simulink model "simulator_prototype_v2"  (R2021b)
(part 6 of 12)

t2408 = ct{941};
t2409 = ct{942};
t241 = ct{943};
t2410 = ct{944};
t2411 = ct{945};
t2412 = ct{946};
t2413 = ct{947};
t2414 = ct{948};
t2416 = ct{949};
t2417 = ct{950};
t2418 = ct{951};
t2419 = ct{952};
t2421 = ct{953};
t2422 = ct{954};
t2423 = ct{955};
t2425 = ct{956};
t2426 = ct{957};
t2427 = ct{958};
t2431 = ct{959};
t2432 = ct{960};
t2433 = ct{961};
t2434 = ct{962};
t2438 = ct{963};
t244 = ct{964};
t2440 = ct{965};
t2441 = ct{966};
t2444 = ct{967};
t2446 = ct{968};
t2447 = ct{969};
t2448 = ct{970};
t2449 = ct{971};
t2450 = ct{972};
t2451 = ct{973};
t2455 = ct{974};
t2457 = ct{975};
t2458 = ct{976};
t2459 = ct{977};
t2460 = ct{978};
t2461 = ct{979};
t2463 = ct{980};
t2465 = ct{981};
t2466 = ct{982};
t2467 = ct{983};
t2468 = ct{984};
t2470 = ct{985};
t2471 = ct{986};
t2472 = ct{987};
t2473 = ct{988};
t2474 = ct{989};
t2476 = ct{990};
t2477 = ct{991};
t2478 = ct{992};
t2479 = ct{993};
t2480 = ct{994};
t2481 = ct{995};
t2484 = ct{996};
t2485 = ct{997};
t2487 = ct{998};
t2488 = ct{999};
t2489 = ct{1000};
t2490 = ct{1001};
t2491 = ct{1002};
t2492 = ct{1003};
t2493 = ct{1004};
t2494 = ct{1005};
t2496 = ct{1006};
t2497 = ct{1007};
t2498 = ct{1008};
t2499 = ct{1009};
t25 = ct{1010};
t2500 = ct{1011};
t2502 = ct{1012};
t2503 = ct{1013};
t2504 = ct{1014};
t2505 = ct{1015};
t2507 = ct{1016};
t2508 = ct{1017};
t2509 = ct{1018};
t2510 = ct{1019};
t2511 = ct{1020};
t2512 = ct{1021};
t2514 = ct{1022};
t2515 = ct{1023};
t2516 = ct{1024};
t2517 = ct{1025};
t2520 = ct{1026};
t2521 = ct{1027};
t2522 = ct{1028};
t2524 = ct{1029};
t2525 = ct{1030};
t2526 = ct{1031};
t2527 = ct{1032};
t2528 = ct{1033};
t2529 = ct{1034};
t2530 = ct{1035};
t2531 = ct{1036};
t2532 = ct{1037};
t2534 = ct{1038};
t2535 = ct{1039};
t2539 = ct{1040};
t2541 = ct{1041};
t2542 = ct{1042};
t2548 = ct{1043};
t2549 = ct{1044};
t2550 = ct{1045};
t2552 = ct{1046};
t2554 = ct{1047};
t2555 = ct{1048};
t2556 = ct{1049};
t2557 = ct{1050};
t2558 = ct{1051};
t2559 = ct{1052};
t2560 = ct{1053};
t2564 = ct{1054};
t2565 = ct{1055};
t2566 = ct{1056};
t2569 = ct{1057};
t257 = ct{1058};
t2570 = ct{1059};
t2571 = ct{1060};
t2572 = ct{1061};
t2575 = ct{1062};
t2577 = ct{1063};
t2578 = ct{1064};
t2579 = ct{1065};
t2580 = ct{1066};
t2581 = ct{1067};
t2582 = ct{1068};
t2583 = ct{1069};
t2584 = ct{1070};
t2585 = ct{1071};
t2586 = ct{1072};
t2587 = ct{1073};
t2589 = ct{1074};
t259 = ct{1075};
t2595 = ct{1076};
t2597 = ct{1077};
t2599 = ct{1078};
t26 = ct{1079};
t2600 = ct{1080};
t2601 = ct{1081};
t2603 = ct{1082};
t2604 = ct{1083};
t2605 = ct{1084};
t2606 = ct{1085};
t261 = ct{1086};
t2610 = ct{1087};
t2611 = ct{1088};
t2612 = ct{1089};
t2613 = ct{1090};
t2614 = ct{1091};
t2616 = ct{1092};
t2618 = ct{1093};
t2619 = ct{1094};
t262 = ct{1095};
t2620 = ct{1096};
t2621 = ct{1097};
t2622 = ct{1098};
t2623 = ct{1099};
t2624 = ct{1100};
t2626 = ct{1101};
t2627 = ct{1102};
t2628 = ct{1103};
t2629 = ct{1104};
t2630 = ct{1105};
t2632 = ct{1106};
t2633 = ct{1107};
t2634 = ct{1108};
t2635 = ct{1109};
t2638 = ct{1110};
t264 = ct{1111};
t2640 = ct{1112};
t2641 = ct{1113};
t2642 = ct{1114};
t2643 = ct{1115};
t2644 = ct{1116};
t2645 = ct{1117};
t2646 = ct{1118};
t2647 = ct{1119};
t2648 = ct{1120};
t2649 = ct{1121};
t2650 = ct{1122};
t2651 = ct{1123};
t2652 = ct{1124};
t2653 = ct{1125};
t2654 = ct{1126};
t2655 = ct{1127};
t2657 = ct{1128};
t2658 = ct{1129};
t2659 = ct{1130};
t2660 = ct{1131};
t2661 = ct{1132};
t2662 = ct{1133};
t2664 = ct{1134};
t2665 = ct{1135};
t2666 = ct{1136};
t2667 = ct{1137};
t2668 = ct{1138};
t2670 = ct{1139};
t2671 = ct{1140};
t2672 = ct{1141};
t2673 = ct{1142};
t2674 = ct{1143};
t2675 = ct{1144};
t2676 = ct{1145};
t2678 = ct{1146};
t2679 = ct{1147};
t2680 = ct{1148};
t2681 = ct{1149};
t2682 = ct{1150};
t2683 = ct{1151};
t2684 = ct{1152};
t2685 = ct{1153};
t2686 = ct{1154};
t2687 = ct{1155};
t2688 = ct{1156};
t2691 = ct{1157};
t2692 = ct{1158};
t2694 = ct{1159};
t2695 = ct{1160};
t2697 = ct{1161};
t2698 = ct{1162};
t2699 = ct{1163};
t27 = ct{1164};
t2701 = ct{1165};
t2703 = ct{1166};
t2707 = ct{1167};
t2708 = ct{1168};
t2709 = ct{1169};
t271 = ct{1170};
t2710 = ct{1171};
t2711 = ct{1172};
t2712 = ct{1173};
t2714 = ct{1174};
t2716 = ct{1175};
t2732 = ct{1176};
t2733 = ct{1177};
t2735 = ct{1178};
t2736 = ct{1179};
t2737 = ct{1180};
t2738 = ct{1181};
t2739 = ct{1182};
t2740 = ct{1183};
t2742 = ct{1184};
t2743 = ct{1185};
t2744 = ct{1186};
t2745 = ct{1187};
t2748 = ct{1188};
t2749 = ct{1189};
t2750 = ct{1190};
t2753 = ct{1191};
t2754 = ct{1192};
t2757 = ct{1193};
t2759 = ct{1194};
t276 = ct{1195};
t2762 = ct{1196};
t2765 = ct{1197};
t2769 = ct{1198};
t2771 = ct{1199};
t2773 = ct{1200};
t2774 = ct{1201};
t2775 = ct{1202};
t2777 = ct{1203};
t2778 = ct{1204};
t2779 = ct{1205};
t2781 = ct{1206};
t2785 = ct{1207};
t2786 = ct{1208};
t2787 = ct{1209};
t2788 = ct{1210};
t279 = ct{1211};
t2790 = ct{1212};
t2791 = ct{1213};
t2792 = ct{1214};
t2793 = ct{1215};
t2795 = ct{1216};
t2796 = ct{1217};
t2797 = ct{1218};
t2798 = ct{1219};
t2799 = ct{1220};
t28 = ct{1221};
t280 = ct{1222};
t2801 = ct{1223};
t2802 = ct{1224};
t2803 = ct{1225};
t2804 = ct{1226};
t2805 = ct{1227};
t2806 = ct{1228};
t2807 = ct{1229};
t2808 = ct{1230};
t2810 = ct{1231};
t2811 = ct{1232};
t2812 = ct{1233};
t2813 = ct{1234};
t2814 = ct{1235};
t2817 = ct{1236};
t2818 = ct{1237};
t2819 = ct{1238};
t2820 = ct{1239};
t2823 = ct{1240};
t2825 = ct{1241};
t2831 = ct{1242};
t2832 = ct{1243};
t2835 = ct{1244};
t2838 = ct{1245};
t2850 = ct{1246};
t2851 = ct{1247};
t2857 = ct{1248};
t2858 = ct{1249};
t2859 = ct{1250};
t286 = ct{1251};
t2865 = ct{1252};
t2867 = ct{1253};
t2868 = ct{1254};
t2870 = ct{1255};
t2875 = ct{1256};
t2883 = ct{1257};
t2884 = ct{1258};
t2886 = ct{1259};
t2890 = ct{1260};
t2893 = ct{1261};
t2894 = ct{1262};
t2895 = ct{1263};
t2898 = ct{1264};
t2900 = ct{1265};
t2901 = ct{1266};
t2903 = ct{1267};
t2905 = ct{1268};
t2909 = ct{1269};
t2911 = ct{1270};
t2914 = ct{1271};
t2917 = ct{1272};
t2918 = ct{1273};
t2919 = ct{1274};
t2920 = ct{1275};
t2922 = ct{1276};
t2923 = ct{1277};
t2925 = ct{1278};
t2926 = ct{1279};
t2927 = ct{1280};
t293 = ct{1281};
t2930 = ct{1282};
t2931 = ct{1283};
t2933 = ct{1284};
t2935 = ct{1285};
t2937 = ct{1286};
t2941 = ct{1287};
t2942 = ct{1288};
t2943 = ct{1289};
t2944 = ct{1290};
t2947 = ct{1291};
t2948 = ct{1292};
t2949 = ct{1293};
t2950 = ct{1294};
t2951 = ct{1295};
t2952 = ct{1296};
t2955 = ct{1297};
t2956 = ct{1298};
t2961 = ct{1299};
t2962 = ct{1300};
t2963 = ct{1301};
t2964 = ct{1302};
t2965 = ct{1303};
t2966 = ct{1304};
t2969 = ct{1305};
t2970 = ct{1306};
t2971 = ct{1307};
t2972 = ct{1308};
t2973 = ct{1309};
t2975 = ct{1310};
t2976 = ct{1311};
t2977 = ct{1312};
t2978 = ct{1313};
t2979 = ct{1314};
t2981 = ct{1315};
t2982 = ct{1316};
t2983 = ct{1317};
t2984 = ct{1318};
t2986 = ct{1319};
t2987 = ct{1320};
t2990 = ct{1321};
t2991 = ct{1322};
t2993 = ct{1323};
t2999 = ct{1324};
t3 = ct{1325};
t30 = ct{1326};
t3000 = ct{1327};
t3004 = ct{1328};
t3005 = ct{1329};
t3008 = ct{1330};
t3010 = ct{1331};
t3011 = ct{1332};
t3012 = ct{1333};
t3015 = ct{1334};
t3017 = ct{1335};
t3018 = ct{1336};
t3019 = ct{1337};
t3022 = ct{1338};
t3023 = ct{1339};
t3026 = ct{1340};
t3027 = ct{1341};
t3029 = ct{1342};
t3030 = ct{1343};
t3036 = ct{1344};
t3037 = ct{1345};
t3042 = ct{1346};
t3043 = ct{1347};
t3044 = ct{1348};
t3045 = ct{1349};
t3049 = ct{1350};
t305 = ct{1351};
t3050 = ct{1352};
t3051 = ct{1353};
t3054 = ct{1354};
t3055 = ct{1355};
t3056 = ct{1356};
t306 = ct{1357};
t3064 = ct{1358};
t3065 = ct{1359};
t3066 = ct{1360};
t3067 = ct{1361};
t3068 = ct{1362};
t3069 = ct{1363};
t3072 = ct{1364};
t3074 = ct{1365};
t3075 = ct{1366};
t3076 = ct{1367};
t3077 = ct{1368};
t3079 = ct{1369};
t308 = ct{1370};
t3080 = ct{1371};
t3081 = ct{1372};
t3082 = ct{1373};
t3083 = ct{1374};
t3085 = ct{1375};
t3086 = ct{1376};
t3087 = ct{1377};
t3088 = ct{1378};
t31 = ct{1379};
t310 = ct{1380};
t3119 = ct{1381};
t312 = ct{1382};
t3120 = ct{1383};
t3129 = ct{1384};
t313 = ct{1385};
t314 = ct{1386};
t3153 = ct{1387};
t3154 = ct{1388};
t3159 = ct{1389};
t316 = ct{1390};
t3165 = ct{1391};
t3171 = ct{1392};
t3172 = ct{1393};
t319 = ct{1394};
t32 = ct{1395};
t321 = ct{1396};
t322 = ct{1397};
t326 = ct{1398};
t328 = ct{1399};
t329 = ct{1400};
t33 = ct{1401};
t330 = ct{1402};
t3306 = ct{1403};
t3308 = ct{1404};
t331 = ct{1405};
t3312 = ct{1406};
t3317 = ct{1407};
t332 = ct{1408};
t333 = ct{1409};
t335 = ct{1410};
t336 = ct{1411};
t3371 = ct{1412};
t3372 = ct{1413};
t3374 = ct{1414};
t3375 = ct{1415};
t338 = ct{1416};
t3380 = ct{1417};
t3381 = ct{1418};
t339 = ct{1419};
t34 = ct{1420};
t341 = ct{1421};
t343 = ct{1422};
t3457 = ct{1423};
t3458 = ct{1424};
t346 = ct{1425};
t347 = ct{1426};
t35 = ct{1427};
t350 = ct{1428};
t3504 = ct{1429};
t351 = ct{1430};
t3514 = ct{1431};
t352 = ct{1432};
t354 = ct{1433};
t356 = ct{1434};
t358 = ct{1435};
t359 = ct{1436};
t36 = ct{1437};
t360 = ct{1438};
t3617 = ct{1439};
t362 = ct{1440};
t3628 = ct{1441};
t363 = ct{1442};
t364 = ct{1443};
t365 = ct{1444};
t366 = ct{1445};
t369 = ct{1446};
t370 = ct{1447};
t371 = ct{1448};
t372 = ct{1449};
t3742 = ct{1450};
t378 = ct{1451};
t3780 = ct{1452};
t3781 = ct{1453};
t38 = ct{1454};
t380 = ct{1455};
t3808 = ct{1456};
t3809 = ct{1457};
t382 = ct{1458};
t3846 = ct{1459};
t3847 = ct{1460};
t3848 = ct{1461};
t3849 = ct{1462};
t3850 = ct{1463};
t387 = ct{1464};
t39 = ct{1465};
t393 = ct{1466};
t3940 = ct{1467};
t3961 = ct{1468};
t3999 = ct{1469};
t4 = ct{1470};
t410 = ct{1471};
t4109 = ct{1472};
t4115 = ct{1473};
t4116 = ct{1474};
t42 = ct{1475};
t4220 = ct{1476};
t4270 = ct{1477};
t428 = ct{1478};
t4280 = ct{1479};
t4282 = ct{1480};
t4289 = ct{1481};
t429 = ct{1482};
t4293 = ct{1483};
t4295 = ct{1484};
t43 = ct{1485};
t4421 = ct{1486};
t4500 = ct{1487};
t46 = ct{1488};
t461 = ct{1489};
t4620 = ct{1490};
t4644 = ct{1491};
t4655 = ct{1492};
t47 = ct{1493};
t4704 = ct{1494};
t4705 = ct{1495};
t473 = ct{1496};
t474 = ct{1497};
t4789 = ct{1498};
t4792 = ct{1499};
t480 = ct{1500};
t4974 = ct{1501};
t4976 = ct{1502};
t498 = ct{1503};
t4985 = ct{1504};
t5 = ct{1505};
t50 = ct{1506};
t503 = ct{1507};
t504 = ct{1508};
t506 = ct{1509};
t510 = ct{1510};
t514 = ct{1511};
t516 = ct{1512};
t521 = ct{1513};
t522 = ct{1514};
t523 = ct{1515};
t524 = ct{1516};
t5240 = ct{1517};
t5243 = ct{1518};
t528 = ct{1519};
t530 = ct{1520};
t5317 = ct{1521};
t535 = ct{1522};
t538 = ct{1523};
t5381 = ct{1524};
t539 = ct{1525};
t542 = ct{1526};
t543 = ct{1527};
t549 = ct{1528};
t56 = ct{1529};
t562 = ct{1530};
t563 = ct{1531};
t564 = ct{1532};
t573 = ct{1533};
t575 = ct{1534};
t577 = ct{1535};
t579 = ct{1536};
t58 = ct{1537};
t580 = ct{1538};
t581 = ct{1539};
t587 = ct{1540};
t59 = ct{1541};
t593 = ct{1542};
t594 = ct{1543};
t598 = ct{1544};
t6 = ct{1545};
t60 = ct{1546};
t610 = ct{1547};
t611 = ct{1548};
t612 = ct{1549};
t614 = ct{1550};
t615 = ct{1551};
t616 = ct{1552};
t623 = ct{1553};
t624 = ct{1554};
t628 = ct{1555};
t635 = ct{1556};
t636 = ct{1557};
t638 = ct{1558};
t640 = ct{1559};
t641 = ct{1560};
t642 = ct{1561};
t643 = ct{1562};
t644 = ct{1563};
t645 = ct{1564};
t646 = ct{1565};
t648 = ct{1566};
t649 = ct{1567};
t654 = ct{1568};
t655 = ct{1569};
t656 = ct{1570};
t657 = ct{1571};
t658 = ct{1572};
t659 = ct{1573};
t660 = ct{1574};
t662 = ct{1575};
t663 = ct{1576};
t664 = ct{1577};
t665 = ct{1578};
t666 = ct{1579};
t667 = ct{1580};
t668 = ct{1581};
t669 = ct{1582};
t67 = ct{1583};
t670 = ct{1584};
t672 = ct{1585};
t673 = ct{1586};
t674 = ct{1587};
t675 = ct{1588};
t676 = ct{1589};
t677 = ct{1590};
t678 = ct{1591};
t679 = ct{1592};
t68 = ct{1593};
t680 = ct{1594};
t681 = ct{1595};
t682 = ct{1596};
t683 = ct{1597};
t684 = ct{1598};
t685 = ct{1599};
t686 = ct{1600};
t687 = ct{1601};
t689 = ct{1602};
t691 = ct{1603};
t692 = ct{1604};
t693 = ct{1605};
t694 = ct{1606};
t696 = ct{1607};
t698 = ct{1608};
t7 = ct{1609};
t70 = ct{1610};
t702 = ct{1611};
t704 = ct{1612};
t705 = ct{1613};
t707 = ct{1614};
t708 = ct{1615};
t71 = ct{1616};
t710 = ct{1617};
t711 = ct{1618};
t712 = ct{1619};
t713 = ct{1620};
t714 = ct{1621};
t715 = ct{1622};
t716 = ct{1623};
t717 = ct{1624};
t718 = ct{1625};
t719 = ct{1626};
t720 = ct{1627};
t721 = ct{1628};
t722 = ct{1629};
t723 = ct{1630};
t724 = ct{1631};
t725 = ct{1632};
t726 = ct{1633};
t728 = ct{1634};
t73 = ct{1635};
t733 = ct{1636};
t736 = ct{1637};
t738 = ct{1638};
t740 = ct{1639};
t741 = ct{1640};
t742 = ct{1641};
t743 = ct{1642};
t744 = ct{1643};
t745 = ct{1644};
t746 = ct{1645};
t747 = ct{1646};
t749 = ct{1647};
t750 = ct{1648};
t751 = ct{1649};
t755 = ct{1650};
t756 = ct{1651};
t757 = ct{1652};
t758 = ct{1653};
t759 = ct{1654};
t76 = ct{1655};
t762 = ct{1656};
t763 = ct{1657};
t764 = ct{1658};
t766 = ct{1659};
t767 = ct{1660};
t768 = ct{1661};
t770 = ct{1662};
t771 = ct{1663};
t772 = ct{1664};
t773 = ct{1665};
t774 = ct{1666};
t775 = ct{1667};
t776 = ct{1668};
t777 = ct{1669};
t778 = ct{1670};
t781 = ct{1671};
t782 = ct{1672};
t783 = ct{1673};
t784 = ct{1674};
t785 = ct{1675};
t786 = ct{1676};
t787 = ct{1677};
t789 = ct{1678};
t790 = ct{1679};
t791 = ct{1680};
t792 = ct{1681};
t793 = ct{1682};
t794 = ct{1683};
t796 = ct{1684};
t797 = ct{1685};
t798 = ct{1686};
t799 = ct{1687};
t800 = ct{1688};
t801 = ct{1689};
t802 = ct{1690};
t806 = ct{1691};
t807 = ct{1692};
t808 = ct{1693};
t809 = ct{1694};
t812 = ct{1695};
t813 = ct{1696};
t816 = ct{1697};
t817 = ct{1698};
t818 = ct{1699};
t819 = ct{1700};
t820 = ct{1701};
t821 = ct{1702};
t822 = ct{1703};
t823 = ct{1704};
t824 = ct{1705};
t825 = ct{1706};
t826 = ct{1707};
t827 = ct{1708};
t828 = ct{1709};
t829 = ct{1710};
t830 = ct{1711};
t831 = ct{1712};
t832 = ct{1713};
t833 = ct{1714};
t850 = ct{1715};
t855 = ct{1716};
t856 = ct{1717};
t874 = ct{1718};
t878 = ct{1719};
t89 = ct{1720};
t893 = ct{1721};
t90 = ct{1722};
t91 = ct{1723};
t911 = ct{1724};
t92 = ct{1725};
t925 = ct{1726};
t926 = ct{1727};
t936 = ct{1728};
t937 = ct{1729};
t940 = ct{1730};
t941 = ct{1731};
t942 = ct{1732};
t944 = ct{1733};
t945 = ct{1734};
t948 = ct{1735};
t949 = ct{1736};
t950 = ct{1737};
t951 = ct{1738};
t959 = ct{1739};
t961 = ct{1740};
t965 = ct{1741};
t966 = ct{1742};
t97 = ct{1743};
t974 = ct{1744};
t978 = ct{1745};
t983 = ct{1746};
t987 = ct{1747};
t989 = ct{1748};
t99 = ct{1749};
t990 = ct{1750};
t991 = ct{1751};
t992 = ct{1752};
t993 = ct{1753};
t995 = ct{1754};
t996 = ct{1755};
t998 = ct{1756};
t3121 = t35.*t991.*t2699.*2.196325630278387e-1;
t3122 = t36.*t991.*t2699.*2.196325630278387e-1;
t3126 = t50.*t202.*t2981.*9.543032792050485e-17;
t3130 = (t2307.*t2363)./1.0e+8;
t3131 = (t2297.*t2388)./1.0e+8;
t3133 = t2363.*t2554;
t3136 = t38.*t1022.*(t855-t878).*(-2.196325630278387e-1);
t3137 = t39.*t1022.*(t855-t878).*(-2.196325630278387e-1);
t3139 = (t2297.*t2419)./1.0e+8;
t3140 = (t2338.*t2363)./1.0e+8;
t3143 = t35.*t991.*t2699.*1.122398993609262e-1;
t3144 = t36.*t991.*t2699.*1.122398993609262e-1;
t3147 = t35.*t991.*t2699.*1.887873611596568e-1;
t3148 = t36.*t991.*t2699.*1.887873611596568e-1;
t3149 = t35.*t991.*t2699.*5.076068728976717e-3;
t3150 = t36.*t991.*t2699.*5.076068728976717e-3;
t3156 = t2307.*t2363.*6.2e-7;
t3157 = t2297.*t2388.*6.2e-7;
t3158 = t2363.*t2801;
t3162 = t2297.*t2419.*6.2e-7;
t3163 = t2338.*t2363.*6.2e-7;
t3164 = t2363.*t2831;
t3167 = t38.*t1022.*(t855-t878).*(-1.122398993609262e-1);
t3168 = t39.*t1022.*(t855-t878).*(-1.122398993609262e-1);
t3169 = t2363.*t2850;
t3170 = t2363.*t2851;
t3173 = t38.*t1022.*(t855-t878).*(-1.887873611596568e-1);
t3174 = t39.*t1022.*(t855-t878).*(-1.887873611596568e-1);
t3175 = t39.*t1022.*(t855-t878).*1.887873611596568e-1;
t3176 = t38.*t1022.*(t855-t878).*(-5.076068728976717e-3);
t3177 = t39.*t1022.*(t855-t878).*(-5.076068728976717e-3);
t3178 = t38.*t1022.*(t855-t878).*5.076068728976717e-3;
t3179 = t39.*t1022.*(t855-t878).*5.076068728976717e-3;
t3181 = t2363.*t2973;
t3182 = t2388.*t2971;
t3183 = t2388.*t2972;
t3185 = t2388.*t2973;
t3192 = t2399.*t2973;
t3200 = t2363.*t2976;
t3203 = t38.*t1022.*(t855-t878).*(-1.46680315462752e-4);
t3204 = t39.*t1022.*(t855-t878).*(-1.46680315462752e-4);
t3205 = t39.*t1022.*(t855-t878).*1.46680315462752e-4;
t3206 = t598+t1904+t2554;
t3267 = t35.*t941.*t948.*(t850-t874).*(-4.392651260556773e-1);
t3268 = t36.*t941.*t948.*(t850-t874).*(-4.392651260556773e-1);
t3269 = t35.*t941.*t948.*(t850-t874).*4.392651260556773e-1;
t3270 = t36.*t941.*t948.*(t850-t874).*4.392651260556773e-1;
t3311 = t201.*t3165.*8.595599785252598e-1;
t3313 = t535+t577+t1887+t1940;
t3359 = t564+t611+t1929+t1967;
t3361 = t35.*t941.*t948.*(t850-t874).*(-2.244797987218524e-1);
t3362 = t36.*t941.*t948.*(t850-t874).*(-2.244797987218524e-1);
t3363 = t36.*t941.*t948.*(t850-t874).*(-3.775747223193135e-1);
t3364 = t35.*t941.*t948.*(t850-t874).*(-3.775747223193135e-1);
t3365 = t36.*t941.*t948.*(t850-t874).*3.775747223193135e-1;
t3367 = t35.*t941.*t948.*(t850-t874).*(-1.015213745795343e-2);
t3368 = t36.*t941.*t948.*(t850-t874).*(-1.015213745795343e-2);
t3369 = t35.*t941.*t948.*(t850-t874).*1.015213745795343e-2;
t3370 = t36.*t941.*t948.*(t850-t874).*1.015213745795343e-2;
t3378 = -t3375;
t3383 = -t3380;
t3384 = -t3381;
t3416 = t50.*t202.*t3165.*9.543032792050485e-17;
t3459 = -t3458;
t3469 = t2363.*t3154;
t3470 = t2388.*t3154;
t3472 = t2419.*t3154;
t3480 = t998+t1036+t1059+t1481+t1519;
t3498 = t1019+t1060+t1072+t1503+t1537;
t3779 = t1021+t1024+t1053+t1490+t1498+t1512;
t3783 = t1582+t1647+t1769+t1961+t2034;
t3851 = t1619+t1739+t1774+t1991+t2057+t2079;
t3865 = t58+t59+t3849;
t3866 = t56+t73+t3850;
t3869 = t539+t577+t581+t593+t1909+t1937+t1939+t1940;
t3870 = t538+t573+t575+t579+t1924+t1935+t1936+t1957;
t3871 = t1038+t1043+t1056+t1057+t1501+t1507+t1517+t1531;
t3911 = -t26.*(t1941-t3308+t39.*t1022.*(t855-t878).*2.196325630278387e-1);
t3912 = -t32.*(t1941-t3308+t39.*t1022.*(t855-t878).*2.196325630278387e-1);
t3914 = -t27.*(t1959-t3306+t38.*t1022.*(t855-t878).*2.196325630278387e-1);
t3915 = -t33.*(t1959-t3306+t38.*t1022.*(t855-t878).*2.196325630278387e-1);
t3917 = t27.*(t1959-t3306+t38.*t1022.*(t855-t878).*2.196325630278387e-1).*(-3.0./5.0e+2);
t3948 = t33.*(t1959-t3306+t38.*t1022.*(t855-t878).*2.196325630278387e-1).*(-1.247162e-2);
t3955 = t26.*(t1941-t3308+t39.*t1022.*(t855-t878).*2.196325630278387e-1).*(-5.84482e-3);
t3956 = t33.*(t1959-t3306+t38.*t1022.*(t855-t878).*2.196325630278387e-1).*1.247162e-2;
t3960 = t26.*(t1941-t3308+t39.*t1022.*(t855-t878).*2.196325630278387e-1).*(-6.48e-5);
t3966 = t27.*(t1959-t3306+t38.*t1022.*(t855-t878).*2.196325630278387e-1).*(-3.131399999999998e-4);
t3969 = t32.*(t1941-t3308+t39.*t1022.*(t855-t878).*2.196325630278387e-1).*(-6.47e-6);
t3970 = t27.*(t1959-t3306+t38.*t1022.*(t855-t878).*2.196325630278387e-1).*(-4.36041e-5);
t3971 = t32.*(t1941-t3308+t39.*t1022.*(t855-t878).*2.196325630278387e-1).*6.47e-6;
t3974 = t1000+t1002+t1006+t1028+t1040+t1054+t1493+t1500+t1506;
t4002 = t26.*(t1941-t3308+t39.*t1022.*(t855-t878).*2.196325630278387e-1).*(-1.688944904408e-4);
t4003 = t27.*(t1959-t3306+t38.*t1022.*(t855-t878).*2.196325630278387e-1).*(-6.1855407534e-5);
t4005 = t33.*(t1959-t3306+t38.*t1022.*(t855-t878).*2.196325630278387e-1).*(-1.35652563578e-4);
t4006 = t26.*(t1941-t3308+t39.*t1022.*(t855-t878).*2.196325630278387e-1).*1.688944904408e-4;
t4012 = t26.*(t1941-t3308+t39.*t1022.*(t855-t878).*2.196325630278387e-1).*(-7.0482312e-7);
t4017 = t32.*(t1941-t3308+t39.*t1022.*(t855-t878).*2.196325630278387e-1).*(-1.869599668e-7);
t4019 = t26.*(t1941-t3308+t39.*t1022.*(t855-t878).*2.196325630278387e-1).*7.0482312e-7;
t4129 = -t34.*(t1005+t26.*(t1941-t3308+t39.*t1022.*(t855-t878).*2.196325630278387e-1));
t4132 = -t28.*(t1005+t26.*(t1941-t3308+t39.*t1022.*(t855-t878).*2.196325630278387e-1));
t4139 = t28.*(t1005+t26.*(t1941-t3308+t39.*t1022.*(t855-t878).*2.196325630278387e-1));
t4182 = t34.*(t1005+t26.*(t1941-t3308+t39.*t1022.*(t855-t878).*2.196325630278387e-1)).*(-1.838876e-2);
t4192 = t50.*t189.*(t1941-t3308+t39.*t1022.*(t855-t878).*2.196325630278387e-1).*(-4.306286555174926e-24);
t4194 = t50.*t189.*(t1959-t3306+t38.*t1022.*(t855-t878).*2.196325630278387e-1).*(-7.660522649005482e-24);
t4214 = t34.*(t1005+t26.*(t1941-t3308+t39.*t1022.*(t855-t878).*2.196325630278387e-1)).*(-1.33637554986e-4);
t4230 = t1098+t1129+t1142+t1156+t2455+t2484+t2490+t2524;
t4231 = t1099+t1135+t1160+t1169+t2451+t2457+t2511+t2512;
t4232 = t1699+t1745+t1767+t1768+t2039+t2093+t2095+t2107;
t4269 = t312+t316+t4115;
t4271 = t314+t319+t4116;
t4279 = t1593+t1621+t1625+t1632+t1743+t1778+t1997+t2035+t2094;
t4281 = t1592+t1603+t1610+t1875+t1883+t1891+t1910+t1925+t1934;
t4300 = -t3165.*(t1959-t3306+t38.*t1022.*(t855-t878).*2.196325630278387e-1);
t4301 = t99+t107+t108+t124+t130+t139+t280+t286+t305+t310+t614+t623+t624+t658+t698+t767+t993+t995+t1011+t1033;
t4303 = t216+t230+t261+t276+t474+t480+t503+t510+t926+t936+t961+t987+t1432+t1439+t1464+t1465;
t4325 = t100+t101+t126+t128+t134+t257+t279+t293+t306+t308+t615+t616+t662+t696+t733+t978+t990+t992+t1034+t1037;
t4368 = -t3154.*(t1005+t26.*(t1941-t3308+t39.*t1022.*(t855-t878).*2.196325630278387e-1));
t4371 = t3154.*(t1005+t26.*(t1941-t3308+t39.*t1022.*(t855-t878).*2.196325630278387e-1));
t4444 = t2143+t2161+t2163+t2340+t2409+t2411+t2425+t2485+t2489;
t4445 = t1444+t1462+t1476+t1487+t1489+t1495+t1534+t1540+t1850+t1857+t1867+t1869;
t4589 = t680+t942+t965+t1103+t1133+t1200+t1211+t1510+t1551+t1555+t1556+t1557+t1574+t1575;
t4599 = t3808.*t3847;
t4601 = t3809.*t3848;
t4641 = t3780.*t4109;
t4643 = -t3781.*(t1089-t1104-t1105-t1121-t2117+t2120+t2122+t2123);
t4645 = t3781.*(t1089-t1104-t1105-t1121-t2117+t2120+t2122+t2123);
t4646 = t925+t1331+t1372+t1453+t1457+t1472+t1502+t1508+t1786+t1801+t1803+t1818+t1856+t1858;
t4668 = -t3781.*(t313-t314-t1108+t1115-t1158-t1159-t2117+t2120+t2122+t2123);
t4669 = t3781.*(t313-t314-t1108+t1115-t1158-t1159-t2117+t2120+t2122+t2123);
t4679 = t3847.*t4116;
t4680 = t3848.*t4115;
t4823 = -t3847.*(t313-t314-t1108+t1115-t1158-t1159-t2117+t2120+t2122+t2123);
t4834 = -t3849.*(t313-t314-t1108+t1115-t1158-t1159-t2117+t2120+t2122+t2123);
t4842 = t3849.*(t313-t314-t1108+t1115-t1158-t1159-t2117+t2120+t2122+t2123);
t4986 = t151+t182+t203+t231+t239+t259+t271+t393+t428+t461+t473+t498+t504+t506+t856+t893+t911+t937+t940+t959+t966+t1195+t1266+t1377+t1388+t1431+t1466+t1467;
t5223 = t704+t705+t726+t728+t755+t778+t781+t797+t1670+t1675+t1713+t1714+t1718+t1719+t1733+t1734+t1988+t1990+t2009+t2010+t2017+t2027+t2036+t2074;
t5224 = t719+t742+t747+t750+t751+t763+t773+t775+t1642+t1655+t1657+t1662+t1663+t1684+t1709+t1724+t1984+t2005+t2031+t2033+t2052+t2059+t2067+t2068;
t5227 = t236.*t241.*t3999.*t4644.*2.33806891548878e-94;
t5252 = t236.*t241.*t3940.*t4655.*2.33806891548878e-94;
t5253 = t236.*t241.*t3961.*t4655.*4.788365138921021e-91;
t5306 = t236.*t241.*t4270.*t4644.*4.312975891071717e-75;
t5308 = t236.*t241.*t4220.*t4655.*4.312975891071717e-75;
t5315 = t236.*t241.*t3999.*t4705.*2.595777943136013e-110;
t5319 = t236.*t241.*t3961.*t4792.*5.316153227542554e-107;
t5328 = t236.*t241.*t4289.*t4644.*4.788365138921021e-91;
t5337 = t236.*t241.*t4280.*t4655.*4.788365138921021e-91;
t5340 = t236.*t241.*t4282.*t4655.*4.312975891071717e-75;
t5347 = t236.*t241.*t4270.*t4705.*4.788365138921021e-91;
t5348 = t236.*t241.*t4295.*t4655.*4.312975891071717e-75;
t5350 = t236.*t241.*t4293.*t4655.*2.33806891548878e-94;
t5377 = t236.*t241.*t4289.*t4705.*5.316153227542554e-107;
t5378 = t236.*t241.*t3999.*t4974.*1.267469698796881e-113;
t5379 = t236.*t241.*t4280.*t4792.*5.316153227542554e-107;
t5384 = t236.*t241.*t4282.*t4792.*4.788365138921021e-91;
t5398 = t236.*t241.*t3940.*t4985.*1.267469698796881e-113;
t5403 = t236.*t241.*t3961.*t4985.*2.595777943136013e-110;
t5406 = t236.*t241.*t4295.*t4792.*4.788365138921021e-91;
t5410 = t236.*t241.*t4293.*t4792.*2.595777943136013e-110;
t5427 = t236.*t241.*t4270.*t4974.*2.33806891548878e-94;
t5443 = t236.*t241.*t4220.*t4985.*2.33806891548878e-94;
t5485 = t1305+t1307+t1316+t1317+t1342+t1399+t1404+t1436+t2184+t2202+t2207+t2258+t2274+t2275+t2277+t2278+t2541+t2560+t2589+t2595+t2597+t2623+t2624+t2634;
t5486 = t1300+t1311+t1337+t1338+t1379+t1392+t1394+t1398+t2179+t2181+t2200+t2201+t2232+t2241+t2271+t2276+t2580+t2582+t2587+t2611+t2629+t2630+t2655+t2662;
t5487 = t236.*t241.*t4421.*t4792.*5.316153227542554e-107;
t5490 = t236.*t241.*t4289.*t4974.*2.595777943136013e-110;
t5491 = t236.*t241.*t4500.*t4792.*4.788365138921021e-91;
t5494 = t236.*t241.*t4282.*t4985.*2.33806891548878e-94;
t5500 = t236.*t241.*t4293.*t4985.*1.267469698796881e-113;
t5518 = t236.*t241.*t4620.*t4792.*2.595777943136013e-110;
t5524 = t236.*t241.*t4655.*t4704.*4.788365138921021e-91;
t5549 = t236.*t241.*t4421.*t4985.*2.595777943136013e-110;
t5578 = t236.*t241.*t4500.*t4985.*2.33806891548878e-94;
t5626 = t236.*t241.*t4620.*t4985.*1.267469698796881e-113;
t5630 = t236.*t241.*t4655.*t4976.*2.33806891548878e-94;
t5692 = t236.*t241.*t4792.*t4976.*2.595777943136013e-110;
t5695 = t236.*t241.*t4704.*t4985.*2.595777943136013e-110;
t5722 = t1076+t1078+t1079+t1097+t1119+t1120+t1125+t1127+t1128+t1136+t1140+t1144+t1152+t1153+t1164+t1175+t2417+t2418+t2426+t2431+t2432+t2444+t2466+t2467+t2476+t2477+t2480+t2481+t2491+t2505+t2514+t2516;
t5723 = t1074+t1075+t1077+t1088+t1109+t1111+t1116+t1130+t1131+t1138+t1139+t1151+t1163+t1165+t1172+t1173+t2416+t2427+t2440+t2441+t2446+t2458+t2463+t2473+t2474+t2478+t2479+t2487+t2488+t2498+t2499+t2504;
t5839 = t1811+t1812+t1821+t1822+t1823+t1824+t1825+t1830+t1837+t1838+t1839+t1846+t1851+t1852+t1855+t1859+t2858+t2859+t2867+t2868+t2886+t2894+t2895+t2903+t2905+t2914+t2919+t2922+t2923+t2925+t2933+t2935;
t5840 = t1808+t1809+t1816+t1819+t1820+t1831+t1832+t1833+t1841+t1844+t1845+t1847+t1848+t1849+t1853+t1854+t2857+t2865+t2883+t2884+t2890+t2893+t2898+t2900+t2901+t2911+t2917+t2918+t2920+t2926+t2930+t2931;
t5951 = t711+t714+t743+t759+t771+t772+t783+t784+t789+t798+t816+t817+t820+t823+t824+t827+t1634+t1645+t1646+t1680+t1696+t1697+t1707+t1708+t1720+t1723+t1731+t1732+t1762+t1779+t1781+t1787+t1979+t1980+t1999+t2001+t2043+t2058+t2061+t2062+t2065+t2066+t2081+t2082+t2084+t2102+t2108+t2109;
t5953 = t720+t723+t744+t764+t774+t776+t785+t786+t794+t800+t806+t807+t809+t812+t831+t832+t1639+t1656+t1658+t1685+t1710+t1711+t1725+t1728+t1735+t1736+t1747+t1748+t1764+t1770+t1783+t1792+t1983+t2008+t2015+t2016+t2030+t2032+t2041+t2042+t2051+t2054+t2070+t2071+t2091+t2103+t2106+t2110;
t5954 = t712+t713+t757+t758+t766+t770+t782+t790+t791+t799+t818+t822+t825+t826+t828+t829+t1644+t1677+t1679+t1687+t1698+t1706+t1721+t1722+t1729+t1730+t1744+t1760+t1761+t1763+t1788+t1789+t1981+t2002+t2003+t2013+t2037+t2044+t2045+t2063+t2064+t2075+t2083+t2085+t2086+t2100+t2101+t2105;
t5955 = t721+t722+t745+t746+t749+t777+t787+t792+t793+t796+t801+t802+t808+t819+t830+t833+t1629+t1640+t1641+t1659+t1661+t1712+t1715+t1726+t1727+t1737+t1746+t1755+t1784+t1785+t1790+t1791+t1985+t2006+t2007+t2014+t2029+t2040+t2049+t2050+t2069+t2072+t2087+t2089+t2090+t2104+t2111+t2112;
t6183 = t1285+t1299+t1324+t1343+t1352+t1366+t1367+t1376+t1386+t1387+t1389+t1407+t1408+t1417+t1428+t1429+t2177+t2178+t2190+t2191+t2198+t2210+t2211+t2230+t2234+t2261+t2265+t2266+t2267+t2283+t2285+t2288+t2548+t2549+t2565+t2566+t2599+t2616+t2620+t2621+t2628+t2641+t2645+t2646+t2648+t2657+t2661+t2668;
t6184 = t1290+t1301+t1328+t1335+t1349+t1380+t1393+t1395+t1397+t1409+t1410+t1419+t1420+t1421+t1433+t1434+t2180+t2182+t2217+t2218+t2233+t2238+t2242+t2243+t2249+t2254+t2263+t2268+t2269+t2272+t2284+t2289+t2557+t2558+t2570+t2571+t2579+t2581+t2584+t2585+t2586+t2614+t2633+t2644+t2653+t2654+t2660+t2665;
t6185 = t1286+t1287+t1322+t1323+t1354+t1368+t1374+t1375+t1385+t1406+t1414+t1415+t1416+t1427+t1441+t1448+t2176+t2192+t2209+t2216+t2224+t2227+t2229+t2237+t2259+t2260+t2264+t2273+t2281+t2282+t2286+t2287+t2550+t2552+t2564+t2577+t2578+t2600+t2601+t2622+t2626+t2627+t2635+t2642+t2643+t2647+t2649+t2650;
t6187 = t1319+t1320+t1344+t1345+t1348+t1360+t1370+t1371+t1378+t1405+t1411+t1412+t1424+t1425+t1440+t1447+t2174+t2187+t2194+t2195+t2203+t2208+t2215+t2222+t2223+t2248+t2256+t2257+t2262+t2270+t2279+t2280+t2542+t2559+t2569+t2603+t2604+t2605+t2606+t2610+t2618+t2619+t2632+t2640+t2658+t2659+t2666+t2667;
t2424 = -t2376;
t2445 = -t2387;
t2501 = t2350.*(3.0./5.0e+2);
t2506 = t2355.*(3.0./5.0e+2);
t2523 = t2390.*(3.0./5.0e+2);
t2533 = -t2521;
t2536 = -t2527;
t2537 = -t2528;
t2547 = t2496.*(3.0./5.0e+2);
t2553 = t2502.*(3.0./5.0e+2);
t2602 = t2350./1.0e+8;
t2615 = t2355./1.0e+8;
t2636 = t2522.*(3.0./5.0e+2);
t2663 = t2387./1.0e+8;
t2677 = -t2674;
t2689 = -t2681;
t2690 = -t2684;
t2693 = -t2687;
t2696 = -t2688;
t2700 = -t2692;
t2702 = -t2694;
t2704 = -t2697;
t2705 = -t2698;
t2713 = -t2707;
t2715 = -t2709;
t2717 = -t2710;
t2719 = -t2711;
t2720 = -t2712;
t2721 = -t2714;
t2746 = t2351.*9.99471e-3;
t2747 = -t2737;
t2751 = t2356.*1.838876e-2;
t2752 = -t2740;
t2755 = t2350.*1.247162e-2;
t2756 = t2355.*1.247162e-2;
t2760 = t2387.*1.247162e-2;
t2761 = t2376.*9.99471e-3;
t2764 = t2373.*1.838876e-2;
t2768 = t2350.*5.68686e-3;
t2770 = t2355.*5.68686e-3;
t2776 = t2390.*5.68686e-3;
t2784 = t2410.*9.99471e-3;
t2789 = t2412.*1.838876e-2;
t2815 = t2350.*3.131399999999998e-4;
t2816 = t2355.*3.131399999999998e-4;
t2821 = t2350.*5.7e-7;
t2822 = t2390.*3.131399999999998e-4;
t2824 = t2355.*5.7e-7;
t2826 = t2351.*9.3e-7;
t2827 = t2350.*1.02e-6;
t2828 = t2355.*1.02e-6;
t2829 = t2356.*1.02e-6;
t2830 = -t2813;
t2833 = t2497.*9.99471e-3;
t2834 = -t2817;
t2836 = t2503.*1.838876e-2;
t2837 = -t2820;
t2839 = t2373.*1.02e-6;
t2840 = t2376.*9.3e-7;
t2843 = t2350.*2.4e-7;
t2844 = t2496.*1.247162e-2;
t2845 = t2390.*5.7e-7;
t2846 = t2355.*2.4e-7;
t2847 = t2502.*1.247162e-2;
t2848 = t2387.*1.02e-6;
t2852 = t2521.*1.247162e-2;
t2854 = t2351.*9.0e-8;
t2855 = t2356.*9.0e-8;
t2856 = -t2838;
t2861 = t2410.*9.3e-7;
t2864 = t2412.*1.02e-6;
t2866 = t2496.*5.68686e-3;
t2869 = t2502.*5.68686e-3;
t2871 = t2350.*4.0e-8;
t2873 = t2387.*2.4e-7;
t2874 = t2355.*4.0e-8;
t2877 = t2373.*9.0e-8;
t2878 = t2376.*9.0e-8;
t2881 = t2522.*5.68686e-3;
t2882 = t2387.*4.0e-8;
t2885 = t2390.*4.0e-8;
t2888 = t2527.*9.99471e-3;
t2889 = t2528.*9.99471e-3;
t2897 = t2526.*1.838876e-2;
t2902 = t2531.*1.838876e-2;
t2928 = t2410.*9.0e-8;
t2929 = t2412.*9.0e-8;
t2932 = t2496.*3.131399999999998e-4;
t2934 = t2502.*3.131399999999998e-4;
t2936 = t2522.*3.131399999999998e-4;
t2945 = -t2943;
t2946 = -t2944;
t2953 = -t2947;
t2954 = -t2949;
t2957 = -t2952;
t2985 = -t2983;
t2992 = t514+t2390;
t2998 = t521+t2522;
t3001 = -t2999;
t3002 = -t3000;
t3006 = -t3005;
t3013 = -t3011;
t3014 = -t3012;
t3016 = -t3015;
t3024 = -t3022;
t3025 = -t3023;
t3028 = -t3026;
t3031 = -t3030;
t3038 = -t3036;
t3039 = -t3037;
t3046 = -t3042;
t3047 = t1458+t2350;
t3048 = t1471+t2355;
t3052 = -t18.*(t1456-t2355);
t3053 = -t23.*(t1456-t2355);
t3057 = t1478+t2496;
t3058 = t1485+t2502;
t3059 = -t28.*(t1477-t2502);
t3060 = -t34.*(t1477-t2502);
t3061 = t28.*(t1477-t2502);
t3073 = -t3067;
t3078 = -t3072;
t3091 = t18.*(t1456-t2355).*(-9.99471e-3);
t3092 = t23.*(t1456-t2355).*(-9.99471e-3);
t3093 = t18.*(t1456-t2355).*(-1.838876e-2);
t3094 = t23.*(t1456-t2355).*(-1.838876e-2);
t3095 = t18.*(t1456-t2355).*9.99471e-3;
t3096 = t23.*(t1456-t2355).*9.99471e-3;
t3097 = t18.*(t1456-t2355).*1.838876e-2;
t3100 = t18.*(t1456-t2355).*(-9.3e-7);
t3101 = t18.*(t1456-t2355).*(-1.02e-6);
t3102 = t23.*(t1456-t2355).*(-9.3e-7);
t3103 = t23.*(t1456-t2355).*(-1.02e-6);
t3106 = t18.*(t1456-t2355).*9.3e-7;
t3107 = t18.*(t1456-t2355).*(-9.0e-8);
t3108 = t23.*(t1456-t2355).*(-9.0e-8);
t3109 = t18.*(t1456-t2355).*9.0e-8;
t3113 = t34.*(t1477-t2502).*(-9.99471e-3);
t3115 = t34.*(t1477-t2502).*(-1.838876e-2);
t3117 = t34.*(t1477-t2502).*9.99471e-3;
t3123 = t2356+t2373;
t3124 = -t3121;
t3125 = -t3122;
t3128 = -t3126;
t3134 = -t3130;
t3135 = -t3131;
t3141 = t2503+t2526;
t3145 = -t3143;
t3146 = -t3144;
t3151 = -t3147;
t3152 = -t3149;
t3160 = -t3156;
t3161 = -t3157;
t3187 = t201.*(t1456-t2355).*(-4.899491877593981e-7);
t3189 = -t3181;
t3190 = -t3182;
t3195 = t201.*(t1456-t2355).*(-3.438239914101039e-8);
t3198 = t201.*(t1456-t2355).*3.438239914101039e-8;
t3202 = -t3200;
t3207 = t2825+t2850;
t3208 = t2133+t3000;
t3209 = t2134+t2999;
t3213 = t50.*t202.*(t1456-t2355).*(-9.543032792050485e-25);
t3218 = t50.*t202.*(t1456-t2355).*9.543032792050485e-25;
t3228 = t2171+t3011;
t3229 = t2172+t3012;
t3255 = t50.*t202.*(t1456-t2355).*(-9.733893447891495e-23);
t3257 = t50.*t202.*(t1456-t2355).*(-5.439528691468777e-23);
t3259 = t50.*t202.*(t1456-t2355).*9.733893447891495e-23;
t3261 = t50.*t202.*(t1456-t2355).*(-2.290327870092116e-23);
t3262 = t50.*t202.*(t1456-t2355).*5.439528691468777e-23;
t3263 = t50.*t202.*(t1456-t2355).*(-3.817213116820194e-24);
t3266 = t50.*t202.*(t1456-t2355).*3.817213116820194e-24;
t3314 = t50.*t202.*t3120.*9.543032792050485e-17;
t3377 = t2363.*(t1456-t2355).*(-1.0e-8);
t3418 = -t3416;
t3424 = t2363.*(t1456-t2355).*(-5.7e-7);
t3427 = t2363.*(t1456-t2355).*(-1.02e-6);
t3431 = t2388.*(t1456-t2355).*(-5.7e-7);
t3432 = t2363.*(t1456-t2355).*5.7e-7;
t3436 = t2363.*(t1456-t2355).*(-2.4e-7);
t3438 = t2388.*(t1456-t2355).*5.7e-7;
t3443 = t2363.*(t1456-t2355).*(-4.0e-8);
t3448 = t2419.*(t1456-t2355).*(-5.7e-7);
t3449 = t2388.*(t1456-t2355).*(-4.0e-8);
t3450 = t2363.*(t1456-t2355).*4.0e-8;
t3453 = t2419.*(t1456-t2355).*5.7e-7;
t3454 = t2419.*(t1456-t2355).*(-4.0e-8);
t3456 = t2419.*(t1456-t2355).*4.0e-8;
t3460 = t2363.*t3119;
t3471 = -t3470;
t3474 = -t3472;
t3526 = t201.*(t2337+t18.*(t1456-t2355)).*(-8.76751178095765e-7);
t3533 = t201.*(t2337+t18.*(t1456-t2355)).*(-7.736039806727338e-8);
t3560 = t2363.*t3206;
t3599 = t347+t1539+t2831+t2875;
t3668 = t50.*t202.*(t2337+t18.*(t1456-t2355)).*(-8.875020496606951e-23);
t3670 = t50.*t202.*(t2337+t18.*(t1456-t2355)).*8.875020496606951e-23;
t3671 = t50.*t202.*(t2337+t18.*(t1456-t2355)).*(-9.733893447891495e-23);
t3673 = t50.*t202.*(t2337+t18.*(t1456-t2355)).*9.733893447891495e-23;
t3675 = t50.*t202.*(t2337+t18.*(t1456-t2355)).*(-8.588729512845436e-24);
t3676 = t50.*t202.*(t2337+t18.*(t1456-t2355)).*8.588729512845436e-24;
t3689 = t530+t1918+t2743+t2771;
t3732 = t563+t1964+t2832+t2870;
t3750 = t2363.*(t2337+t18.*(t1456-t2355)).*(-9.3e-7);
t3751 = t2363.*(t2337+t18.*(t1456-t2355)).*(-1.02e-6);
t3753 = t2363.*(t2337+t18.*(t1456-t2355)).*9.3e-7;
t3754 = t2388.*(t2337+t18.*(t1456-t2355)).*(-1.02e-6);
t3758 = t2363.*(t2337+t18.*(t1456-t2355)).*(-9.0e-8);
t3759 = t2388.*(t2337+t18.*(t1456-t2355)).*1.02e-6;
t3761 = t2388.*(t2337+t18.*(t1456-t2355)).*(-9.0e-8);
t3762 = t2363.*(t2337+t18.*(t1456-t2355)).*9.0e-8;
t3767 = t2419.*(t2337+t18.*(t1456-t2355)).*(-1.02e-6);
t3768 = t2388.*(t2337+t18.*(t1456-t2355)).*9.0e-8;
t3770 = t2419.*(t2337+t18.*(t1456-t2355)).*1.02e-6;
t3774 = t2419.*(t2337+t18.*(t1456-t2355)).*(-9.0e-8);
t3776 = t2419.*(t2337+t18.*(t1456-t2355)).*9.0e-8;
t3786 = (t1477-t2502).*(t2801-t2850);
t3827 = (t2337+t18.*(t1456-t2355)).*(t1477-t2502).*1.02e-6;
t3834 = (t2337+t18.*(t1456-t2355)).*(t1477-t2502).*9.0e-8;
t3880 = t1880+t3122+t3270;
t3882 = t1902+t3121+t3269;
t3883 = -t16.*(-t1881+t3121+t3269);
t3885 = -t21.*(-t1881+t3121+t3269);
t3888 = -t17.*(-t1901+t3122+t3270);
t3890 = -t22.*(-t1901+t3122+t3270);
t3894 = t17.*(-t1901+t3122+t3270).*(-3.0./5.0e+2);
t3898 = t1943+t3136+t3306;
t3903 = t1955+t3137+t3308;
t3904 = t1958+t3137+t3308;
t3905 = t1972+t3136+t3306;
t3923 = t22.*(-t1901+t3122+t3270).*(-1.247162e-2);
t3924 = t16.*(-t1881+t3121+t3269).*(-5.84482e-3);
t3928 = t22.*(-t1901+t3122+t3270).*1.247162e-2;
t3930 = t17.*(-t1901+t3122+t3270).*(-5.68686e-3);
t3931 = t16.*(-t1881+t3121+t3269).*(-6.48e-5);
t3932 = t16.*(-t1881+t3121+t3269).*5.84482e-3;
t3934 = t16.*(-t1881+t3121+t3269).*6.48e-5;
t3935 = t21.*(-t1881+t3121+t3269).*(-6.47e-6);
t3938 = t17.*(-t1901+t3122+t3270).*(-3.131399999999998e-4);
t4092 = -t17.*((t237.*(t42-t43))./9.007199254740992e+15+t21.*(-t1881+t3121+t3269));
t4094 = -t22.*((t237.*(t42-t43))./9.007199254740992e+15+t21.*(-t1881+t3121+t3269));
t4099 = -t18.*(t951+t16.*(-t1881+t3121+t3269));
t4100 = -t23.*(t951+t16.*(-t1881+t3121+t3269));
t4103 = t22.*((t237.*(t42-t43))./9.007199254740992e+15+t21.*(-t1881+t3121+t3269));
t4104 = t23.*(t951+t16.*(-t1881+t3121+t3269));
t4111 = t1004+t3912;
t4114 = t1026+t3911;
t4156 = t17.*((t237.*(t42-t43))./9.007199254740992e+15+t21.*(-t1881+t3121+t3269)).*(-1.247162e-2);
t4158 = t18.*(t951+t16.*(-t1881+t3121+t3269)).*(-9.99471e-3);
t4160 = t17.*((t237.*(t42-t43))./9.007199254740992e+15+t21.*(-t1881+t3121+t3269)).*1.247162e-2;
t4172 = t123.*t188.*(t2694-t2701+t3036-t3043).*(-2.442490654175345e-23);
t4180 = t4139.*(-9.99471e-3);
t4183 = t4139.*9.99471e-3;
t4209 = t4139.*(-7.26350557185e-5);
t4211 = t50.*t123.*t189.*(t2694-t2701+t3036-t3043).*(-2.711709361697228e-39);
t4215 = t4139.*7.26350557185e-5;
t4219 = t3480.*t3504;
t4242 = t3317.*t3783;
t4413 = t3514.*t3869;
t4496 = t3514.*t3974;
t4579 = t3312.*t4231;
t4602 = -t4601;
t4614 = t3808.*t3865;
t4615 = t3312.*t4279;
t4616 = t3809.*t3866;
t4640 = t3846.*t3869;
t4647 = t3851.*t3869;
t4650 = t3742.*t4231;
t4660 = t3846.*t3974;
t4663 = t3851.*t3974;
t4667 = t3780.*t4269;
t4681 = t3742.*t4279;
t4682 = -t4679;
t4702 = t3779.*t4279;
t4742 = t3865.*t4116;
t4754 = t3866.*t4115;
t4816 = t3848.*t4269;
t4829 = t3850.*t4269;
t4860 = t2346+t2382+t3168+t3173+t3372+t3374;
t4865 = t2345+t2408+t3167+t3175+t3371+t3378;
t4868 = t3869.*t4232;
t4869 = t3871.*t4231;
t4911 = t3974.*t4232;
t4931 = t3870.*t4279;
t5005 = t4231.*t4281;
t5246 = t3359.*t3617.*(t2674-t2676+t3022-t3027).*(t2694-t2701+t3036-t3043).*2.889644e-2;
t5248 = t3313.*t3628.*(t2674-t2676+t3022-t3027).*(t2694-t2701+t3036-t3043).*2.889644e-2;
t5254 = -t5253;
t5316 = -t5315;
t5320 = -t5319;
t5338 = t236.*t241.*t4301.*t4644.*4.312975891071717e-75;
t5342 = -t5340;
t5344 = t236.*t241.*t4303.*t4644.*2.33806891548878e-94;
t5345 = t236.*t241.*t4325.*t4644.*4.312975891071717e-75;
t5349 = -t5348;
t5380 = -t5378;
t5382 = t236.*t241.*t4301.*t4705.*4.788365138921021e-91;
t5388 = t236.*t241.*t4445.*t4644.*4.788365138921021e-91;
t5399 = -t5398;
t5402 = t236.*t241.*t4303.*t4705.*2.595777943136013e-110;
t5404 = t236.*t241.*t4325.*t4705.*4.788365138921021e-91;
t5407 = -t5406;
t5411 = -t5410;
t5428 = -t5427;
t5444 = -t5443;
t5482 = t236.*t241.*t4445.*t4705.*5.316153227542554e-107;
t5488 = t236.*t241.*t4644.*t4646.*2.33806891548878e-94;
t5492 = -t5491;
t5493 = t236.*t241.*t4301.*t4974.*2.33806891548878e-94;
t5496 = t236.*t241.*t4303.*t4974.*1.267469698796881e-113;
t5497 = t236.*t241.*t4325.*t4974.*2.33806891548878e-94;
t5517 = t236.*t241.*t4646.*t4705.*2.595777943136013e-110;
tau_c = ft_7({t1000,t1002,t1003,t1005,t1006,t1015,t1018,t1020,t1022,t1023,t1035,t1040,t1044,t1045,t1046,t1048,t1049,t1050,t1051,t1058,t1063,t1065,t1067,t1068,t1071,t1083,t1084,t1089,t1093,t1104,t1105,t1108,t1115,t1121,t1158,t1159,t1190,t1193,t1194,t1196,t1205,t1207,t1208,t1210,t1212,t1214,t1217,t1218,t1219,t1220,t1221,t1222,t123,t1230,t1235,t1236,t1237,t1238,t1288,t1289,t1302,t1303,t1319,t1320,t1336,t1348,t1350,t1351,t1360,t1369,t1378,t1396,t14,t140,t1425,t1435,t1456,t1477,t1488,t1492,t1493,t1494,t15,t1504,t1505,t1513,t1514,t1515,t1516,t1522,t1526,t1527,t1529,t1538,t1539,t1543,t1544,t1545,t1546,t1547,t1548,t1549,t1550,t1553,t1554,t1558,t1559,t1564,t1565,t1576,t1577,t1578,t1579,t1581,t1584,t1585,t1586,t1587,t1591,t1595,t1596,t1598,t1599,t16,t1600,t1601,t1602,t1604,t1605,t1606,t1607,t1608,t1609,t1612,t1613,t1614,t1615,t1616,t1626,t1627,t1628,t1629,t1631,t1637,t1640,t1641,t1648,t1649,t1659,t1660,t1661,t1666,t1667,t1683,t1686,t1690,t1692,t17,t1700,t1701,t1703,t1704,t1705,t1712,t1717,t1738,t1741,t1742,t1750,t1752,t1753,t1754,t1758,t1759,t1775,t1776,t18,t1860,t1861,t1864,t1865,t1868,t1870,t1874,t1876,t1879,t188,t1881,t1882,t1884,t1886,t1888,t1889,t189,t1890,t1893,t1896,t19,t1900,t1901,t1903,t1905,t1906,t1911,t1912,t1913,t1918,t1923,t1926,t1927,t1930,t1931,t1933,t1941,t1945,t1946,t1948,t1951,t1952,t1953,t1954,t1956,t1957,t1959,t1962,t1963,t1964,t1966,t1969,t1971,t1973,t1978,t1992,t1993,t1994,t1998,t2,t20,t2004,t201,t202,t2023,t2024,t2028,t2053,t2060,t2073,t2089,t2090,t2098,t2099,t21,t2117,t2120,t2122,t2123,t2125,t2130,t2132,t2135,t2137,t2138,t2139,t2140,t2141,t2142,t2145,t2146,t2147,t2149,t2150,t2151,t2152,t2153,t2154,t2155,t2156,t2157,t2159,t2160,t2162,t2164,t2165,t2166,t2167,t2168,t2169,t2170,t2173,t2174,t2183,t2187,t2193,t2194,t2195,t2199,t22,t2203,t2215,t2219,t2222,t2223,t2239,t2240,t2256,t2257,t2290,t2291,t2292,t2293,t2294,t2295,t2296,t2297,t2298,t2299,t23,t2300,t2301,t2302,t2303,t2304,t2305,t2306,t2307,t2308,t2309,t2310,t2311,t2312,t2313,t2317,t2320,t2322,t2323,t2324,t2325,t2326,t2327,t2328,t2329,t2335,t2336,t2337,t2338,t2339,t2341,t2342,t2343,t2344,t2351,t2352,t2353,t2354,t2355,t2357,t2358,t2359,t236,t2360,t2361,t2362,t2363,t2364,t2365,t2366,t2367,t2368,t2369,t237,t2370,t2371,t2374,t2375,t2377,t2378,t2379,t238,t2380,t2381,t2384,t2385,t2386,t2388,t2389,t2391,t2393,t2394,t2395,t2396,t2397,t2398,t2399,t24,t2400,t2401,t2402,t2403,t2404,t2405,t241,t2410,t2412,t2413,t2414,t2419,t2421,t2422,t2423,t2424,t2433,t2434,t2438,t244,t2445,t2447,t2448,t2449,t2450,t2459,t2460,t2461,t2465,t2468,t2470,t2471,t2472,t2492,t2493,t2494,t2497,t25,t2500,t2501,t2502,t2506,t2507,t2508,t2509,t2510,t2515,t2517,t2520,t2523,t2525,t2527,t2529,t2530,t2531,t2532,t2533,t2534,t2535,t2536,t2537,t2539,t2547,t2553,t2555,t2556,t2572,t2575,t2583,t26,t2602,t2605,t2606,t2612,t2613,t2615,t2618,t2619,t262,t2636,t2638,t264,t2651,t2652,t2663,t2664,t2670,t2671,t2672,t2673,t2674,t2675,t2676,t2677,t2678,t2679,t2680,t2681,t2682,t2683,t2684,t2685,t2686,t2687,t2689,t2690,t2691,t2692,t2693,t2694,t2695,t2696,t2697,t2698,t27,t2700,t2701,t2702,t2703,t2704,t2705,t2707,t2708,t2709,t2711,t2712,t2713,t2715,t2716,t2717,t2719,t2720,t2721,t2732,t2733,t2735,t2736,t2737,t2738,t2739,t2740,t2742,t2743,t2744,t2745,t2746,t2747,t2748,t2749,t2750,t2751,t2752,t2753,t2754,t2755,t2756,t2757,t2759,t2760,t2761,t2762,t2764,t2765,t2768,t2769,t2770,t2773,t2774,t2775,t2776,t2777,t2778,t2779,t2781,t2784,t2785,t2786,t2787,t2788,t2789,t2790,t2791,t2792,t2793,t2795,t2796,t2797,t2798,t2799,t28,t2801,t2802,t2803,t2804,t2805,t2806,t2807,t2808,t2810,t2811,t2812,t2813,t2814,t2815,t2816,t2817,t2818,t2819,t2820,t2821,t2822,t2823,t2824,t2826,t2827,t2828,t2829,t2830,t2831,t2832,t2833,t2834,t2835,t2836,t2837,t2838,t2839,t2840,t2843,t2844,t2845,t2846,t2847,t2848,t2850,t2851,t2852,t2854,t2855,t2856,t2861,t2864,t2866,t2869,t2871,t2873,t2874,t2877,t2878,t2881,t2882,t2885,t2888,t2889,t2897,t2902,t2909,t2927,t2928,t2929,t2932,t2934,t2936,t2937,t2941,t2942,t2945,t2946,t2947,t2948,t2950,t2951,t2953,t2954,t2955,t2956,t2957,t2961,t2962,t2963,t2964,t2965,t2966,t2969,t2970,t2971,t2972,t2973,t2975,t2976,t2977,t2978,t2979,t2981,t2982,t2984,t2985,t2986,t2987,t2990,t2991,t2992,t2993,t2998,t3,t30,t3001,t3002,t3004,t3006,t3008,t3010,t3013,t3014,t3015,t3016,t3017,t3018,t3019,t3022,t3024,t3025,t3027,t3028,t3029,t3030,t3031,t3036,t3038,t3039,t3043,t3044,t3045,t3046,t3047,t3049,t3050,t3051,t3052,t3053,t3054,t3055,t3056,t3057,t3060,t3061,t3064,t3065,t3066,t3067,t3068,t3069,t3072,t3073,t3074,t3075,t3076,t3077,t3078,t3079,t3080,t3081,t3082,t3083,t3085,t3086,t3087,t3088,t3092,t3093,t3094,t3095,t3096,t3097,t31,t3101,t3102,t3103,t3106,t3107,t3108,t3109,t3113,t3115,t3117,t3119,t3120,t3121,t3122,t3123,t3124,t3125,t3126,t3128,t3129,t313,t3130,t3131,t3133,t3134,t3135,t3139,t314,t3140,t3141,t3144,t3145,t3146,t3147,t3148,t3149,t3150,t3151,t3152,t3153,t3154,t3156,t3157,t3158,t3159,t3160,t3161,t3162,t3163,t3164,t3165,t3170,t3171,t3172,t3178,t3179,t3181,t3182,t3183,t3185,t3187,t3189,t3190,t3192,t3198,t32,t3200,t3202,t3203,t3204,t3205,t3206,t3208,t3209,t321,t3218,t322,t3228,t3229,t3259,t326,t3261,t3262,t3263,t3266,t3267,t3268,t3269,t3270,t328,t329,t33,t330,t3306,t3308,t331,t3311,t3313,t3314,t332,t333,t335,t3359,t336,t3361,t3362,t3364,t3365,t3367,t3369,t3370,t3377,t338,t3383,t3384,t339,t34,t341,t3418,t3424,t3427,t343,t3432,t3436,t3438,t3443,t3449,t3450,t3453,t3456,t3457,t3458,t3459,t346,t3460,t3469,t3470,t3471,t3474,t3480,t3498,t35,t350,t351,t352,t3526,t3533,t354,t356,t3560,t358,t359,t36,t360,t3617,t362,t3628,t363,t364,t365,t366,t3670,t3673,t3676,t3689,t369,t370,t371,t372,t3732,t3751,t3753,t3758,t3759,t3762,t3767,t3768,t3770,t3774,t3776,t3779,t378,t3783,t3786,t38,t380,t382,t3827,t3834,t3847,t3849,t3850,t3865,t3866,t3869,t387,t3870,t3871,t3880,t3882,t3883,t3885,t3888,t3890,t3894,t3898,t39,t3904,t3914,t3915,t3917,t3923,t3928,t3930,t3931,t3932,t3934,t3935,t3938,t3940,t3955,t3956,t3960,t3966,t3970,t3971,t3974,t4,t4002,t4003,t4005,t4006,t4012,t4017,t4019,t4092,t4099,t410,t4103,t4104,t4109,t4111,t4129,t4139,t4156,t4158,t4160,t4172,t4182,t4183,t4192,t4194,t42,t4211,t4214,t4215,t4219,t4220,t4230,t4231,t4242,t4279,t4280,t4281,t429,t4295,t43,t4300,t4368,t4371,t4413,t4421,t4444,t4445,t4496,t4500,t4579,t4589,t4599,t46,t4602,t4614,t4615,t4616,t4620,t4640,t4641,t4644,t4645,t4646,t4647,t4650,t4655,t4660,t4663,t4667,t4669,t4679,t4680,t4681,t4682,t47,t4702,t4704,t4705,t4742,t4754,t4789,t4792,t4816,t4823,t4829,t4842,t4860,t4865,t4868,t4869,t4911,t4931,t4974,t4976,t4985,t4986,t5,t50,t5005,t516,t522,t5223,t5224,t5227,t523,t524,t5240,t5243,t5246,t5248,t5252,t5254,t528,t530,t5306,t5308,t5316,t5317,t5320,t5328,t5337,t5338,t5340,t5342,t5344,t5345,t5347,t5348,t5349,t5350,t5377,t5379,t5380,t5381,t5382,t5384,t5388,t5399,t5402,t5403,t5404,t5407,t5411,t542,t5427,t5428,t543,t5443,t5444,t5482,t5485,t5486,t5487,t5488,t549,t5490,t5491,t5492,t5493,t5494,t5496,t5497,t5500,t5517,t5518,t5524,t5549,t5578,t56,t562,t5626,t563,t5630,t5692,t5695,t5722,t5723,t575,t58,t580,t5839,t5840,t587,t59,t594,t5951,t5953,t5954,t6,t60,t610,t612,t6183,t6184,t6185,t628,t635,t636,t638,t640,t641,t642,t643,t644,t645,t646,t648,t649,t654,t655,t656,t657,t659,t660,t663,t664,t665,t666,t667,t668,t669,t67,t670,t672,t673,t674,t675,t676,t677,t678,t679,t68,t681,t682,t683,t684,t685,t686,t687,t689,t691,t692,t693,t694,t7,t70,t702,t707,t708,t71,t710,t715,t716,t717,t718,t721,t722,t724,t725,t73,t736,t738,t740,t741,t749,t756,t76,t762,t768,t777,t792,t793,t801,t802,t808,t813,t819,t821,t850,t855,t874,t878,t89,t90,t91,t92,t941,t944,t945,t948,t949,t950,t951,t97,t974,t983,t989,t996});
end
function tau_c = ft_7(ct)
t1000 = ct{1};
t1002 = ct{2};
t1003 = ct{3};
t1005 = ct{4};
t1006 = ct{5};
t1015 = ct{6};
t1018 = ct{7};
t1020 = ct{8};
t1022 = ct{9};
t1023 = ct{10};
t1035 = ct{11};
t1040 = ct{12};
t1044 = ct{13};
t1045 = ct{14};
t1046 = ct{15};
t1048 = ct{16};
t1049 = ct{17};
t1050 = ct{18};
t1051 = ct{19};
t1058 = ct{20};
t1063 = ct{21};
t1065 = ct{22};
t1067 = ct{23};
t1068 = ct{24};
t1071 = ct{25};
t1083 = ct{26};
t1084 = ct{27};
t1089 = ct{28};
t1093 = ct{29};
t1104 = ct{30};
t1105 = ct{31};
t1108 = ct{32};
t1115 = ct{33};
t1121 = ct{34};
t1158 = ct{35};
t1159 = ct{36};
t1190 = ct{37};
t1193 = ct{38};
t1194 = ct{39};
t1196 = ct{40};
t1205 = ct{41};
t1207 = ct{42};
t1208 = ct{43};
t1210 = ct{44};
t1212 = ct{45};
t1214 = ct{46};
t1217 = ct{47};
t1218 = ct{48};
t1219 = ct{49};
t1220 = ct{50};
t1221 = ct{51};
t1222 = ct{52};
t123 = ct{53};
t1230 = ct{54};
t1235 = ct{55};
t1236 = ct{56};
t1237 = ct{57};
t1238 = ct{58};
t1288 = ct{59};
t1289 = ct{60};
t1302 = ct{61};
t1303 = ct{62};
t1319 = ct{63};
t1320 = ct{64};
t1336 = ct{65};
t1348 = ct{66};
t1350 = ct{67};
t1351 = ct{68};
t1360 = ct{69};
t1369 = ct{70};
t1378 = ct{71};
t1396 = ct{72};
t14 = ct{73};
t140 = ct{74};
t1425 = ct{75};
t1435 = ct{76};
t1456 = ct{77};
t1477 = ct{78};
t1488 = ct{79};
t1492 = ct{80};
t1493 = ct{81};
t1494 = ct{82};
t15 = ct{83};
t1504 = ct{84};
t1505 = ct{85};
t1513 = ct{86};
t1514 = ct{87};
t1515 = ct{88};
t1516 = ct{89};
t1522 = ct{90};
t1526 = ct{91};
t1527 = ct{92};
t1529 = ct{93};
t1538 = ct{94};
t1539 = ct{95};
t1543 = ct{96};
t1544 = ct{97};
t1545 = ct{98};
t1546 = ct{99};
t1547 = ct{100};
t1548 = ct{101};
t1549 = ct{102};
t1550 = ct{103};
t1553 = ct{104};
t1554 = ct{105};
t1558 = ct{106};
t1559 = ct{107};
t1564 = ct{108};
t1565 = ct{109};
t1576 = ct{110};
t1577 = ct{111};
t1578 = ct{112};
t1579 = ct{113};
t1581 = ct{114};
t1584 = ct{115};
t1585 = ct{116};
t1586 = ct{117};
t1587 = ct{118};
t1591 = ct{119};
t1595 = ct{120};
t1596 = ct{121};
t1598 = ct{122};
t1599 = ct{123};
t16 = ct{124};
t1600 = ct{125};
t1601 = ct{126};
t1602 = ct{127};
t1604 = ct{128};
t1605 = ct{129};
t1606 = ct{130};
t1607 = ct{131};
t1608 = ct{132};
t1609 = ct{133};
t1612 = ct{134};
t1613 = ct{135};
t1614 = ct{136};
t1615 = ct{137};
t1616 = ct{138};
t1626 = ct{139};
t1627 = ct{140};
t1628 = ct{141};
t1629 = ct{142};
t1631 = ct{143};
t1637 = ct{144};
t1640 = ct{145};
t1641 = ct{146};
t1648 = ct{147};
t1649 = ct{148};
t1659 = ct{149};
t1660 = ct{150};
t1661 = ct{151};
t1666 = ct{152};
t1667 = ct{153};
t1683 = ct{154};
t1686 = ct{155};
t1690 = ct{156};
t1692 = ct{157};
t17 = ct{158};
t1700 = ct{159};
t1701 = ct{160};
t1703 = ct{161};
t1704 = ct{162};
t1705 = ct{163};
t1712 = ct{164};
t1717 = ct{165};
t1738 = ct{166};
t1741 = ct{167};
t1742 = ct{168};
t1750 = ct{169};
t1752 = ct{170};
t1753 = ct{171};
t1754 = ct{172};
t1758 = ct{173};
t1759 = ct{174};
t1775 = ct{175};
t1776 = ct{176};
t18 = ct{177};
t1860 = ct{178};
t1861 = ct{179};
t1864 = ct{180};
t1865 = ct{181};
t1868 = ct{182};
t1870 = ct{183};
t1874 = ct{184};
t1876 = ct{185};
t1879 = ct{186};
t188 = ct{187};
t1881 = ct{188};
t1882 = ct{189};
t1884 = ct{190};
t1886 = ct{191};
t1888 = ct{192};
t1889 = ct{193};
t189 = ct{194};
t1890 = ct{195};
t1893 = ct{196};
t1896 = ct{197};
t19 = ct{198};
t1900 = ct{199};
t1901 = ct{200};
t1903 = ct{201};
t1905 = ct{202};
t1906 = ct{203};
t1911 = ct{204};
t1912 = ct{205};
t1913 = ct{206};
t1918 = ct{207};
t1923 = ct{208};
t1926 = ct{209};
t1927 = ct{210};
t1930 = ct{211};
t1931 = ct{212};
t1933 = ct{213};
t1941 = ct{214};
t1945 = ct{215};
t1946 = ct{216};
t1948 = ct{217};
t1951 = ct{218};
t1952 = ct{219};
t1953 = ct{220};
t1954 = ct{221};
t1956 = ct{222};
t1957 = ct{223};
t1959 = ct{224};
t1962 = ct{225};
t1963 = ct{226};
t1964 = ct{227};
t1966 = ct{228};
t1969 = ct{229};
t1971 = ct{230};
t1973 = ct{231};
t1978 = ct{232};
t1992 = ct{233};
t1993 = ct{234};
t1994 = ct{235};
t1998 = ct{236};
t2 = ct{237};
t20 = ct{238};
t2004 = ct{239};
t201 = ct{240};
t202 = ct{241};
t2023 = ct{242};
t2024 = ct{243};
t2028 = ct{244};
t2053 = ct{245};
t2060 = ct{246};
t2073 = ct{247};
t2089 = ct{248};
t2090 = ct{249};
t2098 = ct{250};
t2099 = ct{251};
t21 = ct{252};
t2117 = ct{253};
t2120 = ct{254};
t2122 = ct{255};
t2123 = ct{256};
t2125 = ct{257};
t2130 = ct{258};
t2132 = ct{259};
t2135 = ct{260};
t2137 = ct{261};
t2138 = ct{262};
t2139 = ct{263};
t2140 = ct{264};
t2141 = ct{265};
t2142 = ct{266};
t2145 = ct{267};
t2146 = ct{268};
t2147 = ct{269};
t2149 = ct{270};
t2150 = ct{271};
t2151 = ct{272};
t2152 = ct{273};
t2153 = ct{274};
t2154 = ct{275};
t2155 = ct{276};
t2156 = ct{277};
t2157 = ct{278};
t2159 = ct{279};
t2160 = ct{280};
t2162 = ct{281};
t2164 = ct{282};
t2165 = ct{283};
t2166 = ct{284};
t2167 = ct{285};
t2168 = ct{286};
t2169 = ct{287};
t2170 = ct{288};
t2173 = ct{289};
t2174 = ct{290};
t2183 = ct{291};
t2187 = ct{292};
t2193 = ct{293};
t2194 = ct{294};
t2195 = ct{295};
t2199 = ct{296};
t22 = ct{297};
t2203 = ct{298};
t2215 = ct{299};
t2219 = ct{300};
t2222 = ct{301};
t2223 = ct{302};
t2239 = ct{303};
t2240 = ct{304};
t2256 = ct{305};
t2257 = ct{306};
t2290 = ct{307};
t2291 = ct{308};
t2292 = ct{309};
t2293 = ct{310};
t2294 = ct{311};
t2295 = ct{312};
t2296 = ct{313};
t2297 = ct{314};
t2298 = ct{315};
t2299 = ct{316};
t23 = ct{317};
t2300 = ct{318};
t2301 = ct{319};
t2302 = ct{320};
t2303 = ct{321};
t2304 = ct{322};
t2305 = ct{323};
t2306 = ct{324};
t2307 = ct{325};
t2308 = ct{326};
t2309 = ct{327};
t2310 = ct{328};
t2311 = ct{329};
t2312 = ct{330};
t2313 = ct{331};
t2317 = ct{332};
t2320 = ct{333};
t2322 = ct{334};
t2323 = ct{335};
t2324 = ct{336};
t2325 = ct{337};
t2326 = ct{338};
t2327 = ct{339};
t2328 = ct{340};
t2329 = ct{341};
t2335 = ct{342};
t2336 = ct{343};
t2337 = ct{344};
t2338 = ct{345};
t2339 = ct{346};
t2341 = ct{347};
t2342 = ct{348};
t2343 = ct{349};
t2344 = ct{350};
t2351 = ct{351};
t2352 = ct{352};
t2353 = ct{353};
t2354 = ct{354};
t2355 = ct{355};
t2357 = ct{356};
t2358 = ct{357};
t2359 = ct{358};
t236 = ct{359};
t2360 = ct{360};
t2361 = ct{361};
t2362 = ct{362};
t2363 = ct{363};
t2364 = ct{364};
t2365 = ct{365};
t2366 = ct{366};
t2367 = ct{367};
t2368 = ct{368};
t2369 = ct{369};
t237 = ct{370};
t2370 = ct{371};
t2371 = ct{372};
t2374 = ct{373};
t2375 = ct{374};
t2377 = ct{375};
t2378 = ct{376};
t2379 = ct{377};
t238 = ct{378};
t2380 = ct{379};
t2381 = ct{380};
t2384 = ct{381};
t2385 = ct{382};
t2386 = ct{383};
t2388 = ct{384};
t2389 = ct{385};
t2391 = ct{386};
t2393 = ct{387};
t2394 = ct{388};
t2395 = ct{389};
t2396 = ct{390};
t2397 = ct{391};
t2398 = ct{392};
t2399 = ct{393};
t24 = ct{394};
t2400 = ct{395};
t2401 = ct{396};
t2402 = ct{397};
t2403 = ct{398};
t2404 = ct{399};
t2405 = ct{400};
t241 = ct{401};
t2410 = ct{402};
t2412 = ct{403};
t2413 = ct{404};
t2414 = ct{405};
t2419 = ct{406};
t2421 = ct{407};
t2422 = ct{408};
t2423 = ct{409};
t2424 = ct{410};
t2433 = ct{411};
t2434 = ct{412};
t2438 = ct{413};
t244 = ct{414};
t2445 = ct{415};
t2447 = ct{416};
t2448 = ct{417};
t2449 = ct{418};
t2450 = ct{419};
t2459 = ct{420};
t2460 = ct{421};
t2461 = ct{422};
t2465 = ct{423};
t2468 = ct{424};
t2470 = ct{425};
t2471 = ct{426};
t2472 = ct{427};
t2492 = ct{428};
t2493 = ct{429};
t2494 = ct{430};
t2497 = ct{431};
t25 = ct{432};
t2500 = ct{433};
t2501 = ct{434};
t2502 = ct{435};
t2506 = ct{436};
t2507 = ct{437};
t2508 = ct{438};
t2509 = ct{439};
t2510 = ct{440};
t2515 = ct{441};
t2517 = ct{442};
t2520 = ct{443};
t2523 = ct{444};
t2525 = ct{445};
t2527 = ct{446};
t2529 = ct{447};
t2530 = ct{448};
t2531 = ct{449};
t2532 = ct{450};
t2533 = ct{451};
t2534 = ct{452};
t2535 = ct{453};
t2536 = ct{454};
t2537 = ct{455};
t2539 = ct{456};
t2547 = ct{457};
t2553 = ct{458};
t2555 = ct{459};
t2556 = ct{460};
t2572 = ct{461};
t2575 = ct{462};
t2583 = ct{463};
t26 = ct{464};
t2602 = ct{465};
t2605 = ct{466};
t2606 = ct{467};
t2612 = ct{468};
t2613 = ct{469};
t2615 = ct{470};
t2618 = ct{471};
t2619 = ct{472};
t262 = ct{473};
t2636 = ct{474};
t2638 = ct{475};
t264 = ct{476};
t2651 = ct{477};
t2652 = ct{478};
t2663 = ct{479};
t2664 = ct{480};
t2670 = ct{481};
t2671 = ct{482};
t2672 = ct{483};
t2673 = ct{484};
t2674 = ct{485};
t2675 = ct{486};
t2676 = ct{487};
t2677 = ct{488};
t2678 = ct{489};
t2679 = ct{490};
t2680 = ct{491};
t2681 = ct{492};
t2682 = ct{493};
t2683 = ct{494};
t2684 = ct{495};
t2685 = ct{496};
t2686 = ct{497};
t2687 = ct{498};
t2689 = ct{499};
t2690 = ct{500};
t2691 = ct{501};
t2692 = ct{502};
t2693 = ct{503};
t2694 = ct{504};
t2695 = ct{505};
t2696 = ct{506};
t2697 = ct{507};
t2698 = ct{508};
t27 = ct{509};
t2700 = ct{510};
t2701 = ct{511};
t2702 = ct{512};
t2703 = ct{513};
t2704 = ct{514};
t2705 = ct{515};
t2707 = ct{516};
t2708 = ct{517};
t2709 = ct{518};
t2711 = ct{519};
t2712 = ct{520};
t2713 = ct{521};
t2715 = ct{522};
t2716 = ct{523};
t2717 = ct{524};
t2719 = ct{525};
t2720 = ct{526};
t2721 = ct{527};
t2732 = ct{528};
t2733 = ct{529};
t2735 = ct{530};
t2736 = ct{531};
t2737 = ct{532};
t2738 = ct{533};
t2739 = ct{534};
t2740 = ct{535};
t2742 = ct{536};
t2743 = ct{537};
t2744 = ct{538};
t2745 = ct{539};
t2746 = ct{540};
t2747 = ct{541};
t2748 = ct{542};
t2749 = ct{543};
t2750 = ct{544};
t2751 = ct{545};
t2752 = ct{546};
t2753 = ct{547};
t2754 = ct{548};
t2755 = ct{549};
t2756 = ct{550};
t2757 = ct{551};
t2759 = ct{552};
t2760 = ct{553};
t2761 = ct{554};
t2762 = ct{555};
t2764 = ct{556};
t2765 = ct{557};
t2768 = ct{558};
t2769 = ct{559};
t2770 = ct{560};
t2773 = ct{561};
t2774 = ct{562};
t2775 = ct{563};
t2776 = ct{564};
t2777 = ct{565};
t2778 = ct{566};
t2779 = ct{567};
t2781 = ct{568};
t2784 = ct{569};
t2785 = ct{570};
t2786 = ct{571};
t2787 = ct{572};
t2788 = ct{573};
t2789 = ct{574};
t2790 = ct{575};
t2791 = ct{576};
t2792 = ct{577};
t2793 = ct{578};
t2795 = ct{579};
t2796 = ct{580};
t2797 = ct{581};
t2798 = ct{582};
t2799 = ct{583};
t28 = ct{584};
t2801 = ct{585};
t2802 = ct{586};
t2803 = ct{587};
t2804 = ct{588};
t2805 = ct{589};
t2806 = ct{590};
t2807 = ct{591};
t2808 = ct{592};
t2810 = ct{593};
t2811 = ct{594};
t2812 = ct{595};
t2813 = ct{596};
t2814 = ct{597};
t2815 = ct{598};
t2816 = ct{599};
t2817 = ct{600};
t2818 = ct{601};
t2819 = ct{602};
t2820 = ct{603};
t2821 = ct{604};
t2822 = ct{605};
t2823 = ct{606};
t2824 = ct{607};
t2826 = ct{608};
t2827 = ct{609};
t2828 = ct{610};
t2829 = ct{611};
t2830 = ct{612};
t2831 = ct{613};
t2832 = ct{614};
t2833 = ct{615};
t2834 = ct{616};
t2835 = ct{617};
t2836 = ct{618};
t2837 = ct{619};
t2838 = ct{620};
t2839 = ct{621};
t2840 = ct{622};
t2843 = ct{623};
t2844 = ct{624};
t2845 = ct{625};
t2846 = ct{626};
t2847 = ct{627};
t2848 = ct{628};
t2850 = ct{629};
t2851 = ct{630};
t2852 = ct{631};
t2854 = ct{632};
t2855 = ct{633};
t2856 = ct{634};
t2861 = ct{635};
t2864 = ct{636};
t2866 = ct{637};
t2869 = ct{638};
t2871 = ct{639};
t2873 = ct{640};
t2874 = ct{641};
t2877 = ct{642};
t2878 = ct{643};
t2881 = ct{644};
t2882 = ct{645};
t2885 = ct{646};
t2888 = ct{647};
t2889 = ct{648};
t2897 = ct{649};
t2902 = ct{650};
t2909 = ct{651};
t2927 = ct{652};
t2928 = ct{653};
t2929 = ct{654};
t2932 = ct{655};
t2934 = ct{656};
t2936 = ct{657};
t2937 = ct{658};
t2941 = ct{659};
t2942 = ct{660};
t2945 = ct{661};
t2946 = ct{662};
t2947 = ct{663};
t2948 = ct{664};
t2950 = ct{665};
t2951 = ct{666};
t2953 = ct{667};
t2954 = ct{668};
t2955 = ct{669};
t2956 = ct{670};
t2957 = ct{671};
t2961 = ct{672};
t2962 = ct{673};
t2963 = ct{674};
t2964 = ct{675};
t2965 = ct{676};
t2966 = ct{677};
t2969 = ct{678};
t2970 = ct{679};
t2971 = ct{680};
t2972 = ct{681};
t2973 = ct{682};
t2975 = ct{683};
t2976 = ct{684};
t2977 = ct{685};
t2978 = ct{686};
t2979 = ct{687};
t2981 = ct{688};
t2982 = ct{689};
t2984 = ct{690};
t2985 = ct{691};
t2986 = ct{692};
t2987 = ct{693};
t2990 = ct{694};
t2991 = ct{695};
t2992 = ct{696};
t2993 = ct{697};
t2998 = ct{698};
t3 = ct{699};
t30 = ct{700};
t3001 = ct{701};
t3002 = ct{702};
t3004 = ct{703};
t3006 = ct{704};
t3008 = ct{705};
t3010 = ct{706};
t3013 = ct{707};
t3014 = ct{708};
t3015 = ct{709};
t3016 = ct{710};
t3017 = ct{711};
t3018 = ct{712};
t3019 = ct{713};
t3022 = ct{714};
t3024 = ct{715};
t3025 = ct{716};
t3027 = ct{717};
t3028 = ct{718};
t3029 = ct{719};
t3030 = ct{720};
t3031 = ct{721};
t3036 = ct{722};
t3038 = ct{723};
t3039 = ct{724};
t3043 = ct{725};
t3044 = ct{726};
t3045 = ct{727};
t3046 = ct{728};
t3047 = ct{729};
t3049 = ct{730};
t3050 = ct{731};
t3051 = ct{732};
t3052 = ct{733};
t3053 = ct{734};
t3054 = ct{735};
t3055 = ct{736};
t3056 = ct{737};
t3057 = ct{738};
t3060 = ct{739};
t3061 = ct{740};
t3064 = ct{741};
t3065 = ct{742};
t3066 = ct{743};
t3067 = ct{744};
t3068 = ct{745};
t3069 = ct{746};
t3072 = ct{747};
t3073 = ct{748};
t3074 = ct{749};
t3075 = ct{750};
t3076 = ct{751};
t3077 = ct{752};
t3078 = ct{753};
t3079 = ct{754};
t3080 = ct{755};
t3081 = ct{756};
t3082 = ct{757};
t3083 = ct{758};
t3085 = ct{759};
t3086 = ct{760};
t3087 = ct{761};
t3088 = ct{762};
t3092 = ct{763};
t3093 = ct{764};
t3094 = ct{765};
t3095 = ct{766};
t3096 = ct{767};
t3097 = ct{768};
t31 = ct{769};
t3101 = ct{770};
t3102 = ct{771};
t3103 = ct{772};
t3106 = ct{773};
t3107 = ct{774};
t3108 = ct{775};
t3109 = ct{776};
t3113 = ct{777};
t3115 = ct{778};
t3117 = ct{779};
t3119 = ct{780};
t3120 = ct{781};
t3121 = ct{782};
t3122 = ct{783};
t3123 = ct{784};
t3124 = ct{785};
t3125 = ct{786};
t3126 = ct{787};
t3128 = ct{788};
t3129 = ct{789};
t313 = ct{790};
t3130 = ct{791};
t3131 = ct{792};
t3133 = ct{793};
t3134 = ct{794};
t3135 = ct{795};
t3139 = ct{796};
t314 = ct{797};
t3140 = ct{798};
t3141 = ct{799};
t3144 = ct{800};
t3145 = ct{801};
t3146 = ct{802};
t3147 = ct{803};
t3148 = ct{804};
t3149 = ct{805};
t3150 = ct{806};
t3151 = ct{807};
t3152 = ct{808};
t3153 = ct{809};
t3154 = ct{810};
t3156 = ct{811};
t3157 = ct{812};
t3158 = ct{813};
t3159 = ct{814};
t3160 = ct{815};
t3161 = ct{816};
t3162 = ct{817};
t3163 = ct{818};
t3164 = ct{819};
t3165 = ct{820};
t3170 = ct{821};
t3171 = ct{822};
t3172 = ct{823};
t3178 = ct{824};
t3179 = ct{825};
t3181 = ct{826};
t3182 = ct{827};
t3183 = ct{828};
t3185 = ct{829};
t3187 = ct{830};
t3189 = ct{831};
t3190 = ct{832};
t3192 = ct{833};
t3198 = ct{834};
t32 = ct{835};
t3200 = ct{836};
t3202 = ct{837};
t3203 = ct{838};
t3204 = ct{839};
t3205 = ct{840};
t3206 = ct{841};
t3208 = ct{842};
t3209 = ct{843};
t321 = ct{844};
t3218 = ct{845};
t322 = ct{846};
t3228 = ct{847};
t3229 = ct{848};
t3259 = ct{849};
t326 = ct{850};
t3261 = ct{851};
t3262 = ct{852};
t3263 = ct{853};
t3266 = ct{854};
t3267 = ct{855};
t3268 = ct{856};
t3269 = ct{857};
t3270 = ct{858};
t328 = ct{859};
t329 = ct{860};
t33 = ct{861};
t330 = ct{862};
t3306 = ct{863};
t3308 = ct{864};
t331 = ct{865};
t3311 = ct{866};
t3313 = ct{867};
t3314 = ct{868};
t332 = ct{869};
t333 = ct{870};
t335 = ct{871};
t3359 = ct{872};
t336 = ct{873};
t3361 = ct{874};
t3362 = ct{875};
t3364 = ct{876};
t3365 = ct{877};
t3367 = ct{878};
t3369 = ct{879};
t3370 = ct{880};
t3377 = ct{881};
t338 = ct{882};
t3383 = ct{883};
t3384 = ct{884};
t339 = ct{885};
t34 = ct{886};
t341 = ct{887};
t3418 = ct{888};
t3424 = ct{889};
t3427 = ct{890};
t343 = ct{891};
t3432 = ct{892};
t3436 = ct{893};
t3438 = ct{894};
t3443 = ct{895};
t3449 = ct{896};
t3450 = ct{897};
t3453 = ct{898};
t3456 = ct{899};
t3457 = ct{900};
t3458 = ct{901};
t3459 = ct{902};
t346 = ct{903};
t3460 = ct{904};
t3469 = ct{905};
t3470 = ct{906};
t3471 = ct{907};
t3474 = ct{908};
t3480 = ct{909};
t3498 = ct{910};
t35 = ct{911};
t350 = ct{912};
t351 = ct{913};
t352 = ct{914};
t3526 = ct{915};
t3533 = ct{916};
t354 = ct{917};
t356 = ct{918};
t3560 = ct{919};
t358 = ct{920};
t359 = ct{921};
t36 = ct{922};
t360 = ct{923};
t3617 = ct{924};
t362 = ct{925};
t3628 = ct{926};
t363 = ct{927};
t364 = ct{928};
t365 = ct{929};
t366 = ct{930};
t3670 = ct{931};
t3673 = ct{932};
t3676 = ct{933};
t3689 = ct{934};
t369 = ct{935};
t370 = ct{936};
t371 = ct{937};
t372 = ct{938};
t3732 = ct{939};
t3751 = ct{940};
t3753 = ct{941};
t3758 = ct{942};
t3759 = ct{943};
t3762 = ct{944};
t3767 = ct{945};
t3768 = ct{946};
t3770 = ct{947};
t3774 = ct{948};
t3776 = ct{949};
t3779 = ct{950};
t378 = ct{951};
t3783 = ct{952};
t3786 = ct{953};
t38 = ct{954};
t380 = ct{955};
t382 = ct{956};
t3827 = ct{957};
t3834 = ct{958};
t3847 = ct{959};
t3849 = ct{960};
t3850 = ct{961};
t3865 = ct{962};
t3866 = ct{963};
t3869 = ct{964};
t387 = ct{965};
t3870 = ct{966};
t3871 = ct{967};
t3880 = ct{968};
t3882 = ct{969};
t3883 = ct{970};
t3885 = ct{971};
t3888 = ct{972};
t3890 = ct{973};
t3894 = ct{974};
t3898 = ct{975};
t39 = ct{976};
t3904 = ct{977};
t3914 = ct{978};
t3915 = ct{979};
t3917 = ct{980};
t3923 = ct{981};
t3928 = ct{982};
t3930 = ct{983};
t3931 = ct{984};
t3932 = ct{985};
t3934 = ct{986};
t3935 = ct{987};
t3938 = ct{988};
t3940 = ct{989};
t3955 = ct{990};
t3956 = ct{991};
t3960 = ct{992};
t3966 = ct{993};
t3970 = ct{994};
t3971 = ct{995};
t3974 = ct{996};
t4 = ct{997};
t4002 = ct{998};
t4003 = ct{999};
t4005 = ct{1000};
t4006 = ct{1001};
t4012 = ct{1002};
t4017 = ct{1003};
t4019 = ct{1004};
t4092 = ct{1005};
t4099 = ct{1006};
t410 = ct{1007};
t4103 = ct{1008};
t4104 = ct{1009};
t4109 = ct{1010};
t4111 = ct{1011};
t4129 = ct{1012};
t4139 = ct{1013};
t4156 = ct{1014};
t4158 = ct{1015};
t4160 = ct{1016};
t4172 = ct{1017};
t4182 = ct{1018};
t4183 = ct{1019};
t4192 = ct{1020};
t4194 = ct{1021};
t42 = ct{1022};
t4211 = ct{1023};
t4214 = ct{1024};
t4215 = ct{1025};
t4219 = ct{1026};
t4220 = ct{1027};
t4230 = ct{1028};
t4231 = ct{1029};
t4242 = ct{1030};
t4279 = ct{1031};
t4280 = ct{1032};
t4281 = ct{1033};
t429 = ct{1034};
t4295 = ct{1035};
t43 = ct{1036};
t4300 = ct{1037};
t4368 = ct{1038};
t4371 = ct{1039};
t4413 = ct{1040};
t4421 = ct{1041};
t4444 = ct{1042};
t4445 = ct{1043};
t4496 = ct{1044};
t4500 = ct{1045};
t4579 = ct{1046};
t4589 = ct{1047};
t4599 = ct{1048};
t46 = ct{1049};
t4602 = ct{1050};
t4614 = ct{1051};
t4615 = ct{1052};
t4616 = ct{1053};
t4620 = ct{1054};
t4640 = ct{1055};
t4641 = ct{1056};
t4644 = ct{1057};
t4645 = ct{1058};
t4646 = ct{1059};
t4647 = ct{1060};
t4650 = ct{1061};
t4655 = ct{1062};
t4660 = ct{1063};
t4663 = ct{1064};
t4667 = ct{1065};
t4669 = ct{1066};
t4679 = ct{1067};
t4680 = ct{1068};
t4681 = ct{1069};
t4682 = ct{1070};
t47 = ct{1071};
t4702 = ct{1072};
t4704 = ct{1073};
t4705 = ct{1074};
t4742 = ct{1075};
t4754 = ct{1076};
t4789 = ct{1077};
t4792 = ct{1078};
t4816 = ct{1079};
t4823 = ct{1080};
t4829 = ct{1081};
t4842 = ct{1082};
t4860 = ct{1083};
t4865 = ct{1084};
t4868 = ct{1085};
t4869 = ct{1086};
t4911 = ct{1087};
t4931 = ct{1088};
t4974 = ct{1089};
t4976 = ct{1090};
t4985 = ct{1091};
t4986 = ct{1092};
t5 = ct{1093};
t50 = ct{1094};
t5005 = ct{1095};
t516 = ct{1096};
t522 = ct{1097};
t5223 = ct{1098};
t5224 = ct{1099};
t5227 = ct{1100};
t523 = ct{1101};
t524 = ct{1102};
t5240 = ct{1103};
t5243 = ct{1104};
t5246 = ct{1105};
t5248 = ct{1106};
t5252 = ct{1107};
t5254 = ct{1108};
t528 = ct{1109};
t530 = ct{1110};
t5306 = ct{1111};
t5308 = ct{1112};
t5316 = ct{1113};
t5317 = ct{1114};
t5320 = ct{1115};
t5328 = ct{1116};
t5337 = ct{1117};
t5338 = ct{1118};
t5340 = ct{1119};
t5342 = ct{1120};
t5344 = ct{1121};
t5345 = ct{1122};
t5347 = ct{1123};
t5348 = ct{1124};
t5349 = ct{1125};
t5350 = ct{1126};
t5377 = ct{1127};
t5379 = ct{1128};
t5380 = ct{1129};
t5381 = ct{1130};
t5382 = ct{1131};
t5384 = ct{1132};
t5388 = ct{1133};
t5399 = ct{1134};
t5402 = ct{1135};
t5403 = ct{1136};
t5404 = ct{1137};
t5407 = ct{1138};
t5411 = ct{1139};
t542 = ct{1140};
t5427 = ct{1141};
t5428 = ct{1142};
t543 = ct{1143};
t5443 = ct{1144};
t5444 = ct{1145};
t5482 = ct{1146};
t5485 = ct{1147};
t5486 = ct{1148};
t5487 = ct{1149};
t5488 = ct{1150};
t549 = ct{1151};
t5490 = ct{1152};
t5491 = ct{1153};
t5492 = ct{1154};
t5493 = ct{1155};
t5494 = ct{1156};
t5496 = ct{1157};
t5497 = ct{1158};
t5500 = ct{1159};
t5517 = ct{1160};
t5518 = ct{1161};
t5524 = ct{1162};
t5549 = ct{1163};
t5578 = ct{1164};
t56 = ct{1165};
t562 = ct{1166};
t5626 = ct{1167};
t563 = ct{1168};
t5630 = ct{1169};
t5692 = ct{1170};
t5695 = ct{1171};
t5722 = ct{1172};
t5723 = ct{1173};
t575 = ct{1174};
t58 = ct{1175};
t580 = ct{1176};
t5839 = ct{1177};
t5840 = ct{1178};
t587 = ct{1179};
t59 = ct{1180};
t594 = ct{1181};
t5951 = ct{1182};
t5953 = ct{1183};
t5954 = ct{1184};
t6 = ct{1185};
t60 = ct{1186};
t610 = ct{1187};
t612 = ct{1188};
t6183 = ct{1189};
t6184 = ct{1190};
t6185 = ct{1191};
t628 = ct{1192};
t635 = ct{1193};
t636 = ct{1194};
t638 = ct{1195};
t640 = ct{1196};
t641 = ct{1197};
t642 = ct{1198};
t643 = ct{1199};
t644 = ct{1200};
t645 = ct{1201};
t646 = ct{1202};
t648 = ct{1203};
t649 = ct{1204};
t654 = ct{1205};
t655 = ct{1206};
t656 = ct{1207};
t657 = ct{1208};
t659 = ct{1209};
t660 = ct{1210};
t663 = ct{1211};
t664 = ct{1212};
t665 = ct{1213};
t666 = ct{1214};
t667 = ct{1215};
t668 = ct{1216};
t669 = ct{1217};
t67 = ct{1218};
t670 = ct{1219};
t672 = ct{1220};
t673 = ct{1221};
t674 = ct{1222};
t675 = ct{1223};
t676 = ct{1224};
t677 = ct{1225};
t678 = ct{1226};
t679 = ct{1227};
t68 = ct{1228};
t681 = ct{1229};
t682 = ct{1230};
t683 = ct{1231};
t684 = ct{1232};
t685 = ct{1233};
t686 = ct{1234};
t687 = ct{1235};
t689 = ct{1236};
t691 = ct{1237};
t692 = ct{1238};
t693 = ct{1239};
t694 = ct{1240};
t7 = ct{1241};
t70 = ct{1242};
t702 = ct{1243};
t707 = ct{1244};
t708 = ct{1245};
t71 = ct{1246};
t710 = ct{1247};
t715 = ct{1248};
t716 = ct{1249};
t717 = ct{1250};
t718 = ct{1251};
t721 = ct{1252};
t722 = ct{1253};
t724 = ct{1254};
t725 = ct{1255};
t73 = ct{1256};
t736 = ct{1257};
t738 = ct{1258};
t740 = ct{1259};
t741 = ct{1260};
t749 = ct{1261};
t756 = ct{1262};
t76 = ct{1263};
t762 = ct{1264};
t768 = ct{1265};
t777 = ct{1266};
t792 = ct{1267};
t793 = ct{1268};
t801 = ct{1269};
t802 = ct{1270};
t808 = ct{1271};
t813 = ct{1272};
t819 = ct{1273};
t821 = ct{1274};
t850 = ct{1275};
t855 = ct{1276};
t874 = ct{1277};
t878 = ct{1278};
t89 = ct{1279};
t90 = ct{1280};
t91 = ct{1281};
t92 = ct{1282};
t941 = ct{1283};
t944 = ct{1284};
t945 = ct{1285};
t948 = ct{1286};
t949 = ct{1287};
t950 = ct{1288};
t951 = ct{1289};
t97 = ct{1290};
t974 = ct{1291};
t983 = ct{1292};
t989 = ct{1293};
t996 = ct{1294};
t5531 = t236.*t241.*t4445.*t4974.*2.595777943136013e-110;
t5552 = -t5549;
t5580 = -t5578;
t5620 = t236.*t241.*t4646.*t4974.*1.267469698796881e-113;
t5627 = -t5626;
t5631 = -t5630;
t5634 = t2125+t2142+t2750+t2762+t2796+t2811+t2812+t3203+t3457+t4006+t4017;
t5694 = -t5692;
et9 = -t2125-t2142+t2745-t2750+t2774+t2785+t2786-t3457+t4002+t32.*(t1941-t3308+t39.*t1022.*(t855-t878).*2.196325630278387e-1).*1.869599668e-7;
et10 = t38.*t1022.*(t855-t878).*1.46680315462752e-4;
t5931 = t3617.*(et9+et10).*(t2674-t2676+t3022-t3027);
t6543 = t5486.*t5951;
et11 = t707+t708-t721-t722-t749+t762+t768-t777-t792-t793-t801-t802-t808+t813-t819+t821-t1629+t1637-t1640-t1641-t1659-t1661+t1666+t1667+t1683+t1692+t1705-t1712+t1758+t1759+t1775+t1776+t1973+t1993+t1994+t2023+t2053+t2060-t2089-t2090+t2098+t2099-t14.*t15.*t21.*t50.*t189.*3.670836568391568e-22;
et12 = t16.*t19.*t20.*t50.*t189.*(-3.279367663374749e-19)-t14.*t15.*t17.*t21.*t50.*t189.*7.075931802640439e-19;
et13 = t14.*t17.*t20.*t21.*t50.*t189.*(-1.190170786299927e-18)-t15.*t17.*t19.*t21.*t50.*t189.*1.190170786299927e-18;
et14 = t19.*t20.*t21.*t22.*t50.*t189.*(-3.226512155691387e-19);
t6544 = -t5485.*(et11+et12+et13+et14);
t6658 = t5224.*t6183;
et15 = t1288+t1289+t1302+t1303-t1319-t1320+t1336-t1348+t1350+t1351-t1360+t1369-t1378+t1396-t1425+t1435-t2174+t2183-t2187+t2193-t2194-t2195+t2199-t2203-t2215+t2219-t2222-t2223+t2239+t2240-t2256-t2257+t2555+t2556+t2572+t2583-t2605-t2606+t2612+t2613-t2618-t2619+t2651+t2652;
et16 = t24.*t25.*t26.*t50.*t202.*(-3.566935413776081e-21);
et17 = t30.*t31.*t32.*t50.*t202.*(-3.992732227073824e-24);
et18 = t24.*t25.*t32.*t33.*t50.*t202.*(-3.509445006623964e-21);
et19 = t27.*t30.*t31.*t32.*t50.*t202.*(-7.696420262413979e-21);
t6661 = -t5223.*(et15+et16+et17+et18+et19);
et20 = t1288+t1289+t1302+t1303-t1319-t1320+t1336-t1348+t1350+t1351-t1360+t1369-t1378+t1396-t1425+t1435-t2174+t2183-t2187+t2193-t2194-t2195+t2199-t2203-t2215+t2219-t2222-t2223+t2239+t2240-t2256-t2257+t2555+t2556+t2572+t2583-t2605-t2606+t2612+t2613-t2618-t2619+t2651+t2652;
et21 = t24.*t25.*t26.*t50.*t202.*(-3.566935413776081e-21);
et22 = t30.*t31.*t32.*t50.*t202.*(-3.992732227073824e-24);
et23 = t24.*t25.*t32.*t33.*t50.*t202.*(-3.509445006623964e-21);
et24 = t27.*t30.*t31.*t32.*t50.*t202.*(-7.696420262413979e-21);
t6663 = t5223.*(et20+et21+et22+et23+et24);
t6811 = t5839.*t5951;
et25 = t707+t708-t721-t722-t749+t762+t768-t777-t792-t793-t801-t802-t808+t813-t819+t821-t1629+t1637-t1640-t1641-t1659-t1661+t1666+t1667+t1683+t1692+t1705-t1712+t1758+t1759+t1775+t1776+t1973+t1993+t1994+t2023+t2053+t2060-t2089-t2090+t2098+t2099-t14.*t15.*t21.*t50.*t189.*3.670836568391568e-22;
et26 = t16.*t19.*t20.*t50.*t189.*(-3.279367663374749e-19)-t14.*t15.*t17.*t21.*t50.*t189.*7.075931802640439e-19;
et27 = t14.*t17.*t20.*t21.*t50.*t189.*(-1.190170786299927e-18)-t15.*t17.*t19.*t21.*t50.*t189.*1.190170786299927e-18;
et28 = t19.*t20.*t21.*t22.*t50.*t189.*(-3.226512155691387e-19);
t6812 = -t5840.*(et25+et26+et27+et28);
et29 = t707+t708-t721-t722-t749+t762+t768-t777-t792-t793-t801-t802-t808+t813-t819+t821-t1629+t1637-t1640-t1641-t1659-t1661+t1666+t1667+t1683+t1692+t1705-t1712+t1758+t1759+t1775+t1776+t1973+t1993+t1994+t2023+t2053+t2060-t2089-t2090+t2098+t2099-t14.*t15.*t21.*t50.*t189.*3.670836568391568e-22;
et30 = t16.*t19.*t20.*t50.*t189.*(-3.279367663374749e-19)-t14.*t15.*t17.*t21.*t50.*t189.*7.075931802640439e-19;
et31 = t14.*t17.*t20.*t21.*t50.*t189.*(-1.190170786299927e-18)-t15.*t17.*t19.*t21.*t50.*t189.*1.190170786299927e-18;
et32 = t19.*t20.*t21.*t22.*t50.*t189.*(-3.226512155691387e-19);
t6813 = t5840.*(et29+et30+et31+et32);
t6892 = t5722.*t6183;
et33 = t1288+t1289+t1302+t1303-t1319-t1320+t1336-t1348+t1350+t1351-t1360+t1369-t1378+t1396-t1425+t1435-t2174+t2183-t2187+t2193-t2194-t2195+t2199-t2203-t2215+t2219-t2222-t2223+t2239+t2240-t2256-t2257+t2555+t2556+t2572+t2583-t2605-t2606+t2612+t2613-t2618-t2619+t2651+t2652;
et34 = t24.*t25.*t26.*t50.*t202.*(-3.566935413776081e-21);
et35 = t30.*t31.*t32.*t50.*t202.*(-3.992732227073824e-24);
et36 = t24.*t25.*t32.*t33.*t50.*t202.*(-3.509445006623964e-21);
et37 = t27.*t30.*t31.*t32.*t50.*t202.*(-7.696420262413979e-21);
t6893 = -t5723.*(et33+et34+et35+et36+et37);
t2519 = -t2506;
t2598 = -t2553;
t2669 = -t2663;
t2763 = -t2746;
t2766 = -t2756;
t2772 = -t2760;
t2794 = -t2770;
t2809 = -t2784;
t2841 = -t2824;
t2842 = -t2826;
t2853 = -t2833;
t2862 = -t2847;
t2863 = -t2848;
t2876 = -t2852;
t2880 = -t2854;
t2904 = -t2861;
t2910 = -t2869;
t2912 = -t2873;
t2913 = -t2874;
t2916 = -t2882;
t2921 = -t2888;
t2938 = -t2928;
t2994 = t516+t2445;
t2995 = t18.*t2992;
t2996 = t23.*t2992;
t3003 = t522+t2533;
t3007 = t28.*t2998;
t3009 = t34.*t2998;
t3062 = t1550+t2615;
t3089 = t23.*t3047.*9.99471e-3;
t3090 = t18.*t3047.*1.838876e-2;
t3098 = t18.*t3047.*1.02e-6;
t3099 = t23.*t3047.*9.3e-7;
t3104 = t18.*t3047.*9.0e-8;
t3105 = t23.*t3047.*9.0e-8;
t3110 = t34.*t3057.*9.99471e-3;
t3111 = t28.*t3057.*1.838876e-2;
t3112 = t3061.*(-9.99471e-3);
t3114 = t3061.*(-1.838876e-2);
t3116 = t3061.*9.99471e-3;
t3118 = t3061.*1.838876e-2;
t3127 = t2351+t2424;
t3132 = t1956+t2827;
t3138 = t1969+t2828;
t3142 = t2497+t2537;
t3155 = t201.*t3047.*8.595599785252598e-9;
t3180 = t201.*t3047.*8.76751178095765e-7;
t3184 = t50.*t202.*t2992.*5.439528691468777e-23;
t3186 = t201.*t3047.*2.062943948460623e-7;
t3191 = t201.*t3047.*3.438239914101039e-8;
t3193 = t50.*t202.*t2992.*3.817213116820194e-24;
t3210 = t2132+t3002;
t3211 = t2135+t3001;
t3212 = t50.*t202.*t3047.*9.543032792050485e-25;
t3214 = t16.*t3208;
t3215 = t17.*t3209;
t3216 = t21.*t3208;
t3217 = t22.*t3209;
t3230 = t2170+t3013;
t3231 = t2173+t3014;
t3232 = t26.*t3228;
t3233 = t27.*t3229;
t3234 = t32.*t3228;
t3235 = t33.*t3229;
t3252 = t50.*t202.*t3047.*9.733893447891495e-23;
t3253 = t23.*t50.*t202.*t3047.*8.875020496606951e-23;
t3254 = t50.*t202.*t3047.*5.439528691468777e-23;
t3256 = t50.*t202.*t3047.*2.290327870092116e-23;
t3260 = t50.*t202.*t3047.*3.817213116820194e-24;
t3264 = t18.*t50.*t202.*t3047.*8.588729512845436e-24;
t3265 = t23.*t50.*t202.*t3047.*8.588729512845436e-24;
t3315 = -t3314;
t3316 = t2363.*t2992.*5.7e-7;
t3326 = t2363.*t2992.*4.0e-8;
t3360 = t2335+t3053;
t3366 = t2381+t3052;
t3373 = (t2363.*t3047)./1.0e+8;
t3376 = (t2388.*t3047)./1.0e+8;
t3382 = (t2419.*t3047)./1.0e+8;
t3385 = t2465+t3060;
t3386 = t2468+t3061;
t3387 = -t2363.*(t1545-t2615);
t3415 = t50.*t202.*t3123.*9.733893447891495e-23;
t3421 = t50.*t202.*t3123.*8.588729512845436e-24;
t3422 = t2363.*t3047.*5.7e-7;
t3423 = t2363.*t3047.*1.02e-6;
t3426 = t2388.*t3047.*1.02e-6;
t3428 = t2363.*t3047.*2.4e-7;
t3435 = t2388.*t3047.*2.4e-7;
t3437 = t2363.*t3047.*4.0e-8;
t3441 = t2419.*t3047.*1.02e-6;
t3442 = t2388.*t3047.*4.0e-8;
t3444 = t2419.*t3047.*2.4e-7;
t3447 = t27.*t2363.*t3047.*(-1.02e-6);
t3451 = t2419.*t3047.*4.0e-8;
t3452 = t17.*t2297.*t3057.*1.02e-6;
t3462 = t188.*t3229.*6.899985389504867e-8;
t3463 = t188.*t3228.*3.878758105047274e-8;
t3468 = t580+t1546+t1903+t2602;
t3473 = t2363.*t3123.*1.02e-6;
t3475 = t2363.*t3123.*9.0e-8;
t3517 = t50.*t189.*t3228.*4.306286555174926e-24;
t3520 = t50.*t189.*t3229.*7.660522649005482e-24;
t3566 = -t3560;
t3677 = t3047.*t3057.*1.02e-6;
t3678 = t3057.*(t1456-t2355).*(-1.02e-6);
t3679 = t3047.*(t1477-t2502).*(-1.02e-6);
t3682 = t18.*t3047.*t3057.*(-1.02e-6);
t3683 = t23.*t3047.*t3057.*(-9.3e-7);
t3686 = t18.*t3047.*t3057.*(-9.0e-8);
t3687 = t23.*t3047.*t3057.*(-9.0e-8);
t3734 = -t3057.*(t1953-t2828);
t3738 = t2981.*t3229;
t3739 = t3057.*(t1953-t2828);
t3764 = t3057.*t3123.*1.02e-6;
t3766 = t27.*t3751;
t3771 = t3057.*t3123.*9.0e-8;
t3772 = t27.*t3758;
t3782 = t1884+t1906+t2756+t2768;
t3784 = t1926+t1946+t2847+t2866;
t3788 = t1952+t2073+t2821+t2874;
t3790 = -t3786;
t3793 = t1978+t2028+t2846+t2871;
t3802 = t3120.*t3229;
t3819 = t3057.*(t2337+t18.*(t1456-t2355)).*(-9.3e-7);
t3820 = t3057.*(t2337+t18.*(t1456-t2355)).*(-1.02e-6);
t3826 = t3057.*(t2337+t18.*(t1456-t2355)).*1.02e-6;
t3828 = t3057.*(t2337+t18.*(t1456-t2355)).*(-9.0e-8);
t3832 = t3165.*t3229;
t3833 = t3057.*(t2337+t18.*(t1456-t2355)).*9.0e-8;
t3852 = t3209.*t3229.*3.24e-6;
t3853 = t3209.*t3229.*3.11e-6;
t3862 = -t3057.*(t335-t1539-t2831+t2851);
t3864 = t3057.*(t335-t1539-t2831+t2851);
t3877 = t2672+t2679+t3025+t3028;
t3878 = t2676+t2677+t3024+t3027;
t3879 = t1881+t3124+t3267;
t3881 = t1901+t3125+t3268;
t3884 = t16.*t3880;
t3886 = t21.*t3880;
t3887 = t17.*t3882;
t3889 = t22.*t3882;
t3901 = t2691+t2703+t3039+t3046;
t3902 = t2701+t2702+t3038+t3043;
t3907 = t26.*t3898;
t3908 = t32.*t3898;
t3909 = t33.*t3904;
t3913 = t27.*t3904;
t4081 = t950+t3885;
t4085 = t974+t3883;
t4105 = t4103.*(-3.0./5.0e+2);
t4107 = t4103.*(3.0./5.0e+2);
t4108 = t2738+t2739+t3094+t3095;
t4117 = t33.*t4111;
t4122 = t2810+t2835+t3106+t3108;
t4123 = t2804+t2856+t3102+t3107;
t4124 = t2830+t2835+t3101+t3108;
t4125 = t2806+t2838+t3103+t3109;
t4127 = t27.*t4111;
t4159 = t4104.*(-1.838876e-2);
t4163 = t4103.*(-5.68686e-3);
t4165 = t4104.*1.838876e-2;
t4167 = t4103.*5.68686e-3;
t4169 = t4103.*(-3.131399999999998e-4);
t4171 = t4103.*3.131399999999998e-4;
t4191 = t50.*t189.*t3898.*4.306286555174926e-24;
t4193 = t50.*t189.*t3904.*7.660522649005482e-24;
t4221 = -t4219;
t4244 = -t4242;
t4283 = t2973.*t4111;
t4299 = t3165.*t3904;
t4317 = -t28.*t3057.*(t2813-t2835+t18.*(t1456-t2355).*1.02e-6+t23.*(t1456-t2355).*9.0e-8);
t4318 = -t34.*t3057.*(-t2804+t2838+t3109+t23.*(t1456-t2355).*9.3e-7);
t4321 = t28.*t3057.*(t2813-t2835+t18.*(t1456-t2355).*1.02e-6+t23.*(t1456-t2355).*9.0e-8);
t4322 = t34.*t3057.*(-t2804+t2838+t3109+t23.*(t1456-t2355).*9.3e-7);
t4327 = t3229.*t3882.*3.24e-6;
t4328 = t3229.*t3882.*3.11e-6;
t4331 = t3209.*(t2694-t2701+t3036-t3043).*(-1.1e-7);
t4332 = t3209.*(t2694-t2701+t3036-t3043).*(-3.24e-6);
t4334 = t3209.*(t2694-t2701+t3036-t3043).*1.1e-7;
t4335 = t3209.*(t2694-t2701+t3036-t3043).*(-3.11e-6);
t4337 = t3209.*(t2694-t2701+t3036-t3043).*3.24e-6;
t4339 = t3209.*(t2694-t2701+t3036-t3043).*3.11e-6;
t4340 = t3208.*(t2694-t2701+t3036-t3043).*(-5.0e-8);
t4341 = t3209.*(t2694-t2701+t3036-t3043).*(-5.0e-8);
t4342 = t3208.*(t2694-t2701+t3036-t3043).*(-1.6e-7);
t4343 = t3209.*(t1959-t3306+t38.*t1022.*(t855-t878).*2.196325630278387e-1).*(-3.11e-6);
t4345 = t3209.*(t1959-t3306+t38.*t1022.*(t855-t878).*2.196325630278387e-1).*(-3.24e-6);
t4348 = t3209.*(t2694-t2701+t3036-t3043).*5.0e-8;
t4351 = t3209.*(t1959-t3306+t38.*t1022.*(t855-t878).*2.196325630278387e-1).*3.11e-6;
t4352 = t3209.*(t1959-t3306+t38.*t1022.*(t855-t878).*2.196325630278387e-1).*3.24e-6;
t4360 = -t3141.*(t2813-t2835+t18.*(t1456-t2355).*1.02e-6+t23.*(t1456-t2355).*9.0e-8);
t4363 = t3141.*(t2813-t2835+t18.*(t1456-t2355).*1.02e-6+t23.*(t1456-t2355).*9.0e-8);
t4384 = t3185+t3418+t3469;
t4414 = t1504+t1888+t2506+t2737+t2752+t3092+t3093;
t4617 = -t4616;
t4642 = -t4640;
t4652 = -t4650;
t4661 = -t4660;
t4664 = -t4663;
t4683 = -t4681;
t4686 = t3882.*(t2694-t2701+t3036-t3043).*(-1.1e-7);
t4688 = t3882.*(t2694-t2701+t3036-t3043).*(-3.24e-6);
t4691 = t3882.*(t2694-t2701+t3036-t3043).*1.1e-7;
t4692 = t3880.*(t2694-t2701+t3036-t3043).*(-5.0e-8);
t4693 = t3882.*(t2694-t2701+t3036-t3043).*(-3.11e-6);
t4696 = t3880.*(t2694-t2701+t3036-t3043).*(-1.6e-7);
t4697 = t3882.*(t2694-t2701+t3036-t3043).*3.24e-6;
t4698 = t3882.*(t2694-t2701+t3036-t3043).*3.11e-6;
t4699 = t3882.*(t2694-t2701+t3036-t3043).*(-5.0e-8);
t4701 = t3882.*(t2694-t2701+t3036-t3043).*5.0e-8;
t4703 = -t4702;
t4758 = t549+t1890+t1911+t1962+t2737+t2752+t2755+t2816+t3092+t3093;
t4772 = -t4754;
t4778 = t3890+t4092;
t4779 = t3888+t4103;
t4815 = t2306+t2317+t3146+t3151+t3362+t3364;
t4822 = t2305+t2336+t3145+t3148+t3361+t3365;
t4826 = -t4816;
t4870 = -t4868;
t4871 = -t4869;
t4898 = t3126+t3181+t3182+t3202+t3471;
t4964 = t50.*t189.*t4860.*(t42-t43).*(-2.711709361697228e-39);
t4965 = t50.*t123.*t189.*t4865.*2.711709361697228e-39;
t5007 = -t5005;
t5038 = t3209.*t4865.*1.1e-7;
t5042 = t3209.*t4865.*3.24e-6;
t5044 = t3209.*t4865.*3.11e-6;
t5047 = t3208.*t4865.*5.0e-8;
t5048 = t3209.*t4865.*5.0e-8;
t5049 = t3208.*t4865.*1.6e-7;
t5339 = -t5338;
t5346 = -t5345;
t5383 = -t5382;
t5389 = -t5388;
t5405 = -t5404;
t5498 = -t5497;
t5510 = t1549+t1565+t2327+t2328+t2357+t2375+t2377+t3150+t3370+t3932+t3935;
t5932 = -t5931;
t6217 = t3732.*t5951.*(t2694-t2701+t3036-t3043).*(-1.08769e-2);
t6219 = t3732.*t5951.*(t2694-t2701+t3036-t3043).*1.08769e-2;
t2997 = -t2996;
t3020 = t2996.*9.99471e-3;
t3021 = t2995.*1.838876e-2;
t3032 = t2995.*1.02e-6;
t3033 = t2996.*9.3e-7;
t3034 = t2995.*9.0e-8;
t3035 = t2996.*9.0e-8;
t3040 = t3009.*9.99471e-3;
t3041 = t3007.*1.838876e-2;
t3063 = t1058+t2863;
t3166 = t50.*t202.*t2994.*9.543032792050485e-25;
t3188 = -t3184;
t3194 = -t3191;
t3196 = t50.*t202.*t2994.*9.733893447891495e-23;
t3197 = t50.*t202.*t2994.*2.290327870092116e-23;
t3199 = t50.*t202.*t2994.*3.817213116820194e-24;
t3219 = t16.*t3211;
t3220 = t17.*t3210;
t3221 = t21.*t3211;
t3222 = t22.*t3210;
t3223 = t3215.*(3.0./5.0e+2);
t3224 = t3217.*(3.0./5.0e+2);
t3236 = t2412+t2995;
t3237 = t26.*t3231;
t3238 = t27.*t3230;
t3239 = t32.*t3231;
t3240 = t33.*t3230;
t3241 = -t3235;
t3243 = t3233.*(3.0./5.0e+2);
t3244 = t3235.*(3.0./5.0e+2);
t3249 = (t2363.*t2994)./1.0e+8;
t3250 = t2531+t3007;
t3251 = t2536+t3009;
t3258 = t18.*t3252;
t3271 = t3215.*1.247162e-2;
t3272 = t3217.*1.247162e-2;
t3273 = t3214.*5.84482e-3;
t3274 = t3216.*5.84482e-3;
t3278 = t3215.*5.68686e-3;
t3279 = t3217.*5.68686e-3;
t3280 = t3214.*6.48e-5;
t3283 = t3216.*6.48e-5;
t3296 = t3215.*3.131399999999998e-4;
t3297 = t3217.*3.131399999999998e-4;
t3299 = t3214.*6.47e-6;
t3300 = t3216.*6.47e-6;
t3318 = t3233.*1.247162e-2;
t3319 = t3235.*1.247162e-2;
t3320 = t3232.*5.84482e-3;
t3321 = t3234.*5.84482e-3;
t3327 = t3232.*6.48e-5;
t3330 = t3234.*6.48e-5;
t3333 = t2363.*t2994.*1.02e-6;
t3334 = t3235.*3.131399999999998e-4;
t3335 = t2363.*t2994.*2.4e-7;
t3341 = t3233.*3.131399999999998e-4;
t3344 = t2363.*t2994.*4.0e-8;
t3346 = t3232.*6.47e-6;
t3347 = t3234.*6.47e-6;
t3348 = t3233.*4.36041e-5;
t3349 = t3235.*4.36041e-5;
t3379 = -t3376;
t3388 = t3233.*1.35652563578e-4;
t3389 = t3235.*1.35652563578e-4;
t3390 = t3232.*1.688944904408e-4;
t3391 = t3234.*1.688944904408e-4;
t3392 = t3233.*6.1855407534e-5;
t3393 = t3235.*6.1855407534e-5;
t3402 = t3232.*7.0482312e-7;
t3403 = t3234.*7.0482312e-7;
t3406 = t3232.*1.869599668e-7;
t3407 = t3234.*1.869599668e-7;
t3417 = t50.*t202.*t3127.*8.875020496606951e-23;
t3420 = t648+t1048+t1522+t2669;
t3425 = t50.*t202.*t3127.*8.588729512845436e-24;
t3429 = t2363.*t3098;
t3430 = t2363.*t3099;
t3434 = -t3426;
t3439 = t27.*t3423;
t3440 = -t3435;
t3445 = t2363.*t3104;
t3446 = t2363.*t3105;
t3455 = -t3452;
t3461 = t27.*t2363.*t3132;
t3464 = t188.*t3230.*6.899985389504867e-8;
t3466 = t188.*t3231.*3.878758105047274e-8;
t3476 = t2363.*t3127.*9.3e-7;
t3478 = t2363.*t3127.*9.0e-8;
t3481 = t1860+t3216;
t3482 = t1864+t3214;
t3489 = -t18.*(t1861-t3214);
t3490 = -t23.*(t1861-t3214);
t3505 = t18.*t22.*(t1861-t3214);
t3511 = t22.*(t1861-t3214).*(-3.0./5.0e+2);
t3519 = t50.*t189.*t3231.*4.306286555174926e-24;
t3521 = t50.*t189.*t3230.*7.660522649005482e-24;
t3522 = t201.*t3360.*7.993907800284916e-7;
t3524 = t1893+t3234;
t3525 = t1912+t3232;
t3527 = t201.*t3360.*7.736039806727338e-8;
t3540 = -t28.*(t1896-t3232);
t3541 = -t34.*(t1896-t3232);
t3547 = t28.*(t1896-t3232);
t3558 = t2994.*t3057.*1.02e-6;
t3559 = t3003.*t3047.*1.02e-6;
t3561 = t33.*(t1896-t3232).*(-3.0./5.0e+2);
t3576 = t18.*(t1861-t3214).*(-9.99471e-3);
t3577 = t23.*(t1861-t3214).*(-9.99471e-3);
t3578 = t18.*(t1861-t3214).*(-1.838876e-2);
t3579 = t23.*(t1861-t3214).*(-1.838876e-2);
t3581 = t17.*(t1861-t3214).*(-1.247162e-2);
t3583 = t22.*(t1861-t3214).*(-5.68686e-3);
t3584 = t18.*(t1861-t3214).*9.99471e-3;
t3588 = t23.*(t1861-t3214).*1.838876e-2;
t3590 = t17.*(t1861-t3214).*1.247162e-2;
t3607 = t22.*(t1861-t3214).*(-3.131399999999998e-4);
t3623 = t34.*(t1896-t3232).*(-9.99471e-3);
t3625 = t34.*(t1896-t3232).*(-1.838876e-2);
t3627 = t27.*(t1896-t3232).*(-1.247162e-2);
t3634 = t34.*(t1896-t3232).*1.838876e-2;
t3645 = t33.*(t1896-t3232).*(-3.131399999999998e-4);
t3655 = t33.*(t1896-t3232).*(-4.36041e-5);
t3662 = t3003.*t3132;
t3666 = t50.*t202.*t3360.*8.875020496606951e-23;
t3669 = t50.*t202.*t3360.*9.733893447891495e-23;
t3672 = t50.*t202.*t3360.*8.588729512845436e-24;
t3680 = t3057.*t3098;
t3681 = t3057.*t3099;
t3684 = t3057.*t3104;
t3685 = t3057.*t3105;
t3688 = t1065+t1084+t2845+t2916;
t3697 = t27.*(t1896-t3232).*(-1.35652563578e-4);
t3700 = t34.*(t1896-t3232).*(-1.33637554986e-4);
t3703 = t34.*(t1896-t3232).*(-7.26350557185e-5);
t3704 = t33.*(t1896-t3232).*(-6.1855407534e-5);
t3707 = t27.*(t1896-t3232).*1.35652563578e-4;
t3733 = t3057.*t3132;
t3735 = -t3132.*(t1477-t2502);
t3736 = t3099+t3104;
t3737 = t3098+t3105;
t3740 = t3132.*(t1477-t2502);
t3741 = t2981.*t3230;
t3745 = t2363.*t3360.*9.3e-7;
t3746 = t2363.*t3360.*1.02e-6;
t3747 = t2388.*t3360.*9.3e-7;
t3748 = t2363.*t3360.*9.0e-8;
t3752 = t2388.*t3360.*9.0e-8;
t3756 = t2419.*t3360.*9.3e-7;
t3765 = t2419.*t3360.*9.0e-8;
t3773 = t3057.*t3127.*9.3e-7;
t3777 = t3057.*t3127.*9.0e-8;
t3785 = t2363.*t3468;
t3787 = t2388.*t3468;
t3789 = t1951+t2028+t2841+t2871;
t3792 = t2419.*t3468;
t3795 = t3003.*t3360.*9.3e-7;
t3798 = t3003.*t3360.*9.0e-8;
t3799 = t3003.*(t2337+t18.*(t1456-t2355)).*(-1.02e-6);
t3804 = t3003.*(t2337+t18.*(t1456-t2355)).*(-9.0e-8);
t3805 = t3120.*t3230;
t3807 = -t3802;
t3810 = t3057.*t3360.*9.3e-7;
t3811 = t3057.*t3360.*1.02e-6;
t3815 = t3360.*(t1477-t2502).*(-9.3e-7);
t3817 = t3057.*t3360.*9.0e-8;
t3822 = t3360.*(t1477-t2502).*(-9.0e-8);
t3823 = -t2973.*(t1896-t3232);
t3836 = t3165.*t3230;
t3840 = -t2976.*(t1896-t3232);
t3842 = t2976.*(t1896-t3232);
t3843 = t612+t989+t1071+t1083+t2885+t2912;
t3844 = t2840+t2842+t2855+t2877;
t3845 = t2829+t2839+t2878+t2880;
t3854 = t3210.*t3230.*3.24e-6;
t3855 = t3210.*t3230.*3.11e-6;
t3856 = (t1545-t2615).*(t1896-t3232);
t3863 = t336+t1538+t1966+t2024+t2843+t2913;
t3867 = -t3119.*(t1896-t3232);
t3874 = -t27.*t3132.*(t1896-t3232);
t3876 = t27.*t3132.*(t1896-t3232);
t3891 = t1000+t1002+t1006+t1040+t1493+t2772+t2776;
t3892 = t1492+t2501+t3089+t3090;
t3893 = t3887.*(3.0./5.0e+2);
t3896 = -t3154.*(t1896-t3232);
t3900 = t3154.*(t1896-t3232);
t3910 = t1003+t1035+t1044+t1063+t1515+t2876+t2881;
t3916 = t3913.*(3.0./5.0e+2);
t3918 = t1514+t2547+t3110+t3111;
t3920 = t3884.*5.84482e-3;
t3921 = t3889.*1.247162e-2;
t3925 = t3884.*6.48e-5;
t3929 = t3887.*5.68686e-3;
t3936 = t3886.*6.47e-6;
t3937 = t3887.*3.131399999999998e-4;
t3941 = t2470+t2751+t2761+t2763+t2764;
t3944 = t3909.*1.247162e-2;
t3947 = t3907.*5.84482e-3;
t3952 = t3907.*6.48e-5;
t3953 = -t3206.*(t1896-t3232);
t3962 = t3913.*3.131399999999998e-4;
t3964 = t3908.*6.47e-6;
t3965 = t3913.*4.36041e-5;
t3976 = t3229.*(t1861-t3214).*(-1.0e-8);
t3984 = t2535+t2836+t2853+t2889+t2897;
t3988 = -t3788.*(t1477-t2502);
t3993 = t3057.*t3793;
t3994 = t3788.*(t1477-t2502);
t3997 = t3907.*1.688944904408e-4;
t3998 = t3913.*6.1855407534e-5;
t4000 = t3909.*1.35652563578e-4;
t4004 = t3907.*7.0482312e-7;
tau_c = ft_8({t1000,t1003,t1005,t1015,t1018,t1020,t1022,t1023,t1045,t1046,t1049,t1050,t1051,t1067,t1068,t1089,t1093,t1104,t1105,t1108,t1115,t1121,t1158,t1159,t1190,t1193,t1194,t1196,t1205,t1207,t1208,t1210,t1212,t1214,t1217,t1218,t1219,t1220,t1221,t1222,t123,t1230,t1235,t1236,t1237,t1238,t1288,t1289,t1302,t1303,t1319,t1320,t1336,t1348,t1350,t1351,t1360,t1369,t1378,t1396,t14,t140,t1425,t1435,t1456,t1477,t1488,t1494,t15,t1505,t1513,t1516,t1526,t1527,t1529,t1539,t1543,t1544,t1545,t1547,t1548,t1549,t1553,t1554,t1558,t1559,t1564,t1565,t1576,t1577,t1578,t1579,t1581,t1584,t1585,t1586,t1587,t1591,t1595,t1596,t1598,t1599,t16,t1600,t1601,t1602,t1604,t1605,t1606,t1607,t1608,t1609,t1612,t1613,t1614,t1615,t1616,t1626,t1627,t1628,t1629,t1631,t1637,t1640,t1641,t1648,t1649,t1659,t1660,t1661,t1666,t1667,t1683,t1686,t1690,t1692,t17,t1700,t1701,t1703,t1704,t1705,t1712,t1717,t1738,t1741,t1742,t1750,t1752,t1753,t1754,t1758,t1759,t1775,t1776,t18,t1861,t1865,t1868,t1870,t1874,t1876,t1879,t188,t1881,t1882,t1886,t1889,t189,t1890,t1896,t19,t1900,t1901,t1905,t1911,t1913,t1918,t1923,t1927,t1930,t1931,t1933,t1941,t1945,t1948,t1953,t1954,t1957,t1959,t1963,t1964,t1971,t1973,t1992,t1993,t1994,t1998,t2,t20,t2004,t201,t202,t2023,t2053,t2060,t2089,t2090,t2098,t2099,t21,t2117,t2120,t2122,t2123,t2125,t2130,t2137,t2138,t2139,t2140,t2141,t2142,t2145,t2146,t2147,t2149,t2150,t2151,t2152,t2153,t2154,t2155,t2156,t2157,t2159,t2160,t2162,t2164,t2165,t2166,t2167,t2168,t2169,t2174,t2183,t2187,t2193,t2194,t2195,t2199,t22,t2203,t2215,t2219,t2222,t2223,t2239,t2240,t2256,t2257,t2290,t2291,t2292,t2293,t2294,t2295,t2296,t2297,t2298,t2299,t23,t2300,t2301,t2302,t2303,t2304,t2306,t2307,t2308,t2309,t2310,t2311,t2312,t2313,t2317,t2320,t2322,t2323,t2324,t2325,t2326,t2327,t2328,t2329,t2337,t2338,t2339,t2341,t2342,t2343,t2344,t2352,t2353,t2354,t2355,t2357,t2358,t2359,t236,t2360,t2361,t2362,t2363,t2364,t2365,t2366,t2367,t2368,t2369,t237,t2370,t2371,t2374,t2375,t2378,t2379,t238,t2380,t2384,t2385,t2386,t2388,t2389,t2391,t2393,t2394,t2395,t2396,t2397,t2398,t2399,t24,t2400,t2401,t2402,t2403,t2404,t2405,t241,t2410,t2413,t2414,t2419,t2421,t2422,t2423,t2433,t2434,t2438,t244,t2447,t2448,t2449,t2450,t2459,t2460,t2461,t2471,t2472,t2492,t2493,t2494,t25,t2500,t2502,t2507,t2508,t2509,t2510,t2515,t2517,t2519,t2520,t2523,t2525,t2527,t2529,t2530,t2532,t2534,t2539,t2553,t2555,t2556,t2572,t2575,t2583,t2598,t26,t2605,t2606,t2612,t2613,t2615,t2618,t2619,t262,t2636,t2638,t264,t2651,t2652,t2664,t2670,t2671,t2673,t2674,t2675,t2676,t2678,t2680,t2681,t2682,t2683,t2684,t2685,t2686,t2687,t2689,t2690,t2692,t2693,t2694,t2695,t2696,t2697,t2698,t27,t2700,t2701,t2704,t2705,t2707,t2708,t2709,t2711,t2712,t2713,t2715,t2716,t2717,t2719,t2720,t2721,t2732,t2733,t2735,t2736,t2740,t2742,t2743,t2744,t2745,t2747,t2748,t2749,t2750,t2751,t2753,t2754,t2755,t2757,t2759,t2760,t2761,t2763,t2764,t2765,t2766,t2769,t2773,t2774,t2775,t2777,t2778,t2779,t2781,t2785,t2786,t2787,t2788,t2789,t2790,t2791,t2792,t2793,t2794,t2795,t2797,t2798,t2799,t28,t2801,t2802,t2803,t2804,t2805,t2807,t2808,t2809,t2813,t2814,t2815,t2817,t2818,t2819,t2820,t2822,t2823,t2828,t2831,t2832,t2834,t2835,t2836,t2837,t2838,t2844,t2850,t2851,t2852,t2853,t2862,t2864,t2889,t2897,t2902,t2904,t2909,t2910,t2921,t2927,t2929,t2932,t2934,t2936,t2937,t2938,t2941,t2942,t2945,t2946,t2947,t2948,t2950,t2951,t2953,t2954,t2955,t2956,t2957,t2961,t2962,t2963,t2964,t2965,t2966,t2969,t2970,t2971,t2972,t2973,t2975,t2976,t2977,t2978,t2979,t2982,t2984,t2985,t2986,t2987,t2990,t2991,t2993,t2994,t2997,t2998,t3,t30,t3003,t3004,t3006,t3008,t3009,t3010,t3015,t3016,t3017,t3018,t3019,t3020,t3021,t3022,t3027,t3029,t3030,t3031,t3032,t3033,t3034,t3035,t3036,t3040,t3041,t3043,t3044,t3045,t3047,t3049,t3050,t3051,t3054,t3055,t3056,t3057,t3063,t3064,t3065,t3066,t3067,t3068,t3069,t3072,t3073,t3074,t3075,t3076,t3077,t3078,t3079,t3080,t3081,t3082,t3083,t3085,t3086,t3087,t3088,t3089,t3090,t3096,t3097,t31,t3109,t3110,t3111,t3113,t3114,t3115,t3116,t3117,t3118,t3119,t3121,t3122,t3128,t3129,t313,t3130,t3131,t3132,t3133,t3134,t3135,t3139,t314,t3140,t3141,t3142,t3144,t3147,t3149,t3150,t3152,t3153,t3154,t3155,t3156,t3157,t3158,t3159,t3160,t3161,t3162,t3163,t3164,t3165,t3166,t3170,t3171,t3172,t3178,t3179,t3180,t3183,t3184,t3186,t3187,t3188,t3189,t3190,t3191,t3192,t3193,t3194,t3196,t3197,t3198,t3199,t32,t3200,t3204,t3205,t3206,t3209,t321,t3210,t3211,t3212,t3214,t3215,t3217,t3218,t3219,t322,t3220,t3221,t3222,t3223,t3224,t3228,t3229,t3230,t3231,t3232,t3233,t3235,t3236,t3237,t3238,t3239,t3240,t3241,t3243,t3244,t3249,t3250,t3252,t3253,t3254,t3256,t3258,t3259,t326,t3260,t3261,t3262,t3263,t3264,t3265,t3266,t3269,t3270,t3271,t3272,t3273,t3274,t3278,t3279,t328,t3280,t3283,t329,t3296,t3297,t3299,t33,t330,t3300,t3306,t3308,t331,t3311,t3313,t3315,t3316,t3318,t3319,t332,t3320,t3321,t3326,t3327,t333,t3330,t3333,t3334,t3335,t3341,t3344,t3346,t3347,t3348,t3349,t335,t3359,t3360,t3367,t3369,t3370,t3373,t3376,t3377,t3379,t338,t3382,t3383,t3384,t3385,t3386,t3387,t3388,t3389,t339,t3390,t3391,t3392,t3393,t34,t3402,t3403,t3406,t3407,t341,t3415,t3417,t3420,t3421,t3422,t3423,t3424,t3425,t3427,t3428,t3429,t343,t3430,t3432,t3434,t3435,t3436,t3437,t3438,t3440,t3441,t3442,t3443,t3444,t3445,t3446,t3447,t3449,t3450,t3451,t3452,t3453,t3455,t3456,t3457,t3458,t3459,t346,t3460,t3461,t3462,t3463,t3464,t3466,t3468,t3470,t3473,t3474,t3475,t3476,t3478,t3480,t3481,t3489,t3490,t3498,t35,t350,t3505,t351,t3511,t3517,t3519,t352,t3520,t3521,t3522,t3524,t3526,t3527,t3533,t354,t3540,t3541,t3547,t3558,t3559,t356,t3560,t3561,t3566,t3576,t3577,t3578,t3579,t358,t3581,t3583,t3584,t3588,t359,t3590,t36,t360,t3607,t3617,t362,t3623,t3625,t3627,t3628,t363,t3634,t364,t3645,t365,t3655,t366,t3662,t3666,t3669,t3670,t3672,t3673,t3676,t3677,t3678,t3679,t3680,t3681,t3682,t3683,t3684,t3685,t3686,t3687,t3688,t3689,t369,t370,t3700,t3703,t3704,t3707,t371,t372,t3732,t3733,t3734,t3735,t3736,t3737,t3738,t3739,t3740,t3741,t3745,t3746,t3747,t3748,t3751,t3752,t3753,t3756,t3758,t3759,t3762,t3764,t3765,t3766,t3767,t3768,t3770,t3771,t3772,t3773,t3774,t3776,t3777,t3779,t378,t3782,t3783,t3784,t3785,t3786,t3787,t3788,t3789,t3790,t3792,t3793,t3795,t3798,t3799,t38,t380,t3802,t3804,t3805,t3807,t3810,t3811,t3815,t3817,t3819,t382,t3822,t3823,t3826,t3827,t3828,t3832,t3833,t3834,t3836,t3842,t3843,t3844,t3845,t3847,t3849,t3850,t3852,t3853,t3854,t3855,t3856,t3862,t3863,t3864,t3865,t3866,t3867,t3869,t387,t3870,t3871,t3876,t3877,t3880,t3882,t3884,t3886,t3887,t3889,t3891,t3892,t3893,t3894,t3898,t39,t3900,t3901,t3904,t3907,t3908,t3909,t3910,t3913,t3914,t3915,t3916,t3917,t3918,t3920,t3921,t3923,t3925,t3928,t3929,t3930,t3931,t3932,t3934,t3935,t3936,t3937,t3938,t3940,t3941,t3944,t3947,t3952,t3953,t3955,t3956,t3960,t3962,t3964,t3965,t3966,t3970,t3971,t3974,t3976,t3984,t3993,t3994,t3997,t3998,t4,t4000,t4002,t4003,t4004,t4005,t4012,t4019,t4099,t410,t4104,t4107,t4108,t4109,t4111,t4117,t4122,t4125,t4127,t4129,t4139,t4156,t4158,t4160,t4163,t4165,t4167,t4171,t4172,t4182,t4183,t4191,t4192,t4193,t4194,t42,t4211,t4214,t4215,t4219,t4220,t4221,t4230,t4231,t4242,t4244,t4279,t4280,t4281,t4283,t429,t4295,t4299,t43,t4300,t4317,t4318,t4321,t4322,t4327,t4328,t4334,t4337,t4339,t4340,t4342,t4348,t4351,t4352,t4360,t4363,t4368,t4371,t4384,t4413,t4421,t4444,t4496,t4500,t4579,t4589,t4599,t46,t4602,t4614,t4615,t4617,t4620,t4640,t4641,t4642,t4644,t4645,t4647,t4650,t4652,t4655,t4661,t4663,t4664,t4667,t4669,t4679,t4680,t4682,t4683,t4686,t4688,t4691,t4692,t4693,t4696,t4697,t4698,t4699,t47,t4701,t4702,t4703,t4704,t4705,t4742,t4758,t4772,t4779,t4789,t4792,t4816,t4822,t4823,t4826,t4829,t4842,t4860,t4865,t4868,t4869,t4870,t4871,t4898,t4911,t4931,t4964,t4965,t4974,t4976,t4985,t4986,t5,t50,t5005,t5007,t5038,t5042,t5044,t5047,t5048,t5049,t5223,t5224,t5227,t523,t524,t5240,t5243,t5246,t5248,t5252,t5254,t528,t530,t5306,t5308,t5316,t5317,t5320,t5328,t5337,t5338,t5339,t5340,t5342,t5344,t5345,t5346,t5347,t5348,t5349,t5350,t5377,t5379,t5380,t5381,t5383,t5384,t5388,t5389,t5399,t5402,t5403,t5405,t5407,t5411,t542,t5427,t5428,t543,t5443,t5444,t5482,t5485,t5486,t5487,t5488,t549,t5490,t5491,t5492,t5493,t5494,t5496,t5498,t5500,t5510,t5517,t5518,t5524,t5531,t5552,t5578,t5580,t56,t562,t5620,t5626,t5627,t563,t5631,t5694,t5695,t5722,t5723,t575,t58,t5839,t5840,t587,t59,t5932,t594,t5951,t5953,t5954,t6,t60,t610,t6183,t6184,t6185,t6219,t628,t635,t636,t638,t640,t641,t642,t643,t644,t645,t646,t649,t654,t6543,t6544,t655,t656,t657,t659,t660,t663,t664,t665,t6658,t666,t6663,t667,t668,t669,t67,t670,t672,t673,t674,t675,t676,t677,t678,t679,t68,t681,t6811,t6812,t6813,t682,t683,t684,t685,t686,t687,t689,t6892,t6893,t691,t692,t693,t694,t7,t70,t702,t707,t708,t71,t710,t715,t716,t717,t718,t721,t722,t724,t725,t73,t736,t738,t740,t741,t749,t756,t76,t762,t768,t777,t792,t793,t801,t802,t808,t813,t819,t821,t850,t855,t874,t878,t89,t90,t91,t92,t941,t944,t945,t948,t949,t951,t97,t983,t996});
end
function tau_c = ft_8(ct)
t1000 = ct{1};
t1003 = ct{2};
t1005 = ct{3};
t1015 = ct{4};
t1018 = ct{5};
t1020 = ct{6};
t1022 = ct{7};
t1023 = ct{8};
t1045 = ct{9};
t1046 = ct{10};
t1049 = ct{11};
t1050 = ct{12};
t1051 = ct{13};
t1067 = ct{14};
t1068 = ct{15};
t1089 = ct{16};
t1093 = ct{17};
t1104 = ct{18};
t1105 = ct{19};
t1108 = ct{20};
t1115 = ct{21};
t1121 = ct{22};
t1158 = ct{23};
t1159 = ct{24};
t1190 = ct{25};
t1193 = ct{26};
t1194 = ct{27};
t1196 = ct{28};
t1205 = ct{29};
t1207 = ct{30};
t1208 = ct{31};
t1210 = ct{32};
t1212 = ct{33};
t1214 = ct{34};
t1217 = ct{35};
t1218 = ct{36};
t1219 = ct{37};
t1220 = ct{38};
t1221 = ct{39};
t1222 = ct{40};
t123 = ct{41};
t1230 = ct{42};
t1235 = ct{43};
t1236 = ct{44};
t1237 = ct{45};
t1238 = ct{46};
t1288 = ct{47};
t1289 = ct{48};
t1302 = ct{49};
t1303 = ct{50};
t1319 = ct{51};
t1320 = ct{52};
t1336 = ct{53};
t1348 = ct{54};
t1350 = ct{55};
t1351 = ct{56};
t1360 = ct{57};
t1369 = ct{58};
t1378 = ct{59};
t1396 = ct{60};
t14 = ct{61};
t140 = ct{62};
t1425 = ct{63};
t1435 = ct{64};
t1456 = ct{65};
t1477 = ct{66};
t1488 = ct{67};
t1494 = ct{68};
t15 = ct{69};
t1505 = ct{70};
t1513 = ct{71};
t1516 = ct{72};
t1526 = ct{73};
t1527 = ct{74};
t1529 = ct{75};
t1539 = ct{76};
t1543 = ct{77};
t1544 = ct{78};
t1545 = ct{79};
t1547 = ct{80};
t1548 = ct{81};
t1549 = ct{82};
t1553 = ct{83};
t1554 = ct{84};
t1558 = ct{85};
t1559 = ct{86};
t1564 = ct{87};
t1565 = ct{88};
t1576 = ct{89};
t1577 = ct{90};
t1578 = ct{91};
t1579 = ct{92};
t1581 = ct{93};
t1584 = ct{94};
t1585 = ct{95};
t1586 = ct{96};
t1587 = ct{97};
t1591 = ct{98};
t1595 = ct{99};
t1596 = ct{100};
t1598 = ct{101};
t1599 = ct{102};
t16 = ct{103};
t1600 = ct{104};
t1601 = ct{105};
t1602 = ct{106};
t1604 = ct{107};
t1605 = ct{108};
t1606 = ct{109};
t1607 = ct{110};
t1608 = ct{111};
t1609 = ct{112};
t1612 = ct{113};
t1613 = ct{114};
t1614 = ct{115};
t1615 = ct{116};
t1616 = ct{117};
t1626 = ct{118};
t1627 = ct{119};
t1628 = ct{120};
t1629 = ct{121};
t1631 = ct{122};
t1637 = ct{123};
t1640 = ct{124};
t1641 = ct{125};
t1648 = ct{126};
t1649 = ct{127};
t1659 = ct{128};
t1660 = ct{129};
t1661 = ct{130};
t1666 = ct{131};
t1667 = ct{132};
t1683 = ct{133};
t1686 = ct{134};
t1690 = ct{135};
t1692 = ct{136};
t17 = ct{137};
t1700 = ct{138};
t1701 = ct{139};
t1703 = ct{140};
t1704 = ct{141};
t1705 = ct{142};
t1712 = ct{143};
t1717 = ct{144};
t1738 = ct{145};
t1741 = ct{146};
t1742 = ct{147};
t1750 = ct{148};
t1752 = ct{149};
t1753 = ct{150};
t1754 = ct{151};
t1758 = ct{152};
t1759 = ct{153};
t1775 = ct{154};
t1776 = ct{155};
t18 = ct{156};
t1861 = ct{157};
t1865 = ct{158};
t1868 = ct{159};
t1870 = ct{160};
t1874 = ct{161};
t1876 = ct{162};
t1879 = ct{163};
t188 = ct{164};
t1881 = ct{165};
t1882 = ct{166};
t1886 = ct{167};
t1889 = ct{168};
t189 = ct{169};
t1890 = ct{170};
t1896 = ct{171};
t19 = ct{172};
t1900 = ct{173};
t1901 = ct{174};
t1905 = ct{175};
t1911 = ct{176};
t1913 = ct{177};
t1918 = ct{178};
t1923 = ct{179};
t1927 = ct{180};
t1930 = ct{181};
t1931 = ct{182};
t1933 = ct{183};
t1941 = ct{184};
t1945 = ct{185};
t1948 = ct{186};
t1953 = ct{187};
t1954 = ct{188};
t1957 = ct{189};
t1959 = ct{190};
t1963 = ct{191};
t1964 = ct{192};
t1971 = ct{193};
t1973 = ct{194};
t1992 = ct{195};
t1993 = ct{196};
t1994 = ct{197};
t1998 = ct{198};
t2 = ct{199};
t20 = ct{200};
t2004 = ct{201};
t201 = ct{202};
t202 = ct{203};
t2023 = ct{204};
t2053 = ct{205};
t2060 = ct{206};
t2089 = ct{207};
t2090 = ct{208};
t2098 = ct{209};
t2099 = ct{210};
t21 = ct{211};
t2117 = ct{212};
t2120 = ct{213};
t2122 = ct{214};
t2123 = ct{215};
t2125 = ct{216};
t2130 = ct{217};
t2137 = ct{218};
t2138 = ct{219};
t2139 = ct{220};
t2140 = ct{221};
t2141 = ct{222};
t2142 = ct{223};
t2145 = ct{224};
t2146 = ct{225};
t2147 = ct{226};
t2149 = ct{227};
t2150 = ct{228};
t2151 = ct{229};
t2152 = ct{230};
t2153 = ct{231};
t2154 = ct{232};
t2155 = ct{233};
t2156 = ct{234};
t2157 = ct{235};
t2159 = ct{236};
t2160 = ct{237};
t2162 = ct{238};
t2164 = ct{239};
t2165 = ct{240};
t2166 = ct{241};
t2167 = ct{242};
t2168 = ct{243};
t2169 = ct{244};
t2174 = ct{245};
t2183 = ct{246};
t2187 = ct{247};
t2193 = ct{248};
t2194 = ct{249};
t2195 = ct{250};
t2199 = ct{251};
t22 = ct{252};
t2203 = ct{253};
t2215 = ct{254};
t2219 = ct{255};
t2222 = ct{256};
t2223 = ct{257};
t2239 = ct{258};
t2240 = ct{259};
t2256 = ct{260};
t2257 = ct{261};
t2290 = ct{262};
t2291 = ct{263};
t2292 = ct{264};
t2293 = ct{265};
t2294 = ct{266};
t2295 = ct{267};
t2296 = ct{268};
t2297 = ct{269};
t2298 = ct{270};
t2299 = ct{271};
t23 = ct{272};
t2300 = ct{273};
t2301 = ct{274};
t2302 = ct{275};
t2303 = ct{276};
t2304 = ct{277};
t2306 = ct{278};
t2307 = ct{279};
t2308 = ct{280};
t2309 = ct{281};
t2310 = ct{282};
t2311 = ct{283};
t2312 = ct{284};
t2313 = ct{285};
t2317 = ct{286};
t2320 = ct{287};
t2322 = ct{288};
t2323 = ct{289};
t2324 = ct{290};
t2325 = ct{291};
t2326 = ct{292};
t2327 = ct{293};
t2328 = ct{294};
t2329 = ct{295};
t2337 = ct{296};
t2338 = ct{297};
t2339 = ct{298};
t2341 = ct{299};
t2342 = ct{300};
t2343 = ct{301};
t2344 = ct{302};
t2352 = ct{303};
t2353 = ct{304};
t2354 = ct{305};
t2355 = ct{306};
t2357 = ct{307};
t2358 = ct{308};
t2359 = ct{309};
t236 = ct{310};
t2360 = ct{311};
t2361 = ct{312};
t2362 = ct{313};
t2363 = ct{314};
t2364 = ct{315};
t2365 = ct{316};
t2366 = ct{317};
t2367 = ct{318};
t2368 = ct{319};
t2369 = ct{320};
t237 = ct{321};
t2370 = ct{322};
t2371 = ct{323};
t2374 = ct{324};
t2375 = ct{325};
t2378 = ct{326};
t2379 = ct{327};
t238 = ct{328};
t2380 = ct{329};
t2384 = ct{330};
t2385 = ct{331};
t2386 = ct{332};
t2388 = ct{333};
t2389 = ct{334};
t2391 = ct{335};
t2393 = ct{336};
t2394 = ct{337};
t2395 = ct{338};
t2396 = ct{339};
t2397 = ct{340};
t2398 = ct{341};
t2399 = ct{342};
t24 = ct{343};
t2400 = ct{344};
t2401 = ct{345};
t2402 = ct{346};
t2403 = ct{347};
t2404 = ct{348};
t2405 = ct{349};
t241 = ct{350};
t2410 = ct{351};
t2413 = ct{352};
t2414 = ct{353};
t2419 = ct{354};
t2421 = ct{355};
t2422 = ct{356};
t2423 = ct{357};
t2433 = ct{358};
t2434 = ct{359};
t2438 = ct{360};
t244 = ct{361};
t2447 = ct{362};
t2448 = ct{363};
t2449 = ct{364};
t2450 = ct{365};
t2459 = ct{366};
t2460 = ct{367};
t2461 = ct{368};
t2471 = ct{369};
t2472 = ct{370};
t2492 = ct{371};
t2493 = ct{372};
t2494 = ct{373};
t25 = ct{374};
t2500 = ct{375};
t2502 = ct{376};
t2507 = ct{377};
t2508 = ct{378};
t2509 = ct{379};
t2510 = ct{380};
t2515 = ct{381};
t2517 = ct{382};
t2519 = ct{383};
t2520 = ct{384};
t2523 = ct{385};
t2525 = ct{386};
t2527 = ct{387};
t2529 = ct{388};
t2530 = ct{389};
t2532 = ct{390};
t2534 = ct{391};
t2539 = ct{392};
t2553 = ct{393};
t2555 = ct{394};
t2556 = ct{395};
t2572 = ct{396};
t2575 = ct{397};
t2583 = ct{398};
t2598 = ct{399};
t26 = ct{400};
t2605 = ct{401};
t2606 = ct{402};
t2612 = ct{403};
t2613 = ct{404};
t2615 = ct{405};
t2618 = ct{406};
t2619 = ct{407};
t262 = ct{408};
t2636 = ct{409};
t2638 = ct{410};
t264 = ct{411};
t2651 = ct{412};
t2652 = ct{413};
t2664 = ct{414};
t2670 = ct{415};
t2671 = ct{416};
t2673 = ct{417};
t2674 = ct{418};
t2675 = ct{419};
t2676 = ct{420};
t2678 = ct{421};
t2680 = ct{422};
t2681 = ct{423};
t2682 = ct{424};
t2683 = ct{425};
t2684 = ct{426};
t2685 = ct{427};
t2686 = ct{428};
t2687 = ct{429};
t2689 = ct{430};
t2690 = ct{431};
t2692 = ct{432};
t2693 = ct{433};
t2694 = ct{434};
t2695 = ct{435};
t2696 = ct{436};
t2697 = ct{437};
t2698 = ct{438};
t27 = ct{439};
t2700 = ct{440};
t2701 = ct{441};
t2704 = ct{442};
t2705 = ct{443};
t2707 = ct{444};
t2708 = ct{445};
t2709 = ct{446};
t2711 = ct{447};
t2712 = ct{448};
t2713 = ct{449};
t2715 = ct{450};
t2716 = ct{451};
t2717 = ct{452};
t2719 = ct{453};
t2720 = ct{454};
t2721 = ct{455};
t2732 = ct{456};
t2733 = ct{457};
t2735 = ct{458};
t2736 = ct{459};
t2740 = ct{460};
t2742 = ct{461};
t2743 = ct{462};
t2744 = ct{463};
t2745 = ct{464};
t2747 = ct{465};
t2748 = ct{466};
t2749 = ct{467};
t2750 = ct{468};
t2751 = ct{469};
t2753 = ct{470};
t2754 = ct{471};
t2755 = ct{472};
t2757 = ct{473};
t2759 = ct{474};
t2760 = ct{475};
t2761 = ct{476};
t2763 = ct{477};
t2764 = ct{478};
t2765 = ct{479};
t2766 = ct{480};
t2769 = ct{481};
t2773 = ct{482};
t2774 = ct{483};
t2775 = ct{484};
t2777 = ct{485};
t2778 = ct{486};
t2779 = ct{487};
t2781 = ct{488};
t2785 = ct{489};
t2786 = ct{490};
t2787 = ct{491};
t2788 = ct{492};
t2789 = ct{493};
t2790 = ct{494};
t2791 = ct{495};
t2792 = ct{496};
t2793 = ct{497};
t2794 = ct{498};
t2795 = ct{499};
t2797 = ct{500};
t2798 = ct{501};
t2799 = ct{502};
t28 = ct{503};
t2801 = ct{504};
t2802 = ct{505};
t2803 = ct{506};
t2804 = ct{507};
t2805 = ct{508};
t2807 = ct{509};
t2808 = ct{510};
t2809 = ct{511};
t2813 = ct{512};
t2814 = ct{513};
t2815 = ct{514};
t2817 = ct{515};
t2818 = ct{516};
t2819 = ct{517};
t2820 = ct{518};
t2822 = ct{519};
t2823 = ct{520};
t2828 = ct{521};
t2831 = ct{522};
t2832 = ct{523};
t2834 = ct{524};
t2835 = ct{525};
t2836 = ct{526};
t2837 = ct{527};
t2838 = ct{528};
t2844 = ct{529};
t2850 = ct{530};
t2851 = ct{531};
t2852 = ct{532};
t2853 = ct{533};
t2862 = ct{534};
t2864 = ct{535};
t2889 = ct{536};
t2897 = ct{537};
t2902 = ct{538};
t2904 = ct{539};
t2909 = ct{540};
t2910 = ct{541};
t2921 = ct{542};
t2927 = ct{543};
t2929 = ct{544};
t2932 = ct{545};
t2934 = ct{546};
t2936 = ct{547};
t2937 = ct{548};
t2938 = ct{549};
t2941 = ct{550};
t2942 = ct{551};
t2945 = ct{552};
t2946 = ct{553};
t2947 = ct{554};
t2948 = ct{555};
t2950 = ct{556};
t2951 = ct{557};
t2953 = ct{558};
t2954 = ct{559};
t2955 = ct{560};
t2956 = ct{561};
t2957 = ct{562};
t2961 = ct{563};
t2962 = ct{564};
t2963 = ct{565};
t2964 = ct{566};
t2965 = ct{567};
t2966 = ct{568};
t2969 = ct{569};
t2970 = ct{570};
t2971 = ct{571};
t2972 = ct{572};
t2973 = ct{573};
t2975 = ct{574};
t2976 = ct{575};
t2977 = ct{576};
t2978 = ct{577};
t2979 = ct{578};
t2982 = ct{579};
t2984 = ct{580};
t2985 = ct{581};
t2986 = ct{582};
t2987 = ct{583};
t2990 = ct{584};
t2991 = ct{585};
t2993 = ct{586};
t2994 = ct{587};
t2997 = ct{588};
t2998 = ct{589};
t3 = ct{590};
t30 = ct{591};
t3003 = ct{592};
t3004 = ct{593};
t3006 = ct{594};
t3008 = ct{595};
t3009 = ct{596};
t3010 = ct{597};
t3015 = ct{598};
t3016 = ct{599};
t3017 = ct{600};
t3018 = ct{601};
t3019 = ct{602};
t3020 = ct{603};
t3021 = ct{604};
t3022 = ct{605};
t3027 = ct{606};
t3029 = ct{607};
t3030 = ct{608};
t3031 = ct{609};
t3032 = ct{610};
t3033 = ct{611};
t3034 = ct{612};
t3035 = ct{613};
t3036 = ct{614};
t3040 = ct{615};
t3041 = ct{616};
t3043 = ct{617};
t3044 = ct{618};
t3045 = ct{619};
t3047 = ct{620};
t3049 = ct{621};
t3050 = ct{622};
t3051 = ct{623};
t3054 = ct{624};
t3055 = ct{625};
t3056 = ct{626};
t3057 = ct{627};
t3063 = ct{628};
t3064 = ct{629};
t3065 = ct{630};
t3066 = ct{631};
t3067 = ct{632};
t3068 = ct{633};
t3069 = ct{634};
t3072 = ct{635};
t3073 = ct{636};
t3074 = ct{637};
t3075 = ct{638};
t3076 = ct{639};
t3077 = ct{640};
t3078 = ct{641};
t3079 = ct{642};
t3080 = ct{643};
t3081 = ct{644};
t3082 = ct{645};
t3083 = ct{646};
t3085 = ct{647};
t3086 = ct{648};
t3087 = ct{649};
t3088 = ct{650};
t3089 = ct{651};
t3090 = ct{652};
t3096 = ct{653};
t3097 = ct{654};
t31 = ct{655};
t3109 = ct{656};
t3110 = ct{657};
t3111 = ct{658};
t3113 = ct{659};
t3114 = ct{660};
t3115 = ct{661};
t3116 = ct{662};
t3117 = ct{663};
t3118 = ct{664};
t3119 = ct{665};
t3121 = ct{666};
t3122 = ct{667};
t3128 = ct{668};
t3129 = ct{669};
t313 = ct{670};
t3130 = ct{671};
t3131 = ct{672};
t3132 = ct{673};
t3133 = ct{674};
t3134 = ct{675};
t3135 = ct{676};
t3139 = ct{677};
t314 = ct{678};
t3140 = ct{679};
t3141 = ct{680};
t3142 = ct{681};
t3144 = ct{682};
t3147 = ct{683};
t3149 = ct{684};
t3150 = ct{685};
t3152 = ct{686};
t3153 = ct{687};
t3154 = ct{688};
t3155 = ct{689};
t3156 = ct{690};
t3157 = ct{691};
t3158 = ct{692};
t3159 = ct{693};
t3160 = ct{694};
t3161 = ct{695};
t3162 = ct{696};
t3163 = ct{697};
t3164 = ct{698};
t3165 = ct{699};
t3166 = ct{700};
t3170 = ct{701};
t3171 = ct{702};
t3172 = ct{703};
t3178 = ct{704};
t3179 = ct{705};
t3180 = ct{706};
t3183 = ct{707};
t3184 = ct{708};
t3186 = ct{709};
t3187 = ct{710};
t3188 = ct{711};
t3189 = ct{712};
t3190 = ct{713};
t3191 = ct{714};
t3192 = ct{715};
t3193 = ct{716};
t3194 = ct{717};
t3196 = ct{718};
t3197 = ct{719};
t3198 = ct{720};
t3199 = ct{721};
t32 = ct{722};
t3200 = ct{723};
t3204 = ct{724};
t3205 = ct{725};
t3206 = ct{726};
t3209 = ct{727};
t321 = ct{728};
t3210 = ct{729};
t3211 = ct{730};
t3212 = ct{731};
t3214 = ct{732};
t3215 = ct{733};
t3217 = ct{734};
t3218 = ct{735};
t3219 = ct{736};
t322 = ct{737};
t3220 = ct{738};
t3221 = ct{739};
t3222 = ct{740};
t3223 = ct{741};
t3224 = ct{742};
t3228 = ct{743};
t3229 = ct{744};
t3230 = ct{745};
t3231 = ct{746};
t3232 = ct{747};
t3233 = ct{748};
t3235 = ct{749};
t3236 = ct{750};
t3237 = ct{751};
t3238 = ct{752};
t3239 = ct{753};
t3240 = ct{754};
t3241 = ct{755};
t3243 = ct{756};
t3244 = ct{757};
t3249 = ct{758};
t3250 = ct{759};
t3252 = ct{760};
t3253 = ct{761};
t3254 = ct{762};
t3256 = ct{763};
t3258 = ct{764};
t3259 = ct{765};
t326 = ct{766};
t3260 = ct{767};
t3261 = ct{768};
t3262 = ct{769};
t3263 = ct{770};
t3264 = ct{771};
t3265 = ct{772};
t3266 = ct{773};
t3269 = ct{774};
t3270 = ct{775};
t3271 = ct{776};
t3272 = ct{777};
t3273 = ct{778};
t3274 = ct{779};
t3278 = ct{780};
t3279 = ct{781};
t328 = ct{782};
t3280 = ct{783};
t3283 = ct{784};
t329 = ct{785};
t3296 = ct{786};
t3297 = ct{787};
t3299 = ct{788};
t33 = ct{789};
t330 = ct{790};
t3300 = ct{791};
t3306 = ct{792};
t3308 = ct{793};
t331 = ct{794};
t3311 = ct{795};
t3313 = ct{796};
t3315 = ct{797};
t3316 = ct{798};
t3318 = ct{799};
t3319 = ct{800};
t332 = ct{801};
t3320 = ct{802};
t3321 = ct{803};
t3326 = ct{804};
t3327 = ct{805};
t333 = ct{806};
t3330 = ct{807};
t3333 = ct{808};
t3334 = ct{809};
t3335 = ct{810};
t3341 = ct{811};
t3344 = ct{812};
t3346 = ct{813};
t3347 = ct{814};
t3348 = ct{815};
t3349 = ct{816};
t335 = ct{817};
t3359 = ct{818};
t3360 = ct{819};
t3367 = ct{820};
t3369 = ct{821};
t3370 = ct{822};
t3373 = ct{823};
t3376 = ct{824};
t3377 = ct{825};
t3379 = ct{826};
t338 = ct{827};
t3382 = ct{828};
t3383 = ct{829};
t3384 = ct{830};
t3385 = ct{831};
t3386 = ct{832};
t3387 = ct{833};
t3388 = ct{834};
t3389 = ct{835};
t339 = ct{836};
t3390 = ct{837};
t3391 = ct{838};
t3392 = ct{839};
t3393 = ct{840};
t34 = ct{841};
t3402 = ct{842};
t3403 = ct{843};
t3406 = ct{844};
t3407 = ct{845};
t341 = ct{846};
t3415 = ct{847};
t3417 = ct{848};
t3420 = ct{849};
t3421 = ct{850};
t3422 = ct{851};
t3423 = ct{852};
t3424 = ct{853};
t3425 = ct{854};
t3427 = ct{855};
t3428 = ct{856};
t3429 = ct{857};
t343 = ct{858};
t3430 = ct{859};
t3432 = ct{860};
t3434 = ct{861};
t3435 = ct{862};
t3436 = ct{863};
t3437 = ct{864};
t3438 = ct{865};
t3440 = ct{866};
t3441 = ct{867};
t3442 = ct{868};
t3443 = ct{869};
t3444 = ct{870};
t3445 = ct{871};
t3446 = ct{872};
t3447 = ct{873};
t3449 = ct{874};
t3450 = ct{875};
t3451 = ct{876};
t3452 = ct{877};
t3453 = ct{878};
t3455 = ct{879};
t3456 = ct{880};
t3457 = ct{881};
t3458 = ct{882};
t3459 = ct{883};
t346 = ct{884};
t3460 = ct{885};
t3461 = ct{886};
t3462 = ct{887};
t3463 = ct{888};
t3464 = ct{889};
t3466 = ct{890};
t3468 = ct{891};
t3470 = ct{892};
t3473 = ct{893};
t3474 = ct{894};
t3475 = ct{895};
t3476 = ct{896};
t3478 = ct{897};
t3480 = ct{898};
t3481 = ct{899};
t3489 = ct{900};
t3490 = ct{901};
t3498 = ct{902};
t35 = ct{903};
t350 = ct{904};
t3505 = ct{905};
t351 = ct{906};
t3511 = ct{907};
t3517 = ct{908};
t3519 = ct{909};
t352 = ct{910};
t3520 = ct{911};
t3521 = ct{912};
t3522 = ct{913};
t3524 = ct{914};
t3526 = ct{915};
t3527 = ct{916};
t3533 = ct{917};
t354 = ct{918};
t3540 = ct{919};
t3541 = ct{920};
t3547 = ct{921};
t3558 = ct{922};
t3559 = ct{923};
t356 = ct{924};
t3560 = ct{925};
t3561 = ct{926};
t3566 = ct{927};
t3576 = ct{928};
t3577 = ct{929};
t3578 = ct{930};
t3579 = ct{931};
t358 = ct{932};
t3581 = ct{933};
t3583 = ct{934};
t3584 = ct{935};
t3588 = ct{936};
t359 = ct{937};
t3590 = ct{938};
t36 = ct{939};
t360 = ct{940};
t3607 = ct{941};
t3617 = ct{942};
t362 = ct{943};
t3623 = ct{944};
t3625 = ct{945};
t3627 = ct{946};
t3628 = ct{947};
t363 = ct{948};
t3634 = ct{949};
t364 = ct{950};
t3645 = ct{951};
t365 = ct{952};
t3655 = ct{953};
t366 = ct{954};
t3662 = ct{955};
t3666 = ct{956};
t3669 = ct{957};
t3670 = ct{958};
t3672 = ct{959};
t3673 = ct{960};
t3676 = ct{961};
t3677 = ct{962};
t3678 = ct{963};
t3679 = ct{964};
t3680 = ct{965};
t3681 = ct{966};
t3682 = ct{967};
t3683 = ct{968};
t3684 = ct{969};
t3685 = ct{970};
t3686 = ct{971};
t3687 = ct{972};
t3688 = ct{973};
t3689 = ct{974};
t369 = ct{975};
t370 = ct{976};
t3700 = ct{977};
t3703 = ct{978};
t3704 = ct{979};
t3707 = ct{980};
t371 = ct{981};
t372 = ct{982};
t3732 = ct{983};
t3733 = ct{984};
t3734 = ct{985};
t3735 = ct{986};
t3736 = ct{987};
t3737 = ct{988};
t3738 = ct{989};
t3739 = ct{990};
t3740 = ct{991};
t3741 = ct{992};
t3745 = ct{993};
t3746 = ct{994};
t3747 = ct{995};
t3748 = ct{996};
t3751 = ct{997};
t3752 = ct{998};
t3753 = ct{999};
t3756 = ct{1000};
t3758 = ct{1001};
t3759 = ct{1002};
t3762 = ct{1003};
t3764 = ct{1004};
t3765 = ct{1005};
t3766 = ct{1006};
t3767 = ct{1007};
t3768 = ct{1008};
t3770 = ct{1009};
t3771 = ct{1010};
t3772 = ct{1011};
t3773 = ct{1012};
t3774 = ct{1013};
t3776 = ct{1014};
t3777 = ct{1015};
t3779 = ct{1016};
t378 = ct{1017};
t3782 = ct{1018};
t3783 = ct{1019};
t3784 = ct{1020};
t3785 = ct{1021};
t3786 = ct{1022};
t3787 = ct{1023};
t3788 = ct{1024};
t3789 = ct{1025};
t3790 = ct{1026};
t3792 = ct{1027};
t3793 = ct{1028};
t3795 = ct{1029};
t3798 = ct{1030};
t3799 = ct{1031};
t38 = ct{1032};
t380 = ct{1033};
t3802 = ct{1034};
t3804 = ct{1035};
t3805 = ct{1036};
t3807 = ct{1037};
t3810 = ct{1038};
t3811 = ct{1039};
t3815 = ct{1040};
t3817 = ct{1041};
t3819 = ct{1042};
t382 = ct{1043};
t3822 = ct{1044};
t3823 = ct{1045};
t3826 = ct{1046};
t3827 = ct{1047};
t3828 = ct{1048};
t3832 = ct{1049};
t3833 = ct{1050};
t3834 = ct{1051};
t3836 = ct{1052};
t3842 = ct{1053};
t3843 = ct{1054};
t3844 = ct{1055};
t3845 = ct{1056};
t3847 = ct{1057};
t3849 = ct{1058};
t3850 = ct{1059};
t3852 = ct{1060};
t3853 = ct{1061};
t3854 = ct{1062};
t3855 = ct{1063};
t3856 = ct{1064};
t3862 = ct{1065};
t3863 = ct{1066};
t3864 = ct{1067};
t3865 = ct{1068};
t3866 = ct{1069};
t3867 = ct{1070};
t3869 = ct{1071};
t387 = ct{1072};
t3870 = ct{1073};
t3871 = ct{1074};
t3876 = ct{1075};
t3877 = ct{1076};
t3880 = ct{1077};
t3882 = ct{1078};
t3884 = ct{1079};
t3886 = ct{1080};
t3887 = ct{1081};
t3889 = ct{1082};
t3891 = ct{1083};
t3892 = ct{1084};
t3893 = ct{1085};
t3894 = ct{1086};
t3898 = ct{1087};
t39 = ct{1088};
t3900 = ct{1089};
t3901 = ct{1090};
t3904 = ct{1091};
t3907 = ct{1092};
t3908 = ct{1093};
t3909 = ct{1094};
t3910 = ct{1095};
t3913 = ct{1096};
t3914 = ct{1097};
t3915 = ct{1098};
t3916 = ct{1099};
t3917 = ct{1100};
t3918 = ct{1101};
t3920 = ct{1102};
t3921 = ct{1103};
t3923 = ct{1104};
t3925 = ct{1105};
t3928 = ct{1106};
t3929 = ct{1107};
t3930 = ct{1108};
t3931 = ct{1109};
t3932 = ct{1110};
t3934 = ct{1111};
t3935 = ct{1112};
t3936 = ct{1113};
t3937 = ct{1114};
t3938 = ct{1115};
t3940 = ct{1116};
t3941 = ct{1117};
t3944 = ct{1118};
t3947 = ct{1119};
t3952 = ct{1120};
t3953 = ct{1121};
t3955 = ct{1122};
t3956 = ct{1123};
t3960 = ct{1124};
t3962 = ct{1125};
t3964 = ct{1126};
t3965 = ct{1127};
t3966 = ct{1128};
t3970 = ct{1129};
t3971 = ct{1130};
t3974 = ct{1131};
t3976 = ct{1132};
t3984 = ct{1133};
t3993 = ct{1134};
t3994 = ct{1135};
t3997 = ct{1136};
t3998 = ct{1137};
t4 = ct{1138};
t4000 = ct{1139};
t4002 = ct{1140};
t4003 = ct{1141};
t4004 = ct{1142};
t4005 = ct{1143};
t4012 = ct{1144};
t4019 = ct{1145};
t4099 = ct{1146};
t410 = ct{1147};
t4104 = ct{1148};
t4107 = ct{1149};
t4108 = ct{1150};
t4109 = ct{1151};
t4111 = ct{1152};
t4117 = ct{1153};
t4122 = ct{1154};
t4125 = ct{1155};
t4127 = ct{1156};
t4129 = ct{1157};
t4139 = ct{1158};
t4156 = ct{1159};
t4158 = ct{1160};
t4160 = ct{1161};
t4163 = ct{1162};
t4165 = ct{1163};
t4167 = ct{1164};
t4171 = ct{1165};
t4172 = ct{1166};
t4182 = ct{1167};
t4183 = ct{1168};
t4191 = ct{1169};
t4192 = ct{1170};
t4193 = ct{1171};
t4194 = ct{1172};
t42 = ct{1173};
t4211 = ct{1174};
t4214 = ct{1175};
t4215 = ct{1176};
t4219 = ct{1177};
t4220 = ct{1178};
t4221 = ct{1179};
t4230 = ct{1180};
t4231 = ct{1181};
t4242 = ct{1182};
t4244 = ct{1183};
t4279 = ct{1184};
t4280 = ct{1185};
t4281 = ct{1186};
t4283 = ct{1187};
t429 = ct{1188};
t4295 = ct{1189};
t4299 = ct{1190};
t43 = ct{1191};
t4300 = ct{1192};
t4317 = ct{1193};
t4318 = ct{1194};
t4321 = ct{1195};
t4322 = ct{1196};
t4327 = ct{1197};
t4328 = ct{1198};
t4334 = ct{1199};
t4337 = ct{1200};
t4339 = ct{1201};
t4340 = ct{1202};
t4342 = ct{1203};
t4348 = ct{1204};
t4351 = ct{1205};
t4352 = ct{1206};
t4360 = ct{1207};
t4363 = ct{1208};
t4368 = ct{1209};
t4371 = ct{1210};
t4384 = ct{1211};
t4413 = ct{1212};
t4421 = ct{1213};
t4444 = ct{1214};
t4496 = ct{1215};
t4500 = ct{1216};
t4579 = ct{1217};
t4589 = ct{1218};
t4599 = ct{1219};
t46 = ct{1220};
t4602 = ct{1221};
t4614 = ct{1222};
t4615 = ct{1223};
t4617 = ct{1224};
t4620 = ct{1225};
t4640 = ct{1226};
t4641 = ct{1227};
t4642 = ct{1228};
t4644 = ct{1229};
t4645 = ct{1230};
t4647 = ct{1231};
t4650 = ct{1232};
t4652 = ct{1233};
t4655 = ct{1234};
t4661 = ct{1235};
t4663 = ct{1236};
t4664 = ct{1237};
t4667 = ct{1238};
t4669 = ct{1239};
t4679 = ct{1240};
t4680 = ct{1241};
t4682 = ct{1242};
t4683 = ct{1243};
t4686 = ct{1244};
t4688 = ct{1245};
t4691 = ct{1246};
t4692 = ct{1247};
t4693 = ct{1248};
t4696 = ct{1249};
t4697 = ct{1250};
t4698 = ct{1251};
t4699 = ct{1252};
t47 = ct{1253};
t4701 = ct{1254};
t4702 = ct{1255};
t4703 = ct{1256};
t4704 = ct{1257};
t4705 = ct{1258};
t4742 = ct{1259};
t4758 = ct{1260};
t4772 = ct{1261};
t4779 = ct{1262};
t4789 = ct{1263};
t4792 = ct{1264};
t4816 = ct{1265};
t4822 = ct{1266};
t4823 = ct{1267};
t4826 = ct{1268};
t4829 = ct{1269};
t4842 = ct{1270};
t4860 = ct{1271};
t4865 = ct{1272};
t4868 = ct{1273};
t4869 = ct{1274};
t4870 = ct{1275};
t4871 = ct{1276};
t4898 = ct{1277};
t4911 = ct{1278};
t4931 = ct{1279};
t4964 = ct{1280};
t4965 = ct{1281};
t4974 = ct{1282};
t4976 = ct{1283};
t4985 = ct{1284};
t4986 = ct{1285};
t5 = ct{1286};
t50 = ct{1287};
t5005 = ct{1288};
t5007 = ct{1289};
t5038 = ct{1290};
t5042 = ct{1291};
t5044 = ct{1292};
t5047 = ct{1293};
t5048 = ct{1294};
t5049 = ct{1295};
t5223 = ct{1296};
t5224 = ct{1297};
t5227 = ct{1298};
t523 = ct{1299};
t524 = ct{1300};
t5240 = ct{1301};
t5243 = ct{1302};
t5246 = ct{1303};
t5248 = ct{1304};
t5252 = ct{1305};
t5254 = ct{1306};
t528 = ct{1307};
t530 = ct{1308};
t5306 = ct{1309};
t5308 = ct{1310};
t5316 = ct{1311};
t5317 = ct{1312};
t5320 = ct{1313};
t5328 = ct{1314};
t5337 = ct{1315};
t5338 = ct{1316};
t5339 = ct{1317};
t5340 = ct{1318};
t5342 = ct{1319};
t5344 = ct{1320};
t5345 = ct{1321};
t5346 = ct{1322};
t5347 = ct{1323};
t5348 = ct{1324};
t5349 = ct{1325};
t5350 = ct{1326};
t5377 = ct{1327};
t5379 = ct{1328};
t5380 = ct{1329};
t5381 = ct{1330};
t5383 = ct{1331};
t5384 = ct{1332};
t5388 = ct{1333};
t5389 = ct{1334};
t5399 = ct{1335};
t5402 = ct{1336};
t5403 = ct{1337};
t5405 = ct{1338};
t5407 = ct{1339};
t5411 = ct{1340};
t542 = ct{1341};
t5427 = ct{1342};
t5428 = ct{1343};
t543 = ct{1344};
t5443 = ct{1345};
t5444 = ct{1346};
t5482 = ct{1347};
t5485 = ct{1348};
t5486 = ct{1349};
t5487 = ct{1350};
t5488 = ct{1351};
t549 = ct{1352};
t5490 = ct{1353};
t5491 = ct{1354};
t5492 = ct{1355};
t5493 = ct{1356};
t5494 = ct{1357};
t5496 = ct{1358};
t5498 = ct{1359};
t5500 = ct{1360};
t5510 = ct{1361};
t5517 = ct{1362};
t5518 = ct{1363};
t5524 = ct{1364};
t5531 = ct{1365};
t5552 = ct{1366};
t5578 = ct{1367};
t5580 = ct{1368};
t56 = ct{1369};
t562 = ct{1370};
t5620 = ct{1371};
t5626 = ct{1372};
t5627 = ct{1373};
t563 = ct{1374};
t5631 = ct{1375};
t5694 = ct{1376};
t5695 = ct{1377};
t5722 = ct{1378};
t5723 = ct{1379};
t575 = ct{1380};
t58 = ct{1381};
t5839 = ct{1382};
t5840 = ct{1383};
t587 = ct{1384};
t59 = ct{1385};
t5932 = ct{1386};
t594 = ct{1387};
t5951 = ct{1388};
t5953 = ct{1389};
t5954 = ct{1390};
t6 = ct{1391};
t60 = ct{1392};
t610 = ct{1393};
t6183 = ct{1394};
t6184 = ct{1395};
t6185 = ct{1396};
t6219 = ct{1397};
t628 = ct{1398};
t635 = ct{1399};
t636 = ct{1400};
t638 = ct{1401};
t640 = ct{1402};
t641 = ct{1403};
t642 = ct{1404};
t643 = ct{1405};
t644 = ct{1406};
t645 = ct{1407};
t646 = ct{1408};
t649 = ct{1409};
t654 = ct{1410};
t6543 = ct{1411};
t6544 = ct{1412};
t655 = ct{1413};
t656 = ct{1414};
t657 = ct{1415};
t659 = ct{1416};
t660 = ct{1417};
t663 = ct{1418};
t664 = ct{1419};
t665 = ct{1420};
t6658 = ct{1421};
t666 = ct{1422};
t6663 = ct{1423};
t667 = ct{1424};
t668 = ct{1425};
t669 = ct{1426};
t67 = ct{1427};
t670 = ct{1428};
t672 = ct{1429};
t673 = ct{1430};
t674 = ct{1431};
t675 = ct{1432};
t676 = ct{1433};
t677 = ct{1434};
t678 = ct{1435};
t679 = ct{1436};
t68 = ct{1437};
t681 = ct{1438};
t6811 = ct{1439};
t6812 = ct{1440};
t6813 = ct{1441};
t682 = ct{1442};
t683 = ct{1443};
t684 = ct{1444};
t685 = ct{1445};
t686 = ct{1446};
t687 = ct{1447};
t689 = ct{1448};
t6892 = ct{1449};
t6893 = ct{1450};
t691 = ct{1451};
t692 = ct{1452};
t693 = ct{1453};
t694 = ct{1454};
t7 = ct{1455};
t70 = ct{1456};
t702 = ct{1457};
t707 = ct{1458};
t708 = ct{1459};
t71 = ct{1460};
t710 = ct{1461};
t715 = ct{1462};
t716 = ct{1463};
t717 = ct{1464};
t718 = ct{1465};
t721 = ct{1466};
t722 = ct{1467};
t724 = ct{1468};
t725 = ct{1469};
t73 = ct{1470};
t736 = ct{1471};
t738 = ct{1472};
t740 = ct{1473};
t741 = ct{1474};
t749 = ct{1475};
t756 = ct{1476};
t76 = ct{1477};
t762 = ct{1478};
t768 = ct{1479};
t777 = ct{1480};
t792 = ct{1481};
t793 = ct{1482};
t801 = ct{1483};
t802 = ct{1484};
t808 = ct{1485};
t813 = ct{1486};
t819 = ct{1487};
t821 = ct{1488};
t850 = ct{1489};
t855 = ct{1490};
t874 = ct{1491};
t878 = ct{1492};
t89 = ct{1493};
t90 = ct{1494};
t91 = ct{1495};
t92 = ct{1496};
t941 = ct{1497};
t944 = ct{1498};
t945 = ct{1499};
t948 = ct{1500};
t949 = ct{1501};
t951 = ct{1502};
t97 = ct{1503};
t983 = ct{1504};
t996 = ct{1505};
t4009 = t3908.*1.869599668e-7;
t4023 = t3229.*(t1861-t3214).*(-9.840000000000001e-6);
t4033 = t3229.*(t1861-t3214).*(-6.2e-7);
t4038 = t3229.*(t1861-t3214).*(-3.24e-6);
t4040 = t3229.*(t1861-t3214).*(-7.83e-6);
t4045 = t3229.*(t1861-t3214).*3.24e-6;
t4046 = t3229.*(t1861-t3214).*7.83e-6;
t4048 = t22.*t3229.*(t1861-t3214).*(-5.7e-7);
t4049 = t17.*t3229.*(t1861-t3214).*(-1.02e-6);
t4054 = t22.*t3229.*(t1861-t3214).*5.7e-7;
t4056 = t17.*t3229.*(t1861-t3214).*(-2.4e-7);
t4058 = t17.*t3229.*(t1861-t3214).*(-4.0e-8);
t4060 = t22.*t3229.*(t1861-t3214).*(-4.0e-8);
t4063 = t17.*t3229.*(t1861-t3214).*2.4e-7;
t4080 = t945+t3884;
t4082 = t949+t3886;
t4093 = -t17.*(t944-t3886);
t4095 = -t22.*(t944-t3886);
t4102 = t17.*(t944-t3886);
t4106 = t22.*(t944-t3886).*(-3.0./5.0e+2);
t4110 = t1023+t3908;
t4113 = t1045+t3907;
t4126 = t27.*(t3908-(t262.*(t46-t47))./9.007199254740992e+15);
t4128 = t33.*(t3908-(t262.*(t46-t47))./9.007199254740992e+15);
t4134 = t549+t1874+t1882+t1890+t1911+t2755+t2794;
t4137 = -t4127;
t4143 = t4117.*(3.0./5.0e+2);
t4149 = t2818+t2819+t3115+t3116;
t4164 = t22.*(t944-t3886).*(-5.68686e-3);
t4170 = t22.*(t944-t3886).*(-3.131399999999998e-4);
t4173 = t188.*t3901.*(t42-t43).*(-2.442490654175345e-23);
t4174 = t188.*t3901.*(t42-t43).*2.442490654175345e-23;
t4175 = t587+t1879+t1923+t1931+t1963+t2844+t2910;
t4177 = t4127.*1.247162e-2;
t4186 = t4117.*3.131399999999998e-4;
t4188 = t4117.*4.36041e-5;
t4195 = -t4193;
t4197 = -t3468.*(t1896-t3232);
t4205 = t4117.*6.1855407534e-5;
t4207 = t4127.*1.35652563578e-4;
t4216 = t50.*t189.*t3901.*(t42-t43).*(-2.711709361697228e-39);
t4218 = t50.*t189.*t3901.*(t42-t43).*2.711709361697228e-39;
t4235 = ((t1861-t3214).*(t1896-t3232))./1.0e+8;
t4251 = (t1861-t3214).*(t1896-t3232).*6.2e-7;
t4253 = t22.*(t1861-t3214).*(t1896-t3232).*5.7e-7;
t4254 = t17.*(t1861-t3214).*(t1896-t3232).*1.02e-6;
t4257 = t17.*(t1861-t3214).*(t1896-t3232).*2.4e-7;
t4258 = t17.*(t1861-t3214).*(t1896-t3232).*4.0e-8;
t4259 = t22.*(t1861-t3214).*(t1896-t3232).*4.0e-8;
t4284 = t2973.*(t3908-(t262.*(t46-t47))./9.007199254740992e+15);
t4302 = t1889+t1948+t2766+t2815+t3089+t3090;
t4312 = t2961+t3517+t3520;
t4323 = t1930+t1971+t2862+t2932+t3110+t3111;
t4329 = t3230.*(-t1901+t3122+t3270).*(-3.24e-6);
t4330 = t3230.*(-t1901+t3122+t3270).*(-3.11e-6);
t4333 = t3210.*t3901.*1.1e-7;
t4336 = t3210.*t3901.*3.24e-6;
t4338 = t3210.*t3901.*3.11e-6;
t4344 = t3210.*t3904.*3.11e-6;
t4346 = t3210.*t3904.*3.24e-6;
t4347 = t3210.*t3901.*5.0e-8;
t4349 = t3211.*t3901.*5.0e-8;
t4350 = t3211.*t3901.*1.6e-7;
t4362 = -t3142.*(-t2804+t2838+t3109+t23.*(t1456-t2355).*9.3e-7);
t4364 = t3142.*(-t2804+t2838+t3109+t23.*(t1456-t2355).*9.3e-7);
t4365 = t530+t1918+t2743+t2751+t2761+t2763+t2764+t2793;
t4399 = t563+t1964+t2832+t2836+t2853+t2889+t2897+t2909;
t4404 = t3209.*t4108;
t4405 = t3210.*t4108;
t4412 = t3230.*(t951+t16.*(-t1881+t3121+t3269)).*(-1.0e-8);
t4415 = t3229.*(t944-t3886).*(-9.840000000000001e-6);
t4416 = t3230.*((t237.*(t42-t43))./9.007199254740992e+15+t21.*(-t1881+t3121+t3269)).*(-9.840000000000001e-6);
t4417 = t3229.*(t944-t3886).*9.840000000000001e-6;
t4425 = t3230.*(t951+t16.*(-t1881+t3121+t3269)).*(-3.24e-6);
t4426 = t3230.*(t951+t16.*(-t1881+t3121+t3269)).*(-7.83e-6);
t4427 = t3230.*(t951+t16.*(-t1881+t3121+t3269)).*(-6.2e-7);
t4429 = (t2527-t3009).*(-t2804+t2838+t3109+t23.*(t1456-t2355).*9.3e-7);
t4432 = t188.*t4384.*8.595599785252598e-1;
t4433 = t1526+t1900+t2553+t2817+t2837+t3113+t3114;
t4437 = ((t1861-t3214).*(t2694-t2701+t3036-t3043))./1.0e+8;
t4439 = ((t1861-t3214).*(t1959-t3306+t38.*t1022.*(t855-t878).*2.196325630278387e-1))./1.0e+8;
t4447 = t3385.*t4122;
t4448 = -t3385.*(-t2804+t2838+t3109+t23.*(t1456-t2355).*9.3e-7);
t4449 = -t3385.*(t2813-t2835+t18.*(t1456-t2355).*1.02e-6+t23.*(t1456-t2355).*9.0e-8);
t4450 = (t1861-t3214).*(t2694-t2701+t3036-t3043).*9.840000000000001e-6;
t4455 = -t3386.*(-t2804+t2838+t3109+t23.*(t1456-t2355).*9.3e-7);
t4457 = -t3386.*(t2813-t2835+t18.*(t1456-t2355).*1.02e-6+t23.*(t1456-t2355).*9.0e-8);
t4458 = t3386.*t4125;
t4460 = (t1861-t3214).*(t2694-t2701+t3036-t3043).*6.2e-7;
t4462 = (t1861-t3214).*(t2694-t2701+t3036-t3043).*3.24e-6;
t4463 = (t1861-t3214).*(t2694-t2701+t3036-t3043).*7.83e-6;
t4467 = t3386.*(t2813-t2835+t18.*(t1456-t2355).*1.02e-6+t23.*(t1456-t2355).*9.0e-8);
t4471 = (t1861-t3214).*(t1959-t3306+t38.*t1022.*(t855-t878).*2.196325630278387e-1).*7.83e-6;
t4473 = (t1861-t3214).*(t1959-t3306+t38.*t1022.*(t855-t878).*2.196325630278387e-1).*6.2e-7;
t4474 = t22.*(t1861-t3214).*(t2694-t2701+t3036-t3043).*5.7e-7;
t4476 = t17.*(t1861-t3214).*(t2694-t2701+t3036-t3043).*1.02e-6;
t4479 = (t1861-t3214).*(t1959-t3306+t38.*t1022.*(t855-t878).*2.196325630278387e-1).*3.24e-6;
t4483 = t17.*(t1861-t3214).*(t2694-t2701+t3036-t3043).*2.4e-7;
t4484 = t17.*(t1861-t3214).*(t2694-t2701+t3036-t3043).*4.0e-8;
t4485 = t22.*(t1861-t3214).*(t2694-t2701+t3036-t3043).*4.0e-8;
t4574 = -t3468.*(t1005+t26.*(t1941-t3308+t39.*t1022.*(t855-t878).*2.196325630278387e-1));
t4587 = -t4108.*(t1861-t3214);
t4594 = ((t1005+t26.*(t1941-t3308+t39.*t1022.*(t855-t878).*2.196325630278387e-1)).*(t1861-t3214))./1.0e+8;
t4607 = (t1005+t26.*(t1941-t3308+t39.*t1022.*(t855-t878).*2.196325630278387e-1)).*(t1861-t3214).*6.2e-7;
t4687 = t3901.*(-t1901+t3122+t3270).*(-1.1e-7);
t4689 = t3901.*(-t1901+t3122+t3270).*(-3.24e-6);
t4690 = t3901.*(-t1881+t3121+t3269).*(-5.0e-8);
t4694 = t3901.*(-t1881+t3121+t3269).*(-1.6e-7);
t4695 = t3901.*(-t1901+t3122+t3270).*(-3.11e-6);
t4700 = t3901.*(-t1901+t3122+t3270).*(-5.0e-8);
t4707 = t524+t575+t1488+t1870+t1886+t1957+t2519+t2740+t2747+t3096+t3097;
t4776 = t543+t610+t1513+t1876+t1927+t1998+t2598+t2820+t2834+t3117+t3118;
t4783 = t18.*t4779;
t4784 = t23.*t4779;
t4791 = t3901.*(t951+t16.*(-t1881+t3121+t3269)).*(-1.0e-8);
t4795 = t587+t1931+t1963+t2004+t2817+t2837+t2844+t2934+t3113+t3114;
t4817 = t3914+t4117;
t4820 = t3901.*((t237.*(t42-t43))./9.007199254740992e+15+t21.*(-t1881+t3121+t3269)).*(-9.840000000000001e-6);
t4821 = (t944-t3886).*(t2694-t2701+t3036-t3043).*9.840000000000001e-6;
t4837 = t3901.*(t951+t16.*(-t1881+t3121+t3269)).*(-3.24e-6);
t4838 = t3901.*(t951+t16.*(-t1881+t3121+t3269)).*(-7.83e-6);
t4839 = t3901.*(t951+t16.*(-t1881+t3121+t3269)).*(-6.2e-7);
t4963 = t50.*t189.*t4898.*9.543032792050485e-17;
t4966 = -t4965;
t5001 = -t3132.*(t4127+t33.*(t1959-t3306+t38.*t1022.*(t855-t878).*2.196325630278387e-1));
t5002 = t3132.*(t4127+t33.*(t1959-t3306+t38.*t1022.*(t855-t878).*2.196325630278387e-1));
t5009 = t3230.*(t17.*((t237.*(t42-t43))./9.007199254740992e+15+t21.*(-t1881+t3121+t3269))+t22.*(-t1901+t3122+t3270)).*(-1.0e-8);
t5010 = (t3230.*(t17.*((t237.*(t42-t43))./9.007199254740992e+15+t21.*(-t1881+t3121+t3269))+t22.*(-t1901+t3122+t3270)))./1.0e+8;
t5016 = t3230.*(t17.*((t237.*(t42-t43))./9.007199254740992e+15+t21.*(-t1881+t3121+t3269))+t22.*(-t1901+t3122+t3270)).*(-1.02e-6);
t5017 = t3230.*(t17.*((t237.*(t42-t43))./9.007199254740992e+15+t21.*(-t1881+t3121+t3269))+t22.*(-t1901+t3122+t3270)).*1.02e-6;
t5019 = t3230.*(t17.*((t237.*(t42-t43))./9.007199254740992e+15+t21.*(-t1881+t3121+t3269))+t22.*(-t1901+t3122+t3270)).*(-2.4e-7);
t5021 = t3230.*t4779.*5.7e-7;
t5023 = t3230.*(t17.*((t237.*(t42-t43))./9.007199254740992e+15+t21.*(-t1881+t3121+t3269))+t22.*(-t1901+t3122+t3270)).*2.4e-7;
t5026 = t3230.*(t17.*((t237.*(t42-t43))./9.007199254740992e+15+t21.*(-t1881+t3121+t3269))+t22.*(-t1901+t3122+t3270)).*(-4.0e-8);
t5029 = t3230.*t4779.*4.0e-8;
t5035 = t3210.*t4860.*1.1e-7;
t5036 = t3210.*t4860.*3.24e-6;
t5037 = t3210.*t4860.*3.11e-6;
t5039 = t3210.*t4860.*5.0e-8;
t5040 = t3211.*t4860.*5.0e-8;
t5041 = t3211.*t4860.*1.6e-7;
t5043 = -t5038;
t5045 = -t5042;
t5046 = -t5044;
t5050 = -t5048;
t5061 = -t4758.*(t1861-t3214);
t5153 = t4865.*(t1861-t3214).*(-1.0e-8);
t5167 = t4865.*(t1861-t3214).*(-3.24e-6);
t5168 = t4865.*(t1861-t3214).*(-7.83e-6);
t5169 = t4865.*(t1861-t3214).*(-6.2e-7);
t5191 = t3183+t3192+t3311+t3315+t3460+t3474;
t5219 = t3901.*(t17.*((t237.*(t42-t43))./9.007199254740992e+15+t21.*(-t1881+t3121+t3269))+t22.*(-t1901+t3122+t3270)).*(-1.0e-8);
t5221 = (t3901.*(t17.*((t237.*(t42-t43))./9.007199254740992e+15+t21.*(-t1881+t3121+t3269))+t22.*(-t1901+t3122+t3270)))./1.0e+8;
t5229 = t3901.*(t17.*((t237.*(t42-t43))./9.007199254740992e+15+t21.*(-t1881+t3121+t3269))+t22.*(-t1901+t3122+t3270)).*(-1.02e-6);
t5230 = t3901.*(t17.*((t237.*(t42-t43))./9.007199254740992e+15+t21.*(-t1881+t3121+t3269))+t22.*(-t1901+t3122+t3270)).*(-2.4e-7);
t5231 = t3901.*t4779.*5.7e-7;
t5233 = t3901.*(t17.*((t237.*(t42-t43))./9.007199254740992e+15+t21.*(-t1881+t3121+t3269))+t22.*(-t1901+t3122+t3270)).*2.4e-7;
t5235 = t3901.*(t17.*((t237.*(t42-t43))./9.007199254740992e+15+t21.*(-t1881+t3121+t3269))+t22.*(-t1901+t3122+t3270)).*(-4.0e-8);
t5239 = t3901.*(t17.*((t237.*(t42-t43))./9.007199254740992e+15+t21.*(-t1881+t3121+t3269))+t22.*(-t1901+t3122+t3270)).*4.0e-8;
t5241 = t3901.*t4779.*4.0e-8;
t5245 = t3359.*t3617.*t3877.*t3901.*2.889644e-2;
t5247 = t3313.*t3628.*t3877.*t3901.*2.889644e-2;
t5256 = -t4758.*(t951+t16.*(-t1881+t3121+t3269));
t5257 = t4758.*(t951+t16.*(-t1881+t3121+t3269));
t5425 = t2507+t2517+t3462+t3463+t4192+t4194;
t5702 = t3877.*t3901.*t4108.*(t1513+t1879+t2598+t2820+t2834+t3117+t3118).*(-7.26735e-3);
t5703 = t4108.*(t2674-t2676+t3022-t3027).*(t2694-t2701+t3036-t3043).*(t1513+t1879+t2598+t2820+t2834+t3117+t3118).*(-7.26735e-3);
et38 = t2500-t2507-t3462-t3463+t50.*t189.*(t1941-t3308+t39.*t1022.*(t855-t878).*2.196325630278387e-1).*4.306286555174926e-24;
et39 = t50.*t189.*(t1959-t3306+t38.*t1022.*(t855-t878).*2.196325630278387e-1).*7.660522649005482e-24;
t5719 = (et38+et39).*(t2674-t2676+t3022-t3027);
t5835 = t3628.*t3901.*t5510.*2.889644e-2;
t5942 = t1558+t2385+t2386+t2393+t2396+t3923+t3930+t3931+t4156+t4167;
et40 = t707+t708-t721-t722-t749+t762+t768-t777-t792-t793-t801-t802-t808+t813-t819+t821-t1629+t1637-t1640-t1641-t1659-t1661+t1666+t1667+t1683+t1692+t1705-t1712+t1758+t1759+t1775+t1776+t1973+t1993+t1994+t2023+t2053+t2060-t2089-t2090+t2098+t2099-t14.*t15.*t21.*t50.*t189.*3.670836568391568e-22;
et41 = t16.*t19.*t20.*t50.*t189.*(-3.279367663374749e-19)-t14.*t15.*t17.*t21.*t50.*t189.*7.075931802640439e-19;
et42 = t14.*t17.*t20.*t21.*t50.*t189.*(-1.190170786299927e-18)-t15.*t17.*t19.*t21.*t50.*t189.*1.190170786299927e-18;
et43 = t19.*t20.*t21.*t22.*t50.*t189.*(-3.226512155691387e-19);
t6220 = t3732.*t3901.*(et40+et41+et42+et43).*(-1.08769e-2);
et44 = t707+t708-t721-t722-t749+t762+t768-t777-t792-t793-t801-t802-t808+t813-t819+t821-t1629+t1637-t1640-t1641-t1659-t1661+t1666+t1667+t1683+t1692+t1705-t1712+t1758+t1759+t1775+t1776+t1973+t1993+t1994+t2023+t2053+t2060-t2089-t2090+t2098+t2099-t14.*t15.*t21.*t50.*t189.*3.670836568391568e-22;
et45 = t16.*t19.*t20.*t50.*t189.*(-3.279367663374749e-19)-t14.*t15.*t17.*t21.*t50.*t189.*7.075931802640439e-19;
et46 = t14.*t17.*t20.*t21.*t50.*t189.*(-1.190170786299927e-18)-t15.*t17.*t19.*t21.*t50.*t189.*1.190170786299927e-18;
et47 = t19.*t20.*t21.*t22.*t50.*t189.*(-3.226512155691387e-19);
t6221 = t3732.*t3901.*(et44+et45+et46+et47).*1.08769e-2;
t6247 = t3784.*t5951.*(t2694-t2701+t3036-t3043).*(-1.08769e-2);
et48 = t707+t708-t721-t722-t749+t762+t768-t777-t792-t793-t801-t802-t808+t813-t819+t821-t1629+t1637-t1640-t1641-t1659-t1661+t1666+t1667+t1683+t1692+t1705-t1712+t1758+t1759+t1775+t1776+t1973+t1993+t1994+t2023+t2053+t2060-t2089-t2090+t2098+t2099-t14.*t15.*t21.*t50.*t189.*3.670836568391568e-22;
et49 = t16.*t19.*t20.*t50.*t189.*(-3.279367663374749e-19)-t14.*t15.*t17.*t21.*t50.*t189.*7.075931802640439e-19;
et50 = t14.*t17.*t20.*t21.*t50.*t189.*(-1.190170786299927e-18)-t15.*t17.*t19.*t21.*t50.*t189.*1.190170786299927e-18;
et51 = t19.*t20.*t21.*t22.*t50.*t189.*(-3.226512155691387e-19);
t6253 = t3784.*t3901.*(et48+et49+et50+et51).*(-1.08769e-2);
t6484 = -t3782.*t6183.*(t2674-t2676+t3022-t3027);
et52 = t1288+t1289+t1302+t1303-t1319-t1320+t1336-t1348+t1350+t1351-t1360+t1369-t1378+t1396-t1425+t1435-t2174+t2183-t2187+t2193-t2194-t2195+t2199-t2203-t2215+t2219-t2222-t2223+t2239+t2240-t2256-t2257+t2555+t2556+t2572+t2583-t2605-t2606+t2612+t2613-t2618-t2619+t2651+t2652;
et53 = t24.*t25.*t26.*t50.*t202.*(-3.566935413776081e-21);
et54 = t30.*t31.*t32.*t50.*t202.*(-3.992732227073824e-24);
et55 = t24.*t25.*t32.*t33.*t50.*t202.*(-3.509445006623964e-21);
et56 = t27.*t30.*t31.*t32.*t50.*t202.*(-7.696420262413979e-21);
t6485 = -t3782.*t3877.*(et52+et53+et54+et55+et56);
et57 = t1288+t1289+t1302+t1303-t1319-t1320+t1336-t1348+t1350+t1351-t1360+t1369-t1378+t1396-t1425+t1435-t2174+t2183-t2187+t2193-t2194-t2195+t2199-t2203-t2215+t2219-t2222-t2223+t2239+t2240-t2256-t2257+t2555+t2556+t2572+t2583-t2605-t2606+t2612+t2613-t2618-t2619+t2651+t2652;
et58 = t24.*t25.*t26.*t50.*t202.*(-3.566935413776081e-21);
et59 = t30.*t31.*t32.*t50.*t202.*(-3.992732227073824e-24);
et60 = t24.*t25.*t32.*t33.*t50.*t202.*(-3.509445006623964e-21);
et61 = t27.*t30.*t31.*t32.*t50.*t202.*(-7.696420262413979e-21);
t6486 = t3782.*t3877.*(et57+et58+et59+et60+et61);
et62 = t1288+t1289+t1302+t1303-t1319-t1320+t1336-t1348+t1350+t1351-t1360+t1369-t1378+t1396-t1425+t1435-t2174+t2183-t2187+t2193-t2194-t2195+t2199-t2203-t2215+t2219-t2222-t2223+t2239+t2240-t2256-t2257+t2555+t2556+t2572+t2583-t2605-t2606+t2612+t2613-t2618-t2619+t2651+t2652;
et63 = t24.*t25.*t26.*t50.*t202.*(-3.566935413776081e-21);
et64 = t30.*t31.*t32.*t50.*t202.*(-3.992732227073824e-24);
et65 = t24.*t25.*t32.*t33.*t50.*t202.*(-3.509445006623964e-21);
et66 = t27.*t30.*t31.*t32.*t50.*t202.*(-7.696420262413979e-21);
t7041 = (et62+et63+et64+et65+et66).*(t1554+t2361+t2362+t2367+t2414+t3928+t3934+t4160+t4163+t17.*(-t1901+t3122+t3270).*5.68686e-3);
t3201 = -t3199;
t3225 = t3220.*(3.0./5.0e+2);
t3226 = -t3223;
t3227 = t3222.*(3.0./5.0e+2);
t3242 = t2410+t2997;
t3245 = t3238.*(3.0./5.0e+2);
t3246 = -t3243;
t3247 = t3240.*(3.0./5.0e+2);
t3248 = -t3244;
t3275 = t3220.*1.247162e-2;
t3276 = t3222.*1.247162e-2;
t3277 = -t3272;
t3281 = -t3273;
t3282 = t3219.*5.84482e-3;
t3284 = -t3274;
t3285 = t3221.*5.84482e-3;
t3287 = t3220.*5.68686e-3;
t3288 = t3222.*5.68686e-3;
t3289 = -t3279;
t3290 = -t3280;
t3291 = t3219.*6.48e-5;
t3293 = -t3283;
t3294 = t3221.*6.48e-5;
t3301 = t3220.*3.131399999999998e-4;
t3302 = t3222.*3.131399999999998e-4;
t3303 = -t3299;
t3304 = t3219.*6.47e-6;
t3305 = t3221.*6.47e-6;
t3322 = t3238.*1.247162e-2;
t3323 = -t3318;
t3324 = t3240.*1.247162e-2;
t3325 = -t3319;
t3328 = -t3320;
t3329 = t3237.*5.84482e-3;
t3331 = -t3321;
t3332 = t3239.*5.84482e-3;
t3336 = t3237.*6.48e-5;
t3338 = -t3330;
t3339 = t3239.*6.48e-5;
t3342 = t3240.*3.131399999999998e-4;
t3343 = -t3334;
t3350 = t3238.*3.131399999999998e-4;
t3351 = -t3346;
t3352 = t3237.*6.47e-6;
t3353 = t3239.*6.47e-6;
t3354 = t3238.*4.36041e-5;
t3355 = t3240.*4.36041e-5;
t3356 = -t3349;
t3394 = t3238.*1.35652563578e-4;
t3395 = t3240.*1.35652563578e-4;
t3396 = -t3390;
t3397 = t3237.*1.688944904408e-4;
t3398 = t3239.*1.688944904408e-4;
t3399 = t3238.*6.1855407534e-5;
t3400 = t3240.*6.1855407534e-5;
t3401 = -t3393;
t3408 = -t3402;
t3409 = t3237.*7.0482312e-7;
t3410 = t3239.*7.0482312e-7;
t3411 = t3237.*1.869599668e-7;
t3412 = t3239.*1.869599668e-7;
t3419 = -t3417;
t3433 = -t3425;
t3465 = -t3461;
t3467 = -t3466;
t3477 = -t3476;
t3479 = -t3478;
t3483 = t1865+t3219;
t3484 = t1868+t3221;
t3485 = t17.*t3481;
t3486 = t18.*t3481;
t3487 = t22.*t3481;
t3488 = t23.*t3481;
t3494 = t22.*t3489;
t3495 = t22.*t3490;
t3523 = -t3521;
t3528 = t1913+t3237;
t3529 = t50.*t202.*t3236.*9.733893447891495e-23;
t3531 = t1933+t3239;
t3534 = t50.*t202.*t3236.*8.588729512845436e-24;
t3535 = t27.*t3524;
t3536 = t28.*t3524;
t3537 = t33.*t3524;
t3538 = t34.*t3524;
t3551 = t33.*t3540;
t3552 = t33.*t3541;
t3563 = t33.*t3547;
t3595 = t22.*t3577;
t3598 = t3505.*(-1.838876e-2);
t3622 = t3547.*(-9.99471e-3);
t3624 = t3547.*(-1.838876e-2);
t3630 = t3547.*9.99471e-3;
t3647 = t33.*t3623;
t3659 = t3057.*t3063;
t3665 = -t3662;
t3667 = -t3666;
t3674 = -t3672;
t3690 = t2363.*t3236.*1.02e-6;
t3699 = t3547.*(-1.33637554986e-4);
t3702 = t3547.*(-7.26350557185e-5);
t3705 = t2363.*t3236.*9.0e-8;
t3711 = t3547.*7.26350557185e-5;
t3725 = t33.*t3703;
t3743 = t2363.*t3420;
t3749 = -t3747;
t3755 = t27.*t3745;
t3757 = -t3752;
t3760 = -t3756;
t3763 = t27.*t3748;
t3769 = -t3765;
t3775 = -t3773;
t3778 = -t3777;
t3791 = -t3787;
t3794 = -t3792;
t3796 = t3057.*t3236.*1.02e-6;
t3800 = t3057.*t3236.*9.0e-8;
t3812 = t2971.*t3524;
t3813 = t2972.*t3524;
t3814 = -t3810;
t3816 = -t3811;
t3818 = t2973.*t3524;
t3821 = -t3817;
t3858 = t33.*t2363.*t3789;
t3859 = -t3856;
t3872 = -t3688.*(t1477-t2502);
t3873 = t3688.*(t1477-t2502);
t3895 = t3154.*t3524;
t3919 = t2998.*t3789;
t3926 = -t3920;
t3927 = -t3921;
t3933 = -t3925;
t3939 = -t3936;
t3943 = t2904+t2929+t3033+t3034;
t3945 = t2864+t2938+t3032+t3035;
t3949 = -t3944;
t3954 = -t3947;
t3958 = -t3952;
t3975 = (t3229.*t3481)./1.0e+8;
t3978 = t17.*t3976;
t3987 = t3057.*t3789;
t3989 = -t3789.*(t1477-t2502);
t3995 = t3789.*(t1477-t2502);
t4001 = -t3997;
t4020 = t3229.*t3481.*9.840000000000001e-6;
t4028 = t3229.*t3481.*6.2e-7;
t4029 = t3229.*t3481.*3.24e-6;
t4030 = t3229.*t3481.*7.83e-6;
t4087 = t18.*t4080;
t4088 = t23.*t4080;
t4131 = t28.*t4113;
t4133 = t34.*t4113;
t4138 = -t4128;
t4144 = t4128.*(3.0./5.0e+2);
t4154 = t27.*t2363.*t3863;
t4157 = t4102.*(-1.247162e-2);
t4162 = t4102.*1.247162e-2;
t4166 = -t3420.*(t1896-t3232);
t4176 = t4126.*1.247162e-2;
t4185 = t4128.*3.131399999999998e-4;
t4187 = t4128.*4.36041e-5;
t4196 = t3468.*t3524;
t4198 = t3057.*t3843;
t4204 = t4128.*6.1855407534e-5;
t4206 = t4126.*1.35652563578e-4;
t4212 = -t4207;
t4225 = t3385.*t3736;
t4228 = t3386.*t3737;
t4233 = t3481.*(t1896-t3232).*(-1.0e-8);
t4234 = t3524.*(t1861-t3214).*(-1.0e-8);
t4236 = t17.*t4235;
t4241 = t3003.*t3863;
t4249 = t3481.*(t1896-t3232).*(-6.2e-7);
t4250 = t3524.*(t1861-t3214).*(-6.2e-7);
t4262 = -t4258;
t4263 = -t4259;
t4272 = t3057.*t3863;
t4273 = -t3863.*(t1477-t2502);
t4277 = t2290+t2312+t3274+t3299;
t4285 = -t33.*t3789.*(t1896-t3232);
t4286 = -t4284;
t4288 = t33.*t3789.*(t1896-t3232);
t4290 = t3385.*t3844;
t4292 = t3386.*t3845;
t4298 = t528+t1000+t2523+t2789+t2809+t3020+t3021;
t4304 = t562+t1003+t2636+t2902+t2921+t3040+t3041;
t4308 = t3209.*t3892;
t4310 = t3210.*t3892;
t4324 = t2732+t2791+t3391+t3406;
t4355 = t3229.*t3918.*7.26735e-3;
t4356 = t3230.*t3918.*7.26735e-3;
t4366 = t523+t594+t1905+t1954+t3941;
t4367 = t3154.*t4113;
t4401 = t542+t644+t1945+t1992+t3984;
t4407 = -t27.*t3863.*(t1896-t3232);
t4408 = (t3229.*t4080)./1.0e+8;
t4418 = t3229.*t4080.*3.24e-6;
t4419 = t3229.*t4080.*7.83e-6;
t4420 = t3229.*t4080.*6.2e-7;
t4428 = -t3250.*(t2813-t2835+t18.*(t1456-t2355).*1.02e-6+t23.*(t1456-t2355).*9.0e-8);
t4430 = t3250.*(t2813-t2835+t18.*(t1456-t2355).*1.02e-6+t23.*(t1456-t2355).*9.0e-8);
t4431 = -t4429;
t4434 = t3229.*t4149.*7.26735e-3;
t4435 = t3481.*(t2694-t2701+t3036-t3043).*(-1.0e-8);
t4436 = t3230.*t4149.*7.26735e-3;
t4441 = t17.*t4437;
t4446 = t3481.*(t2694-t2701+t3036-t3043).*(-9.840000000000001e-6);
t4451 = t3481.*(t1959-t3306+t38.*t1022.*(t855-t878).*2.196325630278387e-1).*(-9.840000000000001e-6);
t4453 = t3481.*(t2694-t2701+t3036-t3043).*(-6.2e-7);
t4454 = t3481.*(t2694-t2701+t3036-t3043).*(-3.24e-6);
t4456 = t3481.*(t2694-t2701+t3036-t3043).*(-7.83e-6);
t4468 = -t4458;
t4480 = -t4474;
t4489 = -t4485;
